simulink model "SimulinkAnalysisofCheetahTail"  (R2022a)
(part 6 of 21)

t4052 = ct{1961};
t4053 = ct{1962};
t4054 = ct{1963};
t4056 = ct{1964};
t4058 = ct{1965};
t4059 = ct{1966};
t4061 = ct{1967};
t4062 = ct{1968};
t4064 = ct{1969};
t4065 = ct{1970};
t4066 = ct{1971};
t4068 = ct{1972};
t4070 = ct{1973};
t4071 = ct{1974};
t4072 = ct{1975};
t4073 = ct{1976};
t4074 = ct{1977};
t4077 = ct{1978};
t4078 = ct{1979};
t4081 = ct{1980};
t4083 = ct{1981};
t4084 = ct{1982};
t4085 = ct{1983};
t4086 = ct{1984};
t4087 = ct{1985};
t4089 = ct{1986};
t4090 = ct{1987};
t4091 = ct{1988};
t4092 = ct{1989};
t4093 = ct{1990};
t4094 = ct{1991};
t4095 = ct{1992};
t4096 = ct{1993};
t4097 = ct{1994};
t4098 = ct{1995};
t4099 = ct{1996};
t410 = ct{1997};
t4100 = ct{1998};
t4104 = ct{1999};
t4105 = ct{2000};
t4107 = ct{2001};
t4108 = ct{2002};
t4109 = ct{2003};
t411 = ct{2004};
t4111 = ct{2005};
t4112 = ct{2006};
t4115 = ct{2007};
t4116 = ct{2008};
t4117 = ct{2009};
t4119 = ct{2010};
t412 = ct{2011};
t4120 = ct{2012};
t4121 = ct{2013};
t4122 = ct{2014};
t4126 = ct{2015};
t4128 = ct{2016};
t4129 = ct{2017};
t413 = ct{2018};
t4130 = ct{2019};
t4131 = ct{2020};
t4132 = ct{2021};
t4133 = ct{2022};
t4135 = ct{2023};
t4137 = ct{2024};
t4138 = ct{2025};
t4139 = ct{2026};
t414 = ct{2027};
t4140 = ct{2028};
t4141 = ct{2029};
t4143 = ct{2030};
t4144 = ct{2031};
t4145 = ct{2032};
t4147 = ct{2033};
t4148 = ct{2034};
t415 = ct{2035};
t4151 = ct{2036};
t4152 = ct{2037};
t4153 = ct{2038};
t4154 = ct{2039};
t4155 = ct{2040};
t4156 = ct{2041};
t4157 = ct{2042};
t4158 = ct{2043};
t4160 = ct{2044};
t4162 = ct{2045};
t4164 = ct{2046};
t4165 = ct{2047};
t4166 = ct{2048};
t4168 = ct{2049};
t4169 = ct{2050};
t4170 = ct{2051};
t4171 = ct{2052};
t4173 = ct{2053};
t4174 = ct{2054};
t4176 = ct{2055};
t4177 = ct{2056};
t4178 = ct{2057};
t4179 = ct{2058};
t4182 = ct{2059};
t4184 = ct{2060};
t4186 = ct{2061};
t4187 = ct{2062};
t4188 = ct{2063};
t4189 = ct{2064};
t4190 = ct{2065};
t4191 = ct{2066};
t4192 = ct{2067};
t4193 = ct{2068};
t4194 = ct{2069};
t4195 = ct{2070};
t4196 = ct{2071};
t4197 = ct{2072};
t420 = ct{2073};
t4200 = ct{2074};
t4201 = ct{2075};
t4202 = ct{2076};
t4203 = ct{2077};
t4204 = ct{2078};
t4205 = ct{2079};
t4206 = ct{2080};
t4208 = ct{2081};
t4209 = ct{2082};
t421 = ct{2083};
t4210 = ct{2084};
t4211 = ct{2085};
t4212 = ct{2086};
t4213 = ct{2087};
t4214 = ct{2088};
t4215 = ct{2089};
t4216 = ct{2090};
t4217 = ct{2091};
t4218 = ct{2092};
t4220 = ct{2093};
t4221 = ct{2094};
t4222 = ct{2095};
t4223 = ct{2096};
t4224 = ct{2097};
t4225 = ct{2098};
t4226 = ct{2099};
t4227 = ct{2100};
t4228 = ct{2101};
t4229 = ct{2102};
t4230 = ct{2103};
t4231 = ct{2104};
t4232 = ct{2105};
t4233 = ct{2106};
t4234 = ct{2107};
t4236 = ct{2108};
t4237 = ct{2109};
t4238 = ct{2110};
t4239 = ct{2111};
t4240 = ct{2112};
t4241 = ct{2113};
t4243 = ct{2114};
t4244 = ct{2115};
t4245 = ct{2116};
t4246 = ct{2117};
t4247 = ct{2118};
t4248 = ct{2119};
t4249 = ct{2120};
t425 = ct{2121};
t4250 = ct{2122};
t4252 = ct{2123};
t4253 = ct{2124};
t4255 = ct{2125};
t4256 = ct{2126};
t4258 = ct{2127};
t4259 = ct{2128};
t4260 = ct{2129};
t4261 = ct{2130};
t4262 = ct{2131};
t4263 = ct{2132};
t4265 = ct{2133};
t4266 = ct{2134};
t4268 = ct{2135};
t4269 = ct{2136};
t4271 = ct{2137};
t4272 = ct{2138};
t4273 = ct{2139};
t4274 = ct{2140};
t4276 = ct{2141};
t4277 = ct{2142};
t4278 = ct{2143};
t4280 = ct{2144};
t4281 = ct{2145};
t4282 = ct{2146};
t4285 = ct{2147};
t4286 = ct{2148};
t4290 = ct{2149};
t4295 = ct{2150};
t4296 = ct{2151};
t4298 = ct{2152};
t430 = ct{2153};
t4300 = ct{2154};
t4301 = ct{2155};
t4302 = ct{2156};
t4303 = ct{2157};
t4304 = ct{2158};
t4305 = ct{2159};
t4306 = ct{2160};
t4307 = ct{2161};
t4308 = ct{2162};
t4309 = ct{2163};
t431 = ct{2164};
t4310 = ct{2165};
t4311 = ct{2166};
t4312 = ct{2167};
t4313 = ct{2168};
t4315 = ct{2169};
t4316 = ct{2170};
t4317 = ct{2171};
t4318 = ct{2172};
t4319 = ct{2173};
t4320 = ct{2174};
t4321 = ct{2175};
t4322 = ct{2176};
t4323 = ct{2177};
t4324 = ct{2178};
t4326 = ct{2179};
t4327 = ct{2180};
t4329 = ct{2181};
t433 = ct{2182};
t4330 = ct{2183};
t4332 = ct{2184};
t4333 = ct{2185};
t4334 = ct{2186};
t4337 = ct{2187};
t4339 = ct{2188};
t4340 = ct{2189};
t4341 = ct{2190};
t4342 = ct{2191};
t4343 = ct{2192};
t4344 = ct{2193};
t4345 = ct{2194};
t4346 = ct{2195};
t4347 = ct{2196};
t4348 = ct{2197};
t4349 = ct{2198};
t4350 = ct{2199};
t4351 = ct{2200};
t4352 = ct{2201};
t4354 = ct{2202};
t4355 = ct{2203};
t4356 = ct{2204};
t4357 = ct{2205};
t4358 = ct{2206};
t4359 = ct{2207};
t436 = ct{2208};
t4360 = ct{2209};
t4361 = ct{2210};
t4362 = ct{2211};
t4364 = ct{2212};
t4365 = ct{2213};
t4367 = ct{2214};
t4368 = ct{2215};
t4370 = ct{2216};
t4371 = ct{2217};
t4372 = ct{2218};
t4373 = ct{2219};
t4374 = ct{2220};
t4375 = ct{2221};
t4376 = ct{2222};
t4377 = ct{2223};
t4378 = ct{2224};
t4379 = ct{2225};
t4380 = ct{2226};
t4382 = ct{2227};
t4383 = ct{2228};
t4384 = ct{2229};
t4385 = ct{2230};
t4386 = ct{2231};
t4387 = ct{2232};
t4388 = ct{2233};
t4389 = ct{2234};
t4392 = ct{2235};
t4393 = ct{2236};
t4394 = ct{2237};
t4395 = ct{2238};
t4396 = ct{2239};
t4399 = ct{2240};
t44 = ct{2241};
t4400 = ct{2242};
t4401 = ct{2243};
t4402 = ct{2244};
t4403 = ct{2245};
t4404 = ct{2246};
t4405 = ct{2247};
t4406 = ct{2248};
t4407 = ct{2249};
t4408 = ct{2250};
t4409 = ct{2251};
t4411 = ct{2252};
t4412 = ct{2253};
t4413 = ct{2254};
t4414 = ct{2255};
t4415 = ct{2256};
t4416 = ct{2257};
t4418 = ct{2258};
t4419 = ct{2259};
t4420 = ct{2260};
t4421 = ct{2261};
t4422 = ct{2262};
t4424 = ct{2263};
t4425 = ct{2264};
t4426 = ct{2265};
t4427 = ct{2266};
t4428 = ct{2267};
t4429 = ct{2268};
t4431 = ct{2269};
t4432 = ct{2270};
t4433 = ct{2271};
t4434 = ct{2272};
t4435 = ct{2273};
t4437 = ct{2274};
t4438 = ct{2275};
t4439 = ct{2276};
t4440 = ct{2277};
t4442 = ct{2278};
t4444 = ct{2279};
t4447 = ct{2280};
t4449 = ct{2281};
t445 = ct{2282};
t4450 = ct{2283};
t4451 = ct{2284};
t4452 = ct{2285};
t4453 = ct{2286};
t4454 = ct{2287};
t4455 = ct{2288};
t4457 = ct{2289};
t4458 = ct{2290};
t4459 = ct{2291};
t4460 = ct{2292};
t4461 = ct{2293};
t4462 = ct{2294};
t4465 = ct{2295};
t4467 = ct{2296};
t4469 = ct{2297};
t4470 = ct{2298};
t4471 = ct{2299};
t4472 = ct{2300};
t4473 = ct{2301};
t4475 = ct{2302};
t4476 = ct{2303};
t4477 = ct{2304};
t4478 = ct{2305};
t4479 = ct{2306};
t4480 = ct{2307};
t4481 = ct{2308};
t4482 = ct{2309};
t4483 = ct{2310};
t4484 = ct{2311};
t4485 = ct{2312};
t4486 = ct{2313};
t4487 = ct{2314};
t4488 = ct{2315};
t4489 = ct{2316};
t4490 = ct{2317};
t4492 = ct{2318};
t4493 = ct{2319};
t4494 = ct{2320};
t4495 = ct{2321};
t4496 = ct{2322};
t4497 = ct{2323};
t4498 = ct{2324};
t4499 = ct{2325};
t4500 = ct{2326};
t4501 = ct{2327};
t4502 = ct{2328};
t4503 = ct{2329};
t4504 = ct{2330};
t4505 = ct{2331};
t4506 = ct{2332};
t4507 = ct{2333};
t451 = ct{2334};
t4511 = ct{2335};
t4512 = ct{2336};
t4514 = ct{2337};
t4515 = ct{2338};
t4517 = ct{2339};
t4518 = ct{2340};
t4519 = ct{2341};
t4520 = ct{2342};
t4521 = ct{2343};
t4522 = ct{2344};
t4523 = ct{2345};
t4524 = ct{2346};
t4525 = ct{2347};
t4526 = ct{2348};
t4528 = ct{2349};
t4529 = ct{2350};
t4530 = ct{2351};
t4531 = ct{2352};
t4532 = ct{2353};
t4533 = ct{2354};
t4534 = ct{2355};
t4536 = ct{2356};
t4537 = ct{2357};
t4538 = ct{2358};
t4541 = ct{2359};
t4542 = ct{2360};
t4545 = ct{2361};
t4546 = ct{2362};
t4547 = ct{2363};
t4548 = ct{2364};
t4549 = ct{2365};
t4550 = ct{2366};
t4551 = ct{2367};
t4552 = ct{2368};
t4553 = ct{2369};
t4555 = ct{2370};
t4556 = ct{2371};
t4557 = ct{2372};
t4558 = ct{2373};
t4559 = ct{2374};
t4560 = ct{2375};
t4561 = ct{2376};
t4562 = ct{2377};
t4563 = ct{2378};
t4566 = ct{2379};
t4567 = ct{2380};
t4569 = ct{2381};
t4570 = ct{2382};
t4571 = ct{2383};
t4572 = ct{2384};
t4573 = ct{2385};
t4574 = ct{2386};
t4575 = ct{2387};
t4576 = ct{2388};
t4577 = ct{2389};
t4578 = ct{2390};
t4580 = ct{2391};
t4581 = ct{2392};
t4583 = ct{2393};
t4584 = ct{2394};
t4585 = ct{2395};
t4587 = ct{2396};
t4588 = ct{2397};
t4589 = ct{2398};
t459 = ct{2399};
t4591 = ct{2400};
t4592 = ct{2401};
t4597 = ct{2402};
t4598 = ct{2403};
t4600 = ct{2404};
t4601 = ct{2405};
t4602 = ct{2406};
t4603 = ct{2407};
t4604 = ct{2408};
t4605 = ct{2409};
t4606 = ct{2410};
t4608 = ct{2411};
t4610 = ct{2412};
t4613 = ct{2413};
t4614 = ct{2414};
t4615 = ct{2415};
t4616 = ct{2416};
t4617 = ct{2417};
t4618 = ct{2418};
t4619 = ct{2419};
t4621 = ct{2420};
t4622 = ct{2421};
t4625 = ct{2422};
t4630 = ct{2423};
t4636 = ct{2424};
t4637 = ct{2425};
t4638 = ct{2426};
t4641 = ct{2427};
t4645 = ct{2428};
t4646 = ct{2429};
t4649 = ct{2430};
t465 = ct{2431};
t4651 = ct{2432};
t4655 = ct{2433};
t4659 = ct{2434};
t4660 = ct{2435};
t4661 = ct{2436};
t4662 = ct{2437};
t4663 = ct{2438};
t4664 = ct{2439};
t4665 = ct{2440};
t4668 = ct{2441};
t4669 = ct{2442};
t4671 = ct{2443};
t4672 = ct{2444};
t4676 = ct{2445};
t4677 = ct{2446};
t4686 = ct{2447};
t4695 = ct{2448};
t4701 = ct{2449};
t4707 = ct{2450};
t4708 = ct{2451};
t4709 = ct{2452};
t4711 = ct{2453};
t4713 = ct{2454};
t4722 = ct{2455};
t4723 = ct{2456};
t4724 = ct{2457};
t4725 = ct{2458};
t4732 = ct{2459};
t4733 = ct{2460};
t4735 = ct{2461};
t4736 = ct{2462};
t4737 = ct{2463};
t4738 = ct{2464};
t4740 = ct{2465};
t4746 = ct{2466};
t4747 = ct{2467};
t4748 = ct{2468};
t4751 = ct{2469};
t4752 = ct{2470};
t4756 = ct{2471};
t4758 = ct{2472};
t4766 = ct{2473};
t4770 = ct{2474};
t4771 = ct{2475};
t4772 = ct{2476};
t4775 = ct{2477};
t4776 = ct{2478};
t4778 = ct{2479};
t4782 = ct{2480};
t4784 = ct{2481};
t4787 = ct{2482};
t4789 = ct{2483};
t4796 = ct{2484};
t48 = ct{2485};
t4800 = ct{2486};
t4801 = ct{2487};
t4802 = ct{2488};
t4805 = ct{2489};
t4807 = ct{2490};
t4809 = ct{2491};
t4821 = ct{2492};
t4823 = ct{2493};
t4830 = ct{2494};
t4834 = ct{2495};
t4837 = ct{2496};
t4842 = ct{2497};
t4846 = ct{2498};
t4847 = ct{2499};
t4848 = ct{2500};
t4849 = ct{2501};
t485 = ct{2502};
t4859 = ct{2503};
t4862 = ct{2504};
t4864 = ct{2505};
t4870 = ct{2506};
t4871 = ct{2507};
t4873 = ct{2508};
t4874 = ct{2509};
t4877 = ct{2510};
t4878 = ct{2511};
t488 = ct{2512};
t4880 = ct{2513};
t4882 = ct{2514};
t4883 = ct{2515};
t4889 = ct{2516};
t4890 = ct{2517};
t4892 = ct{2518};
t4895 = ct{2519};
t4897 = ct{2520};
t49 = ct{2521};
t4904 = ct{2522};
t4908 = ct{2523};
t4909 = ct{2524};
t491 = ct{2525};
t4912 = ct{2526};
t4913 = ct{2527};
t4922 = ct{2528};
t4923 = ct{2529};
t4925 = ct{2530};
t4927 = ct{2531};
t4931 = ct{2532};
t4932 = ct{2533};
t4933 = ct{2534};
t4934 = ct{2535};
t4936 = ct{2536};
t4938 = ct{2537};
t4939 = ct{2538};
t4941 = ct{2539};
t4942 = ct{2540};
t4944 = ct{2541};
t4945 = ct{2542};
t4946 = ct{2543};
t4949 = ct{2544};
t4950 = ct{2545};
t4953 = ct{2546};
t4954 = ct{2547};
t496 = ct{2548};
t4960 = ct{2549};
t4961 = ct{2550};
t4964 = ct{2551};
t4966 = ct{2552};
t4967 = ct{2553};
t4968 = ct{2554};
t4969 = ct{2555};
t4975 = ct{2556};
t4976 = ct{2557};
t4978 = ct{2558};
t4979 = ct{2559};
t4986 = ct{2560};
t4987 = ct{2561};
t4988 = ct{2562};
t4990 = ct{2563};
t4991 = ct{2564};
t4992 = ct{2565};
t4993 = ct{2566};
t4995 = ct{2567};
t4997 = ct{2568};
t4998 = ct{2569};
t5 = ct{2570};
t50 = ct{2571};
t5004 = ct{2572};
t501 = ct{2573};
t5017 = ct{2574};
t502 = ct{2575};
t5020 = ct{2576};
t5021 = ct{2577};
t5024 = ct{2578};
t5029 = ct{2579};
t5030 = ct{2580};
t5031 = ct{2581};
t5032 = ct{2582};
t5033 = ct{2583};
t5036 = ct{2584};
t5038 = ct{2585};
t504 = ct{2586};
t5041 = ct{2587};
t5042 = ct{2588};
t5046 = ct{2589};
t5048 = ct{2590};
t5051 = ct{2591};
t5053 = ct{2592};
t5054 = ct{2593};
t5055 = ct{2594};
t5058 = ct{2595};
t5059 = ct{2596};
t5061 = ct{2597};
t5063 = ct{2598};
t5066 = ct{2599};
t5067 = ct{2600};
t5072 = ct{2601};
t5074 = ct{2602};
t5076 = ct{2603};
t5078 = ct{2604};
t5080 = ct{2605};
t5082 = ct{2606};
t5083 = ct{2607};
t5088 = ct{2608};
t5092 = ct{2609};
t5098 = ct{2610};
t5099 = ct{2611};
t51 = ct{2612};
t5103 = ct{2613};
t5109 = ct{2614};
t5114 = ct{2615};
t5126 = ct{2616};
t5128 = ct{2617};
t5131 = ct{2618};
t5143 = ct{2619};
t5150 = ct{2620};
t5152 = ct{2621};
t5153 = ct{2622};
t5156 = ct{2623};
t5161 = ct{2624};
t5165 = ct{2625};
t5177 = ct{2626};
t5179 = ct{2627};
t5184 = ct{2628};
t519 = ct{2629};
t5191 = ct{2630};
t5194 = ct{2631};
t5197 = ct{2632};
t5198 = ct{2633};
t5202 = ct{2634};
t5203 = ct{2635};
t5205 = ct{2636};
t5206 = ct{2637};
t5207 = ct{2638};
t5208 = ct{2639};
t5214 = ct{2640};
t5223 = ct{2641};
t5227 = ct{2642};
t523 = ct{2643};
t5232 = ct{2644};
t524 = ct{2645};
t5240 = ct{2646};
t5241 = ct{2647};
t5265 = ct{2648};
t527 = ct{2649};
t5275 = ct{2650};
t5287 = ct{2651};
t5291 = ct{2652};
t5293 = ct{2653};
t530 = ct{2654};
t5300 = ct{2655};
t5308 = ct{2656};
t5310 = ct{2657};
t5317 = ct{2658};
t5319 = ct{2659};
t5324 = ct{2660};
t5328 = ct{2661};
t534 = ct{2662};
t5344 = ct{2663};
t5351 = ct{2664};
t5354 = ct{2665};
t5358 = ct{2666};
t5363 = ct{2667};
t537 = ct{2668};
t5372 = ct{2669};
t5374 = ct{2670};
t5379 = ct{2671};
t5380 = ct{2672};
t539 = ct{2673};
t5399 = ct{2674};
t54 = ct{2675};
t541 = ct{2676};
t5412 = ct{2677};
t5417 = ct{2678};
t542 = ct{2679};
t5420 = ct{2680};
t5424 = ct{2681};
t5427 = ct{2682};
t5431 = ct{2683};
t5438 = ct{2684};
t544 = ct{2685};
t5445 = ct{2686};
t5448 = ct{2687};
t5452 = ct{2688};
t5453 = ct{2689};
t5456 = ct{2690};
t546 = ct{2691};
t5460 = ct{2692};
t5476 = ct{2693};
t5488 = ct{2694};
t5490 = ct{2695};
t5492 = ct{2696};
t5493 = ct{2697};
t5494 = ct{2698};
t5498 = ct{2699};
t55 = ct{2700};
t550 = ct{2701};
t5523 = ct{2702};
t5524 = ct{2703};
t553 = ct{2704};
t5530 = ct{2705};
t5538 = ct{2706};
t5539 = ct{2707};
t5547 = ct{2708};
t5548 = ct{2709};
t5552 = ct{2710};
t5556 = ct{2711};
t5565 = ct{2712};
t5566 = ct{2713};
t5569 = ct{2714};
t557 = ct{2715};
t5576 = ct{2716};
t558 = ct{2717};
t5582 = ct{2718};
t5588 = ct{2719};
t5598 = ct{2720};
t56 = ct{2721};
t5607 = ct{2722};
t5620 = ct{2723};
t5657 = ct{2724};
t5660 = ct{2725};
t5662 = ct{2726};
t5664 = ct{2727};
t5668 = ct{2728};
t5672 = ct{2729};
t5674 = ct{2730};
t5685 = ct{2731};
t5690 = ct{2732};
t5696 = ct{2733};
t5697 = ct{2734};
t5705 = ct{2735};
t5706 = ct{2736};
t5713 = ct{2737};
t5724 = ct{2738};
t573 = ct{2739};
t5730 = ct{2740};
t5738 = ct{2741};
t574 = ct{2742};
t5749 = ct{2743};
t575 = ct{2744};
t5757 = ct{2745};
t5779 = ct{2746};
t5785 = ct{2747};
t5788 = ct{2748};
t5791 = ct{2749};
t5795 = ct{2750};
t5798 = ct{2751};
t5800 = ct{2752};
t5806 = ct{2753};
t5808 = ct{2754};
t5809 = ct{2755};
t5815 = ct{2756};
t5832 = ct{2757};
t5837 = ct{2758};
t5840 = ct{2759};
t5843 = ct{2760};
t5846 = ct{2761};
t5857 = ct{2762};
t5867 = ct{2763};
t5869 = ct{2764};
t587 = ct{2765};
t5870 = ct{2766};
t5874 = ct{2767};
t5880 = ct{2768};
t5887 = ct{2769};
t59 = ct{2770};
t5905 = ct{2771};
t5926 = ct{2772};
t5932 = ct{2773};
t5933 = ct{2774};
t5936 = ct{2775};
t5939 = ct{2776};
t5949 = ct{2777};
t595 = ct{2778};
t5963 = ct{2779};
t5971 = ct{2780};
t5984 = ct{2781};
t5985 = ct{2782};
t603 = ct{2783};
t6049 = ct{2784};
t6051 = ct{2785};
t6052 = ct{2786};
t6066 = ct{2787};
t6067 = ct{2788};
t6074 = ct{2789};
t6083 = ct{2790};
t6099 = ct{2791};
t61 = ct{2792};
t6117 = ct{2793};
t6129 = ct{2794};
t614 = ct{2795};
t628 = ct{2796};
t629 = ct{2797};
t634 = ct{2798};
t641 = ct{2799};
t65 = ct{2800};
t650 = ct{2801};
t651 = ct{2802};
t655 = ct{2803};
t6555 = ct{2804};
t6557 = ct{2805};
t657 = ct{2806};
t6599 = ct{2807};
t6628 = ct{2808};
t6629 = ct{2809};
t664 = ct{2810};
t665 = ct{2811};
t666 = ct{2812};
t667 = ct{2813};
t668 = ct{2814};
t669 = ct{2815};
t675 = ct{2816};
t68 = ct{2817};
t693 = ct{2818};
t7 = ct{2819};
t71 = ct{2820};
t721 = ct{2821};
t724 = ct{2822};
t73 = ct{2823};
t731 = ct{2824};
t732 = ct{2825};
t736 = ct{2826};
t741 = ct{2827};
t753 = ct{2828};
t754 = ct{2829};
t755 = ct{2830};
t756 = ct{2831};
t757 = ct{2832};
t759 = ct{2833};
t760 = ct{2834};
t761 = ct{2835};
t762 = ct{2836};
t764 = ct{2837};
t765 = ct{2838};
t769 = ct{2839};
t772 = ct{2840};
t774 = ct{2841};
t776 = ct{2842};
t778 = ct{2843};
t795 = ct{2844};
t797 = ct{2845};
t799 = ct{2846};
t8 = ct{2847};
t802 = ct{2848};
t803 = ct{2849};
t806 = ct{2850};
t817 = ct{2851};
t818 = ct{2852};
t820 = ct{2853};
t824 = ct{2854};
t828 = ct{2855};
t831 = ct{2856};
t838 = ct{2857};
t843 = ct{2858};
t844 = ct{2859};
t846 = ct{2860};
t847 = ct{2861};
t848 = ct{2862};
t850 = ct{2863};
t851 = ct{2864};
t852 = ct{2865};
t853 = ct{2866};
t855 = ct{2867};
t865 = ct{2868};
t867 = ct{2869};
t868 = ct{2870};
t870 = ct{2871};
t871 = ct{2872};
t872 = ct{2873};
t876 = ct{2874};
t877 = ct{2875};
t886 = ct{2876};
t888 = ct{2877};
t890 = ct{2878};
t896 = ct{2879};
t9 = ct{2880};
t901 = ct{2881};
t902 = ct{2882};
t903 = ct{2883};
t904 = ct{2884};
t906 = ct{2885};
t907 = ct{2886};
t909 = ct{2887};
t914 = ct{2888};
t916 = ct{2889};
t924 = ct{2890};
t925 = ct{2891};
t926 = ct{2892};
t947 = ct{2893};
t949 = ct{2894};
t952 = ct{2895};
t954 = ct{2896};
t955 = ct{2897};
t957 = ct{2898};
t964 = ct{2899};
t972 = ct{2900};
t977 = ct{2901};
t983 = ct{2902};
t987 = ct{2903};
t991 = ct{2904};
t992 = ct{2905};
t993 = ct{2906};
t994 = ct{2907};
t995 = ct{2908};
t4620 = Mt.*t3774.*t4115;
t4623 = t4528.*3.36554e-3;
t4624 = Mt.*t3774.*t4132;
t4626 = t4415.*(t197-t537).*(-3.36554e-3);
t4629 = t1884+t1893+t2128+t2200;
t4634 = t3997+t4031;
t4639 = t4435.*(t103-t544).*(-3.36554e-3);
t4647 = t4542.*3.36554e-3;
t4652 = t4550.*3.36554e-3;
t4653 = Mt.*t2730.*t4357;
t4657 = t2048+t2074+t2079+t2138;
t4666 = Mt.*t2914.*t4357;
t4667 = t1967+t2127+t2173+t2198;
t4670 = t1845+t1864+t2451+t2502;
t4673 = -t4664;
t4674 = Mt.*t4357.*(-t130+t436+t523-t657+t769);
t4675 = t1849+t1870+t2416+t2610;
t4678 = -t4671;
t4681 = t2214+t3352+t3479;
t4682 = dth2.*t4676;
t4683 = dth2.*t4677;
t4684 = dy.*t4677;
t4685 = dz.*t4676;
t4687 = t4576.*3.36554e-3;
t4697 = t4589.*3.36554e-3;
t4698 = t4591.*3.36554e-3;
t4700 = ITail.*t3967.*t4214;
t4702 = ITail.*t3961.*t4215;
t4704 = t2620+t3425+t3455;
t4705 = t4589.*9.52624335e-4;
t4706 = t4589.*3.372816795e-3;
t4710 = ITail.*t4071.*t4162;
t4712 = t1020+t1117+t1606+t1632+t1844+t1869;
t4717 = t1124+t1163+t1609+t1686+t1853+t1858;
t4720 = Mt.*t3679.*t4357;
t4728 = t916+t1143+t1544+t1614+t2038+t2175;
t4729 = -t4725;
t4742 = ITail.*t4164.*t4214;
t4749 = t754+t1174+t1220+t1635+t2544+t2676;
t4750 = -ITail.*t4215.*(-t1262+t1701+t9.*t868.*(t105-t465));
t4753 = t2880+t3626+t3763;
t4754 = dphi2.*t4748;
t4755 = dth2.*t4748;
t4757 = t1163+t1243+t1785+t1823+t1853+t1858;
t4759 = -ITail.*t4162.*(-t1355+t1789+(t9.*t868.*(t105-t465))./2.0);
t4761 = Mt.*t3969.*t4357;
t4764 = ITail.*t4214.*t4237;
t4767 = t954+t1156+t1730+t1792+t2093+t2139;
t4768 = -ITail.*t4215.*(-t947+t1240.*(t105-t465)+t903.*(t534-t546));
t4769 = ITail.*t4215.*t4255;
t4773 = ITail.*t4215.*(-t947+t1240.*(t105-t465)+t903.*(t534-t546));
t4777 = -ITail.*t4162.*(-t1017+(t1240.*(t105-t465))./2.0+(t903.*(t534-t546))./2.0);
t4780 = ITail.*t4162.*t4296;
t4781 = ITail.*t4214.*t4277;
t4783 = t1140+t1354+t1610+t1631+t2212+t2243;
t4785 = t2529+t2635+t2641+t2741;
t4786 = dz.*t4778;
t4788 = ITail.*t4162.*(-t1017+(t1240.*(t105-t465))./2.0+(t903.*(t534-t546))./2.0);
t4790 = dy.*t4782;
t4798 = t1079+t1122+t1924+t1956+t2003+t2005;
t4799 = Mt.*t4100.*t4357;
t4803 = -ITail.*t3967.*(t1386+t2501+(t1512.*(t105-t465))./2.0);
t4806 = -t4801;
t4808 = t1121+t1183+t1883+t1997+t2000+t2026;
t4810 = ITail.*t4214.*t4313;
t4811 = ITail.*t4215.*t4311;
t4812 = t1251+t1829+t1863+t4313;
t4815 = ITail.*t4162.*t4343;
t4816 = t1357+t1386+t1644+t1649+t2213+t2244;
t4820 = t987+t1753+t1762+t4396;
t4826 = ITail.*t4296.*t4313;
t4829 = -ITail.*t4214.*(t1260-t2364+t1430.*(t105-t465));
t4831 = ITail.*t4215.*t4382;
t4832 = ITail.*t4214.*(t1260-t2364+t1430.*(t105-t465));
t4836 = ITail.*t4277.*t4343;
t4838 = t3967.*t4500;
t4841 = -ITail.*t4215.*(t1332+t2368+t1512.*(t105-t465));
t4843 = t3961.*t4505;
t4844 = ITail.*t4162.*t4416;
t4845 = -ITail.*t4214.*(-t1331+t2317+t1510.*(t103-t544));
t4850 = dy.*t4842;
t4851 = dphi2.*t4837;
t4852 = dth2.*t4837;
t4853 = -ITail.*t4162.*(t1386+t2501+(t1512.*(t105-t465))./2.0);
t4855 = -ITail.*t4164.*(t1386+t2501+(t1512.*(t105-t465))./2.0);
t4856 = t1354+t1358+t1872+t1922+t2212+t2243;
t4858 = t2957+t4011+t4030;
t4865 = ITail.*t4164.*(t1386+t2501+(t1512.*(t105-t465))./2.0);
t4867 = t1082+t1847+t1852+t4426;
t4879 = t844+t1361+t1423+t1711+t3099+t3168;
t4881 = t2867+t2971+t3000+t3003;
t4884 = -t4877;
t4888 = -ITail.*t4237.*(t1386+t2501+(t1512.*(t105-t465))./2.0);
t4891 = t1189+t1248+t2205+t2210+t2279+t2284;
t4896 = t2274+t4128+t4131;
t4900 = t1478+t1555+t1940+t1986+t2195+t2234;
t4901 = ITail.*t4214.*t4454;
t4902 = -ITail.*t4296.*(-t1331+t2317+t1510.*(t103-t544));
t4903 = ITail.*t4277.*t4416;
t4906 = ITail.*t4296.*(-t1331+t2317+t1510.*(t103-t544));
t4911 = t4164.*t4500;
t4914 = -t4505.*(-t1262+t1701+t9.*t868.*(t105-t465));
t4915 = ITail.*t4313.*t4416;
t4919 = -ITail.*t4214.*(-t1018+t1426+t1431-t1446+t3.*t496.*(t105-t465));
t4920 = -ITail.*t4343.*(-t1331+t2317+t1510.*(t103-t544));
t4924 = ITail.*t4214.*(-t1018+t1426+t1431-t1446+t3.*t496.*(t105-t465));
t4926 = ITail.*t4343.*(-t1331+t2317+t1510.*(t103-t544));
t4928 = t1399+t1553+t2235+t2246+t2250+t2332;
t4929 = t4237.*t4500;
t4935 = -t4505.*(-t947+t1240.*(t105-t465)+t903.*(t534-t546));
t4937 = t4505.*(-t947+t1240.*(t105-t465)+t903.*(t534-t546));
t4940 = t4162.*t4551;
t4943 = t4255.*t4518;
t4947 = ITail.*t3961.*t4617;
t4948 = t4277.*t4517;
t4963 = -ITail.*t4392.*(t1368-t2524+t1430.*(t197-t537));
t4972 = t1368+t1380+t2453+t2460+t2549+t2558;
t4973 = dphi2.*t4968;
t4974 = t4313.*t4517;
t4977 = t4311.*t4518;
t4980 = t3181+t3189+t3464+t3496;
t4982 = ITail.*t4071.*t4638;
t4983 = dphi2.*t4979;
t4989 = t3240+t3370+t3408+t3410;
t4994 = t3069+t3102+t3601+t3635;
t4996 = ITail.*t4214.*t4581;
t4999 = -t4992;
t5000 = -ITail.*t4447.*(t1368-t2524+t1430.*(t197-t537));
t5002 = ITail.*t4392.*t4461;
t5005 = -t4162.*(-t2388+t3008+t9.*t868.*(t105-t465).*9.53094055e-4);
t5006 = t3361+t3393+t3420+t3430;
t5007 = -ITail.*t4214.*(t1019-t1651+t1702+t3.*t818.*(t105-t465)+t3.*t872.*(t103-t544));
t5008 = -ITail.*t4454.*(t1386+t2501+(t1512.*(t105-t465))./2.0);
t5009 = -ITail.*t4452.*(t1396-t2573+t1430.*(t197-t537).*2.0);
t5010 = ITail.*t4214.*(t1019-t1651+t1702+t3.*t818.*(t105-t465)+t3.*t872.*(t103-t544));
t5011 = -t4500.*(t1260-t2364+t1430.*(t105-t465));
t5012 = -ITail.*t4617.*(-t1262+t1701+t9.*t868.*(t105-t465));
t5014 = -ITail.*t4392.*(t1365-t2831+t1505.*(t534-t546));
t5016 = t4500.*(t1260-t2364+t1430.*(t105-t465));
t5018 = -t4505.*(t1332+t2368+t1512.*(t105-t465));
t5019 = ITail.*t4071.*t4672;
t5022 = t1617+t1653+t2439+t2445+t2554+t2561;
t5023 = t3115+t3157+t3658+t3790;
t5026 = t4382.*t4518;
t5027 = -t5020;
t5039 = -t5029;
t5040 = -t4517.*(-t1331+t2317+t1510.*(t103-t544));
t5043 = -t4162.*(-t1974+t1240.*(t105-t465).*9.53094055e-4+t903.*(t534-t546).*9.53094055e-4);
t5047 = ITail.*(t1386+t2501+(t1512.*(t105-t465))./2.0).*(-t1018+t1426+t1431-t1446+t3.*t496.*(t105-t465));
t5050 = ITail.*t4447.*t4461;
t5052 = t4162.*(-t1974+t1240.*(t105-t465).*9.53094055e-4+t903.*(t534-t546).*9.53094055e-4);
t5057 = -ITail.*t4617.*(-t947+t1240.*(t105-t465)+t903.*(t534-t546));
t5060 = ITail.*t4452.*t4471;
t5062 = t4162.*t4668;
t5064 = -ITail.*t4638.*(-t1355+t1789+(t9.*t868.*(t105-t465))./2.0);
t5073 = -ITail.*t4447.*(t1365-t2831+t1505.*(t534-t546));
t5077 = -t3967.*(-t2389+t3634+t1512.*(t105-t465).*9.53094055e-4);
t5081 = t1306+t1465+t2639+t2640+t2940+t2997;
t5084 = ITail.*t4447.*(t1365-t2831+t1505.*(t534-t546));
t5085 = -ITail.*t4452.*(t1395-t2868+t1505.*(t534-t546).*2.0);
t5090 = t4454.*t4500;
t5093 = -ITail.*t4522.*(t1396-t2573+t1430.*(t197-t537).*2.0);
t5095 = ITail.*t4214.*t4672;
t5101 = ITail.*t4214.*t4686;
t5102 = -ITail.*t4638.*(-t1017+(t1240.*(t105-t465))./2.0+(t903.*(t534-t546))./2.0);
t5104 = -t5099;
t5111 = t4162.*t4701;
t5112 = -ITail.*t4672.*(-t1355+t1789+(t9.*t868.*(t105-t465))./2.0);
t5113 = t1443+t2833+t2905+t4494;
t5120 = -ITail.*t4215.*(t995+t1064-t1506+t1598-t1763-t1774);
t5121 = ITail.*t4214.*t4695;
t5123 = ITail.*t4392.*t4573;
t5129 = -t4500.*(-t1018+t1426+t1431-t1446+t3.*t496.*(t105-t465));
t5133 = -ITail.*t4215.*(t820+t1121-t1435+t1997+t2000+t11.*t420.*(t214-t541));
t5135 = t4500.*(-t1018+t1426+t1431-t1446+t3.*t496.*(t105-t465));
t5136 = ITail.*t4471.*t4522;
t5137 = -ITail.*t4214.*(t1260-t1328-t1427-t1441+t1706+t9.*t870.*(t105-t465));
t5139 = ITail.*t4215.*(t820+t1121-t1435+t1997+t2000+t11.*t420.*(t214-t541));
t5144 = ITail.*t4214.*(t1260-t1328-t1427-t1441+t1706+t9.*t870.*(t105-t465));
t5146 = ITail.*t4408.*t4573;
t5149 = -ITail.*t4162.*(t1088+t1147-t1609+t1652-t1853-t1858);
t5151 = -ITail.*t4522.*(t1395-t2868+t1505.*(t534-t546).*2.0);
t5154 = -ITail.*t4575.*(t1386+t2501+(t1512.*(t105-t465))./2.0);
t5155 = -t4162.*(-t2389+t3634+t1512.*(t105-t465).*9.53094055e-4);
t5158 = t4313.*t4668;
t5160 = -t4164.*(-t2389+t3634+t1512.*(t105-t465).*9.53094055e-4);
t5163 = ITail.*t4522.*(t1395-t2868+t1505.*(t534-t546).*2.0);
t5164 = -ITail.*t4581.*(t1386+t2501+(t1512.*(t105-t465))./2.0);
t5166 = t4164.*(-t2389+t3634+t1512.*(t105-t465).*9.53094055e-4);
t5167 = t4277.*t4701;
t5171 = -ITail.*t4617.*(t1332+t2368+t1512.*(t105-t465));
t5172 = ITail.*t4581.*(t1386+t2501+(t1512.*(t105-t465))./2.0);
t5173 = -ITail.*t4214.*(t753+t991-t1771-t1957+t1181.*(t105-t465)+t11.*t381.*(t534-t546));
t5174 = ITail.*t4447.*t4573;
t5176 = t4162.*t4736;
t5178 = ITail.*(t1386+t2501+(t1512.*(t105-t465))./2.0).*(t1019-t1651+t1702+t3.*t818.*(t105-t465)+t3.*t872.*(t103-t544));
t5181 = -ITail.*t4215.*(t1064+t1137-t1694+t1698-t1763-t1774);
t5182 = -ITail.*t4592.*(-t1412+t2419+(t1510.*(t103-t544))./2.0);
t5185 = -ITail.*t4077.*(t2436-t2536+t1510.*(t197-t537)+t1505.*(t214-t541));
t5190 = ITail.*t4215.*(t1064+t1137-t1694+t1698-t1763-t1774);
t5193 = -t5184;
t5199 = -t4237.*(-t2389+t3634+t1512.*(t105-t465).*9.53094055e-4);
t5204 = -ITail.*t4215.*(t867+t1059-t1646-t1705+t1938-t2002);
t5210 = -ITail.*t4618.*(-t1412+t2419+(t1510.*(t103-t544))./2.0);
t5213 = -ITail.*t4162.*(t1147+t1193-t1785+t1787-t1853-t1858);
t5215 = ITail.*t4215.*t4738;
t5217 = -ITail.*t4638.*(t1386+t2501+(t1512.*(t105-t465))./2.0);
t5218 = ITail.*t4618.*(-t1412+t2419+(t1510.*(t103-t544))./2.0);
t5220 = ITail.*t4162.*(t1147+t1193-t1785+t1787-t1853-t1858);
t5224 = ITail.*t4071.*(t1079+t1956-t4277-t1178.*(t105-t465));
t5225 = ITail.*t4476.*t4573;
t5229 = ITail.*(t1386+t2501+(t1512.*(t105-t465))./2.0).*(t1751+t2308+t964.*(t105-t465)+t1430.*(t103-t544));
t5236 = -t4668.*(-t1331+t2317+t1510.*(t103-t544));
t5237 = t4277.*t4736;
t5238 = -ITail.*t4645.*(-t1412+t2419+(t1510.*(t103-t544))./2.0);
t5239 = -ITail.*t4162.*(t949+t1142-t1730-t1792+t2049-t2139);
t5244 = t4668.*(-t1331+t2317+t1510.*(t103-t544));
t5246 = t4500.*t4581;
t5250 = -ITail.*t4313.*(t1088+t1147-t1609+t1652-t1853-t1858);
t5251 = -ITail.*t4071.*(t1185+t1813-t4313+t1047.*(t105-t465));
t5256 = -t4500.*(t1019-t1651+t1702+t3.*t818.*(t105-t465)+t3.*t872.*(t103-t544));
t5263 = t4500.*(t1019-t1651+t1702+t3.*t818.*(t105-t465)+t3.*t872.*(t103-t544));
t5266 = ITail.*t4215.*t4770;
t5268 = -ITail.*t4672.*(t1386+t2501+(t1512.*(t105-t465))./2.0);
t5271 = t4313.*t4736;
t5272 = -ITail.*t4277.*(t1147+t1193-t1785+t1787-t1853-t1858);
t5274 = ITail.*t4077.*t4821;
t5280 = -ITail.*t4686.*(t1386+t2501+(t1512.*(t105-t465))./2.0);
t5282 = -t4701.*(-t1331+t2317+t1510.*(t103-t544));
t5285 = ITail.*t4686.*(t1386+t2501+(t1512.*(t105-t465))./2.0);
t5286 = t4701.*(-t1331+t2317+t1510.*(t103-t544));
t5288 = ITail.*t4077.*t4823;
t5289 = -ITail.*t4695.*(t1386+t2501+(t1512.*(t105-t465))./2.0);
t5290 = ITail.*t4214.*(t1079+t1956-t4277-t1178.*(t105-t465));
t5294 = ITail.*t3938.*t4874;
t5299 = ITail.*t4695.*(t1386+t2501+(t1512.*(t105-t465))./2.0);
t5301 = ITail.*t4077.*t4830;
t5302 = -ITail.*t4077.*(-t1129+t1139-t2082+t2110+t2123+t8.*t872.*(t534-t546));
t5304 = t1975+t2095+t2769+t2807+t3065+t3104;
t5306 = ITail.*t3938.*t4882;
t5309 = ITail.*(-t1412+t2419+(t1510.*(t103-t544))./2.0).*(t820+t1121-t1435+t1997+t2000+t11.*t420.*(t214-t541));
t5311 = -ITail.*t4215.*(t1060+t1138-t1883+t1932+t2088+t1179.*(t103-t544));
t5312 = -ITail.*(-t1355+t1789+(t9.*t868.*(t105-t465))./2.0).*(t1079+t1956-t4277-t1178.*(t105-t465));
t5313 = t3844+t3884+t3901+t3910;
t5316 = ITail.*(t1386+t2501+(t1512.*(t105-t465))./2.0).*(t1260-t1328-t1427-t1441+t1706+t9.*t870.*(t105-t465));
t5318 = ITail.*t4077.*t4834;
t5320 = -ITail.*t4214.*(t1185+t1813-t4313+t1047.*(t105-t465));
t5321 = -t5308;
t5325 = ITail.*(-t1331+t2317+t1510.*(t103-t544)).*(t1088+t1147-t1609+t1652-t1853-t1858);
t5326 = ITail.*t4214.*(t1185+t1813-t4313+t1047.*(t105-t465));
t5327 = ITail.*t4077.*t4849;
t5329 = -ITail.*t4313.*(t949+t1142-t1730-t1792+t2049-t2139);
t5334 = t1073+t1946+t1949+t2425+t3970+t3987;
t5335 = ITail.*(-t1355+t1789+(t9.*t868.*(t105-t465))./2.0).*(t1185+t1813-t4313+t1047.*(t105-t465));
t5336 = -ITail.*t4215.*(t1250-t1261+t1761-t2083-t2111+t1037.*(t103-t544));
t5338 = ITail.*t3938.*t4908;
t5340 = t4500.*t4672;
t5345 = -ITail.*t4215.*(t1053+t1332+t2368+t817.*(t214-t541)+t977.*(t103-t544)+t1512.*(t105-t465));
t5346 = -ITail.*t4162.*(t1143+t1194-t1959+t2038+t2175+(t1179.*(t103-t544))./2.0);
t5347 = ITail.*(t1386+t2501+(t1512.*(t105-t465))./2.0).*(t753+t991-t1771-t1957+t1181.*(t105-t465)+t11.*t381.*(t534-t546));
t5348 = t1132+t1902+t2010+t2521+t3941+t4015;
t5349 = -ITail.*(-t1017+(t1240.*(t105-t465))./2.0+(t903.*(t534-t546))./2.0).*(t1079+t1956-t4277-t1178.*(t105-t465));
t5352 = t4500.*t4686;
t5353 = t4551.*t4638;
t5356 = -t4392.*(t2591-t3773+t1430.*(t197-t537).*1.90524867e-3);
t5364 = t4500.*t4695;
t5367 = t2176+t2259+t2825+t2944+t3121+t3131;
t5368 = ITail.*t4077.*t4897;
t5369 = -ITail.*t4162.*(t1334-t1354+t1851-t2212-t2243+(t1037.*(t103-t544))./2.0);
t5370 = ITail.*(-t1017+(t1240.*(t105-t465))./2.0+(t903.*(t534-t546))./2.0).*(t1185+t1813-t4313+t1047.*(t105-t465));
t5378 = -t4454.*(-t2389+t3634+t1512.*(t105-t465).*9.53094055e-4);
t5382 = ITail.*(-t1331+t2317+t1510.*(t103-t544)).*(t1147+t1193-t1785+t1787-t1853-t1858);
t5384 = -ITail.*t4162.*(t1141+t1386+t2501+(t817.*(t214-t541))./2.0+(t977.*(t103-t544))./2.0+(t1512.*(t105-t465))./2.0);
t5385 = -t5372;
t5386 = -t4518.*(t995+t1064-t1506+t1598-t1763-t1774);
t5391 = -t4737.*(t1396-t2573+t1430.*(t197-t537).*2.0);
t5392 = t1914+t2208+t2775+t2835+t3347+t3475;
t5393 = -t4500.*(t1260-t1328-t1427-t1441+t1706+t9.*t870.*(t105-t465));
t5396 = -ITail.*t4738.*(-t1412+t2419+(t1510.*(t103-t544))./2.0);
t5397 = -t4518.*(t820+t1121-t1435+t1997+t2000+t11.*t420.*(t214-t541));
t5398 = t4500.*(t1260-t1328-t1427-t1441+t1706+t9.*t870.*(t105-t465));
t5401 = t4551.*t4672;
t5404 = -ITail.*t4277.*(t1143+t1194-t1959+t2038+t2175+(t1179.*(t103-t544))./2.0);
t5405 = ITail.*(-t1331+t2317+t1510.*(t103-t544)).*(t949+t1142-t1730-t1792+t2049-t2139);
t5406 = t4518.*(t820+t1121-t1435+t1997+t2000+t11.*t420.*(t214-t541));
t5407 = -t4447.*(t2591-t3773+t1430.*(t197-t537).*1.90524867e-3);
t5409 = t4392.*t4775;
t5413 = ITail.*t4277.*(t1143+t1194-t1959+t2038+t2175+(t1179.*(t103-t544))./2.0);
t5419 = -t4500.*(t753+t991-t1771-t1957+t1181.*(t105-t465)+t11.*t381.*(t534-t546));
t5421 = ITail.*t4077.*t4922;
t5422 = -t4392.*(t2587-t3868+t1505.*(t534-t546).*1.90524867e-3);
t5423 = (-t2389+t3634+t1512.*(t105-t465).*9.53094055e-4).*(-t1018+t1426+t1431-t1446+t3.*t496.*(t105-t465));
t5425 = ITail.*t4077.*t4923;
t5428 = -ITail.*t4277.*(t1334-t1354+t1851-t2212-t2243+(t1037.*(t103-t544))./2.0);
t5429 = t4408.*t4775;
t5430 = t3961.*t4949;
t5432 = t2259+t2342+t3054+t3096+t3121+t3131;
t5435 = ITail.*t3938.*t4960;
t5437 = t4471.*t4737;
t5439 = ITail.*t3938.*t4961;
t5441 = -ITail.*t4313.*(t1143+t1194-t1959+t2038+t2175+(t1179.*(t103-t544))./2.0);
t5443 = -ITail.*t4452.*(t2436-t2536+t1510.*(t197-t537)+t1505.*(t214-t541));
t5444 = -ITail.*t4277.*(t1141+t1386+t2501+(t817.*(t214-t541))./2.0+(t977.*(t103-t544))./2.0+(t1512.*(t105-t465))./2.0);
t5446 = -ITail.*t4770.*(-t1412+t2419+(t1510.*(t103-t544))./2.0);
t5447 = -t4638.*(-t2388+t3008+t9.*t868.*(t105-t465).*9.53094055e-4);
t5451 = -t4518.*(t1064+t1137-t1694+t1698-t1763-t1774);
t5455 = ITail.*t4770.*(-t1412+t2419+(t1510.*(t103-t544))./2.0);
t5457 = t1960+t2254+t2994+t3064+t3407+t3431;
t5458 = t4518.*(t1064+t1137-t1694+t1698-t1763-t1774);
t5459 = -t4737.*(t1395-t2868+t1505.*(t534-t546).*2.0);
t5461 = t4447.*t4775;
t5463 = -t4518.*(t867+t1059-t1646-t1705+t1938-t2002);
t5464 = -t4787.*(t1396-t2573+t1430.*(t197-t537).*2.0);
t5466 = -ITail.*t4313.*(t1334-t1354+t1851-t2212-t2243+(t1037.*(t103-t544))./2.0);
t5470 = ITail.*t4313.*(t1334-t1354+t1851-t2212-t2243+(t1037.*(t103-t544))./2.0);
t5472 = -t4447.*(t2587-t3868+t1505.*(t534-t546).*1.90524867e-3);
t5473 = -ITail.*t4313.*(t1141+t1386+t2501+(t817.*(t214-t541))./2.0+(t977.*(t103-t544))./2.0+(t1512.*(t105-t465))./2.0);
t5474 = t2201+t2514+t2828+t2848+t3501+t3510;
t5475 = -t4638.*(-t1974+t1240.*(t105-t465).*9.53094055e-4+t903.*(t534-t546).*9.53094055e-4);
t5477 = t4518.*t4738;
t5480 = -ITail.*t4447.*(t2582-t2684+(t1510.*(t197-t537))./2.0+(t1505.*(t214-t541))./2.0);
t5481 = t4447.*(t2587-t3868+t1505.*(t534-t546).*1.90524867e-3);
t5484 = ITail.*t4313.*(t1141+t1386+t2501+(t817.*(t214-t541))./2.0+(t977.*(t103-t544))./2.0+(t1512.*(t105-t465))./2.0);
t5486 = -t4672.*(-t2388+t3008+t9.*t868.*(t105-t465).*9.53094055e-4);
t5502 = t4476.*t4775;
t5509 = t4471.*t4787;
t5511 = -ITail.*t4522.*(t2436-t2536+t1510.*(t197-t537)+t1505.*(t214-t541));
t5514 = t2564+t2565+t2892+t2902+t3502+t3511;
t5516 = -t4949.*(-t1262+t1701+t9.*t868.*(t105-t465));
t5519 = t2351+t2467+t3136+t3164+t3355+t3373;
t5521 = t4518.*t4770;
t5525 = -t4787.*(t1395-t2868+t1505.*(t534-t546).*2.0);
t5527 = -t4575.*(-t2389+t3634+t1512.*(t105-t465).*9.53094055e-4);
t5528 = ITail.*t4452.*t4821;
t5533 = t4787.*(t1395-t2868+t1505.*(t534-t546).*2.0);
t5536 = t4500.*(t1079+t1956-t4277-t1178.*(t105-t465));
t5537 = -t4581.*(-t2389+t3634+t1512.*(t105-t465).*9.53094055e-4);
t5540 = ITail.*t4452.*t4823;
t5542 = t4581.*(-t2389+t3634+t1512.*(t105-t465).*9.53094055e-4);
t5543 = ITail.*t4392.*t4874;
t5546 = (-t2389+t3634+t1512.*(t105-t465).*9.53094055e-4).*(t1019-t1651+t1702+t3.*t818.*(t105-t465)+t3.*t872.*(t103-t544));
t5550 = ITail.*t4392.*t4882;
t5551 = -t4949.*(-t947+t1240.*(t105-t465)+t903.*(t534-t546));
t5553 = -t4555.*(t2436-t2536+t1510.*(t197-t537)+t1505.*(t214-t541));
t5557 = -ITail.*t4077.*(t1176-t1366+t2434+t2435-t2899+t1430.*(t539+t641));
t5563 = ITail.*t4452.*t4830;
t5564 = -t4500.*(t1185+t1813-t4313+t1047.*(t105-t465));
t5567 = -ITail.*t4392.*(-t1189+t1195-t2210+t2241+t2248+(t8.*t872.*(t534-t546))./2.0);
t5571 = t4500.*(t1185+t1813-t4313+t1047.*(t105-t465));
t5573 = ITail.*t4408.*t4874;
t5575 = -t4518.*(t1060+t1138-t1883+t1932+t2088+t1179.*(t103-t544));
t5578 = ITail.*t4392.*(-t1189+t1195-t2210+t2241+t2248+(t8.*t872.*(t534-t546))./2.0);
t5580 = ITail.*t4408.*t4882;
t5583 = t2237+t2258+t3434+t3439+t3470+t3472;
t5585 = -t4592.*(-t2621+t3659+t1510.*(t103-t544).*8.56645e-6);
t5592 = ITail.*t4392.*t4908;
t5596 = t2514+t2566+t3160+t3266+t3501+t3510;
t5597 = t2615+t2714+t3200+t3224+t3401+t3456;
t5599 = -t4638.*(-t2389+t3634+t1512.*(t105-t465).*9.53094055e-4);
t5601 = -t4518.*(t1250-t1261+t1761-t2083-t2111+t1037.*(t103-t544));
t5602 = t4551.*(t1079+t1956-t4277-t1178.*(t105-t465));
t5603 = ITail.*t4447.*t4874;
t5606 = (-t2389+t3634+t1512.*(t105-t465).*9.53094055e-4).*(t1751+t2308+t964.*(t105-t465)+t1430.*(t103-t544));
t5612 = -t4618.*(-t2621+t3659+t1510.*(t103-t544).*8.56645e-6);
t5616 = -t4518.*(t1053+t1332+t2368+t817.*(t214-t541)+t977.*(t103-t544)+t1512.*(t105-t465));
t5618 = t4618.*(-t2621+t3659+t1510.*(t103-t544).*8.56645e-6);
t5619 = -ITail.*t4447.*(-t1189+t1195-t2210+t2241+t2248+(t8.*t872.*(t534-t546))./2.0);
t5622 = -t4551.*(t1185+t1813-t4313+t1047.*(t105-t465));
t5623 = ITail.*t4522.*t4823;
t5627 = ITail.*t4452.*t4897;
t5629 = -t4645.*(-t2621+t3659+t1510.*(t103-t544).*8.56645e-6);
t5631 = ITail.*t4522.*t4830;
t5632 = -ITail.*t4522.*(-t1129+t1139-t2082+t2110+t2123+t8.*t872.*(t534-t546));
t5633 = -t4672.*(-t2389+t3634+t1512.*(t105-t465).*9.53094055e-4);
t5638 = ITail.*t4447.*t4908;
t5642 = ITail.*t4522.*t4834;
t5644 = t4555.*t4821;
t5647 = t2503+t2712+t3426+t3460+t3477+t3533;
t5648 = -t4686.*(-t2389+t3634+t1512.*(t105-t465).*9.53094055e-4);
t5650 = t491+t824+t877+t1115+t1878+t2073+t4842;
t5655 = -ITail.*t4077.*(t1365-t1443+t2829-t2831-t2833+t1505.*(t534-t546));
t5658 = ITail.*t4476.*t4882;
t5659 = t4686.*(-t2389+t3634+t1512.*(t105-t465).*9.53094055e-4);
t5661 = ITail.*t4522.*t4849;
t5663 = ITail.*t4077.*(t1365-t1443+t2829-t2831-t2833+t1505.*(t534-t546));
t5667 = t4555.*t4823;
t5670 = -t4695.*(-t2389+t3634+t1512.*(t105-t465).*9.53094055e-4);
t5677 = -t4949.*(t1332+t2368+t1512.*(t105-t465));
t5678 = t4695.*(-t2389+t3634+t1512.*(t105-t465).*9.53094055e-4);
t5682 = t4555.*t4830;
t5684 = -t4555.*(-t1129+t1139-t2082+t2110+t2123+t8.*t872.*(t534-t546));
t5686 = ITail.*t4452.*t4923;
t5687 = t4555.*t4834;
t5688 = (-t2389+t3634+t1512.*(t105-t465).*9.53094055e-4).*(t1260-t1328-t1427-t1441+t1706+t9.*t870.*(t105-t465));
t5689 = ITail.*t4452.*t4922;
t5691 = -(-t2388+t3008+t9.*t868.*(t105-t465).*9.53094055e-4).*(t1079+t1956-t4277-t1178.*(t105-t465));
t5692 = ITail.*t4392.*t4961;
t5693 = ITail.*t4392.*t4960;
t5694 = ITail.*t4476.*t4908;
t5699 = t4555.*t4849;
t5704 = (-t2621+t3659+t1510.*(t103-t544).*8.56645e-6).*(t820+t1121-t1435+t1997+t2000+t11.*t420.*(t214-t541));
t5707 = ITail.*t4522.*t4897;
t5709 = (-t2388+t3008+t9.*t868.*(t105-t465).*9.53094055e-4).*(t1185+t1813-t4313+t1047.*(t105-t465));
t5710 = ITail.*t4408.*t4961;
t5712 = ITail.*t4408.*t4960;
t5715 = (-t2389+t3634+t1512.*(t105-t465).*9.53094055e-4).*(t753+t991-t1771-t1957+t1181.*(t105-t465)+t11.*t381.*(t534-t546));
t5717 = -(-t1974+t1240.*(t105-t465).*9.53094055e-4+t903.*(t534-t546).*9.53094055e-4).*(t1079+t1956-t4277-t1178.*(t105-t465));
t5721 = t4569+t4859;
t5722 = t1473+t1477+t3323+t3396+t4158+t4176;
t5726 = -t4277.*(t2449.*3.367829185e-3+t3556+t3557+t3576);
t5731 = ITail.*t4447.*t4960;
t5733 = (-t1974+t1240.*(t105-t465).*9.53094055e-4+t903.*(t534-t546).*9.53094055e-4).*(t1185+t1813-t4313+t1047.*(t105-t465));
t5734 = t4555.*t4897;
t5741 = ITail.*t4522.*t4923;
t5745 = -t4313.*(t2449.*3.367829185e-3+t3556+t3557+t3576);
t5754 = -t5749;
t5756 = -t4738.*(-t2621+t3659+t1510.*(t103-t544).*8.56645e-6);
t5761 = ITail.*t4476.*t4961;
t5763 = -t5757;
t5771 = t4555.*t4922;
t5772 = t4555.*t4923;
t5776 = -t4737.*(t2436-t2536+t1510.*(t197-t537)+t1505.*(t214-t541));
t5778 = t1661+t1976+t3791+t3811+t4043+t4070;
t5780 = t2318+t2782+t3495+t3532+t3935+t3946;
t5781 = -ITail.*t4452.*(t1176-t1366+t2434+t2435-t2899+t1430.*(t539+t641));
t5786 = -ITail.*t4392.*(t1255-t1465+t2578+t2579-t2997+(t1430.*(t539+t641))./2.0);
t5789 = ITail.*t4452.*(t1176-t1366+t2434+t2435-t2899+t1430.*(t539+t641));
t5792 = ITail.*t4392.*(t1255-t1465+t2578+t2579-t2997+(t1430.*(t539+t641))./2.0);
t5793 = t2335+t2588+t3751+t3752+t3866+t3897;
t5796 = -t4770.*(-t2621+t3659+t1510.*(t103-t544).*8.56645e-6);
t5805 = t4770.*(-t2621+t3659+t1510.*(t103-t544).*8.56645e-6);
t5814 = -t5806;
t5817 = t896+t1214+t1271+t1731+t2634+t2767+t4740;
t5818 = t924+t1201+t1213+t1828+t2294+t2299+t4778;
t5820 = -t4447.*(t2449.*3.36554e-3+t3490+t3556+t3557);
t5823 = t2422+t2782+t3562+t3660+t3935+t3946;
t5824 = dth1.*(t890+t1161-t1212+t1770+t2224-t2298-t4782);
t5826 = -ITail.*t4447.*(t1255-t1465+t2578+t2579-t2997+(t1430.*(t539+t641))./2.0);
t5829 = t2318+t2961+t3495+t3532+t4013+t4032;
t5835 = -t4787.*(t2436-t2536+t1510.*(t197-t537)+t1505.*(t214-t541));
t5841 = t4737.*t4821;
t5845 = -ITail.*t4452.*(t1365-t1443+t2829-t2831-t2833+t1505.*(t534-t546));
t5847 = t2104+t2277+t3879+t3936+t3978+t3994;
t5848 = t4737.*t4823;
t5855 = -t4555.*(t1176-t1366+t2434+t2435-t2899+t1430.*(t539+t641));
t5859 = t4737.*t4830;
t5862 = -t5857;
t5868 = t4162.*(-t2141+t2259+t2825+t2944+t3121+t3131);
t5881 = -t4447.*(t3716-t3777+t1510.*(t197-t537).*9.52624335e-4+t1505.*(t214-t541).*9.52624335e-4);
t5889 = t4787.*t4823;
t5891 = t4737.*t4897;
t5894 = t4787.*t4830;
t5895 = -t4787.*(-t1129+t1139-t2082+t2110+t2123+t8.*t872.*(t534-t546));
t5897 = t4162.*(-t2218+t2342+t3054+t3096+t3121+t3131);
t5901 = t4787.*t4834;
t5906 = -t4555.*(t1365-t1443+t2829-t2831-t2833+t1505.*(t534-t546));
t5908 = t4787.*t4849;
t5909 = t4162.*(-t1928+t2254+t2994+t3064+t3407+t3431);
t5910 = t4555.*(t1365-t1443+t2829-t2831-t2833+t1505.*(t534-t546));
t5915 = t4313.*(-t2141+t2259+t2825+t2944+t3121+t3131);
t5916 = t3961.*t5548;
t5917 = t3938.*t5556;
t5919 = t3938.*t5566;
t5923 = t4737.*t4923;
t5925 = t4737.*t4922;
t5935 = t4277.*(-t2218+t2342+t3054+t3096+t3121+t3131);
t5940 = t3509+t3537+t3675+t3676+t3934+t3966;
t5941 = t4787.*t4897;
t5943 = t3556+t3557+t3625+t3664+t3934+t3966;
t5944 = t3509+t3537+t3556+t3557+t4001+t4034;
t5947 = t3938.*t5607;
t5959 = -(-t1331+t2317+t1510.*(t103-t544)).*(-t2141+t2259+t2825+t2944+t3121+t3131);
t5960 = t4313.*(-t1928+t2254+t2994+t3064+t3407+t3431);
t5964 = t4173.*t5548;
t5967 = t4787.*t4923;
t5970 = -t5548.*(-t1262+t1701+t9.*t868.*(t105-t465));
t5973 = -t4162.*(t2208+t2312-t3315+t3347+t3475+t1179.*(t103-t544).*8.56645e-6);
t5980 = t4162.*(t2514-t2518+t3160+t3266+t3501+t3510);
t5981 = -t5548.*(-t947+t1240.*(t105-t465)+t903.*(t534-t546));
t5982 = -(-t1331+t2317+t1510.*(t103-t544)).*(-t2218+t2342+t3054+t3096+t3121+t3131);
t5983 = -t4162.*(t2202+t2564+t3719+t817.*(t214-t541).*8.56645e-6+t977.*(t103-t544).*8.56645e-6+t1512.*(t105-t465).*8.56645e-6);
t5986 = -t4737.*(t1176-t1366+t2434+t2435-t2899+t1430.*(t539+t641));
t5988 = -t4277.*(t2208+t2312-t3315+t3347+t3475+t1179.*(t103-t544).*8.56645e-6);
t5989 = -(-t1331+t2317+t1510.*(t103-t544)).*(-t1928+t2254+t2994+t3064+t3407+t3431);
t5990 = t4737.*(t1176-t1366+t2434+t2435-t2899+t1430.*(t539+t641));
t5991 = t4277.*(t2208+t2312-t3315+t3347+t3475+t1179.*(t103-t544).*8.56645e-6);
t5992 = (-t1331+t2317+t1510.*(t103-t544)).*(-t1928+t2254+t2994+t3064+t3407+t3431);
t5996 = t4277.*(t2514-t2518+t3160+t3266+t3501+t3510);
t5998 = -t4313.*(t2208+t2312-t3315+t3347+t3475+t1179.*(t103-t544).*8.56645e-6);
t6000 = -t4277.*(t2202+t2564+t3719+t817.*(t214-t541).*8.56645e-6+t977.*(t103-t544).*8.56645e-6+t1512.*(t105-t465).*8.56645e-6);
t6001 = t4313.*(t2514-t2518+t3160+t3266+t3501+t3510);
t6005 = -t4313.*(t2202+t2564+t3719+t817.*(t214-t541).*8.56645e-6+t977.*(t103-t544).*8.56645e-6+t1512.*(t105-t465).*8.56645e-6);
t6009 = t764+t1349+t1405+t1589+t2519+t3316+t3324+t4166+t4168;
t6010 = t4313.*(t2202+t2564+t3719+t817.*(t214-t541).*8.56645e-6+t977.*(t103-t544).*8.56645e-6+t1512.*(t105-t465).*8.56645e-6);
t6013 = -t4737.*(t1365-t1443+t2829-t2831-t2833+t1505.*(t534-t546));
t6014 = t4392.*t5556;
t6015 = t4392.*t5566;
t6019 = -t4392.*(t2215-t2237+t3424+t3427-t3439+t8.*t872.*(t534-t546).*9.52624335e-4);
t6021 = t4408.*t5556;
t6024 = t4392.*(t2215-t2237+t3424+t3427-t3439+t8.*t872.*(t534-t546).*9.52624335e-4);
C = ft_11({B_cg_H,ITail,Mb,Mm,Mt,T_cg_H,dphi1,dphi2,dpsi1,dth1,dth2,dx,dy,dz,t10,t1003,t1005,t1006,t1007,t1008,t1009,t1013,t1014,t1015,t1016,t1017,t1018,t1019,t1023,t1029,t103,t1037,t1047,t105,t1050,t1053,t1059,t1060,t1064,t1068,t1071,t1072,t1075,t1076,t1077,t1078,t1079,t1084,t1086,t1088,t1097,t1099,t11,t1102,t1108,t1113,t1116,t1121,t1129,t1133,t1134,t1135,t1136,t1137,t1138,t1139,t1141,t1142,t1143,t1147,t1149,t1153,t1155,t1157,t1159,t1160,t1162,t1164,t1167,t1169,t1170,t1173,t1176,t1178,t1179,t1181,t1185,t1186,t1187,t1188,t1189,t1191,t1192,t1193,t1194,t1195,t1196,t120,t1200,t1203,t1205,t1206,t1211,t1215,t1221,t1223,t1224,t1225,t1228,t1229,t1230,t1234,t1240,t1242,t1244,t1245,t1246,t1247,t1250,t1252,t1253,t1255,t1260,t1261,t1262,t1264,t1265,t1268,t1280,t1283,t1291,t130,t1301,t1302,t1303,t1304,t1305,t1307,t1309,t1313,t1322,t1328,t1331,t1332,t1334,t1337,t1338,t134,t1343,t1344,t1345,t1348,t1352,t1354,t1355,t1356,t1360,t1362,t1365,t1366,t1368,t1370,t1371,t1373,t1374,t1378,t1381,t1382,t1384,t1386,t1388,t1389,t1391,t1393,t1394,t1395,t1396,t1397,t1403,t1406,t1412,t1413,t1415,t1416,t1421,t1426,t1427,t1430,t1431,t1433,t1435,t144,t1441,t1443,t1444,t1446,t1453,t1455,t1456,t1457,t1458,t1460,t1463,t1465,t1466,t1467,t1468,t1469,t1470,t1476,t1479,t1480,t1481,t1486,t1487,t1495,t15,t1505,t1506,t1508,t1510,t1512,t1513,t1516,t1518,t1521,t1525,t1526,t1528,t1529,t1531,t1535,t1540,t1543,t1544,t1546,t1549,t1551,t1552,t1558,t1562,t1563,t1568,t1575,t1578,t1581,t1585,t1586,t1587,t1590,t1593,t1595,t1596,t1597,t1598,t1599,t1605,t1609,t161,t1612,t1618,t1619,t162,t1620,t1621,t1624,t1627,t1628,t1630,t1633,t1634,t1635,t1636,t1637,t1639,t1640,t1643,t1645,t1646,t1650,t1651,t1652,t1654,t1655,t1656,t1657,t1659,t1660,t1661,t1663,t1664,t1665,t1667,t1669,t1672,t1674,t1675,t1676,t1678,t1679,t1680,t1681,t1682,t1683,t1685,t1691,t1692,t1693,t1694,t1695,t1696,t1698,t1699,t1700,t1701,t1702,t1703,t1705,t1706,t1716,t1718,t1719,t1720,t1721,t1722,t1723,t1725,t1727,t1730,t1734,t1735,t1736,t1737,t1739,t1740,t1741,t1742,t1744,t1746,t1747,t1748,t1751,t1752,t1759,t1761,t1763,t1764,t1765,t1771,t1774,t1777,t1778,t1779,t1780,t1781,t1782,t1783,t1784,t1785,t1786,t1787,t1788,t1789,t1790,t1792,t1798,t1799,t1800,t1801,t1802,t1806,t1809,t1810,t1813,t1820,t1821,t1832,t1836,t1840,t1841,t1843,t1846,t1851,t1853,t1855,t1857,t1858,t1859,t1860,t1865,t1866,t1867,t1874,t1875,t1882,t1883,t1888,t1890,t1895,t1896,t1898,t1899,t1900,t1904,t1905,t1907,t1908,t1909,t1910,t1912,t1915,t1916,t1917,t1918,t1928,t1929,t1930,t1931,t1932,t1938,t1939,t1941,t1942,t1943,t1945,t1947,t1948,t195,t1950,t1951,t1952,t1956,t1957,t1959,t1961,t1962,t1963,t1964,t1965,t1966,t1969,t197,t1970,t1971,t1973,t1974,t1976,t1977,t1979,t1981,t1982,t1983,t1993,t1997,t1998,t1999,t2,t2000,t2002,t2004,t2007,t2008,t2009,t2011,t2012,t2013,t2015,t2016,t2017,t2018,t2020,t2023,t2024,t2025,t2032,t2033,t2037,t2038,t2042,t2045,t2046,t2047,t2049,t2050,t2057,t2058,t2059,t2061,t2062,t2064,t2065,t2066,t2067,t2068,t2069,t2072,t2075,t2076,t2081,t2082,t2083,t2086,t2087,t2088,t2089,t2090,t2091,t2094,t2096,t2102,t2104,t2106,t2107,t2108,t2109,t2110,t2111,t2113,t2117,t2118,t2119,t2123,t2130,t2131,t2134,t2135,t2137,t2139,t214,t2141,t2143,t2144,t2147,t2148,t2150,t2151,t2152,t2153,t2154,t2155,t2156,t2157,t2158,t2161,t2165,t2171,t2172,t2174,t2175,t2178,t2179,t2181,t2182,t2183,t2186,t2188,t2189,t2190,t2191,t2192,t2196,t2197,t2202,t2203,t2206,t2208,t2210,t2211,t2212,t2215,t2216,t2217,t2218,t2220,t2221,t2222,t2223,t2225,t2227,t2229,t2230,t2237,t2240,t2241,t2242,t2243,t2245,t2247,t2248,t2249,t2251,t2252,t2253,t2254,t2255,t2257,t2259,t2260,t2262,t2263,t2268,t2269,t2271,t2274,t2276,t2281,t2282,t2285,t2286,t2287,t2288,t2289,t2290,t2293,t2305,t2307,t2308,t2312,t2316,t2317,t2318,t2319,t2320,t2321,t2322,t2324,t2325,t2329,t2334,t2336,t2338,t2339,t2340,t2341,t2342,t2343,t2345,t2346,t2347,t2348,t2349,t2350,t2352,t2354,t2356,t2358,t2360,t2361,t2362,t2363,t2364,t2368,t2376,t2382,t2385,t2386,t2387,t2388,t2389,t2390,t2391,t2392,t2397,t2399,t24,t2400,t2401,t2404,t2406,t2407,t2408,t2409,t2410,t2411,t2412,t2413,t2419,t2420,t2422,t2426,t2427,t2428,t2429,t2430,t2431,t2433,t2434,t2435,t2436,t2437,t2438,t2447,t2449,t2458,t2461,t2462,t2463,t2465,t2468,t2470,t2471,t2472,t2474,t2476,t2479,t2480,t2483,t2485,t2486,t2487,t2488,t2489,t2492,t2495,t2496,t25,t2501,t2503,t2504,t2512,t2513,t2514,t2515,t2516,t2518,t2522,t2523,t2524,t2525,t2526,t2527,t2528,t2530,t2531,t2533,t2534,t2535,t2536,t2543,t2545,t2546,t2547,t2550,t2551,t2552,t2555,t2557,t2559,t2560,t2562,t2563,t2564,t2567,t2568,t2569,t2570,t2571,t2573,t2574,t2576,t2577,t2578,t2579,t2581,t2582,t2584,t2585,t2587,t2589,t259,t2590,t2591,t2597,t2598,t2599,t26,t260,t2600,t2605,t2607,t2613,t2616,t2617,t2619,t2621,t2623,t2624,t2627,t2629,t2630,t2632,t2636,t2637,t2638,t2646,t2648,t2650,t2652,t2655,t2657,t2659,t2660,t2661,t2662,t2663,t2665,t2666,t2667,t2668,t2669,t2671,t2673,t2677,t2678,t2679,t2682,t2684,t2688,t2689,t2692,t2696,t2698,t2699,t27,t2700,t2705,t2706,t2707,t2708,t2710,t2712,t2715,t2717,t2718,t2722,t2723,t2725,t2726,t2727,t2728,t2730,t2733,t2734,t2735,t2736,t2737,t2738,t2740,t2742,t2743,t2744,t2746,t2749,t2750,t2751,t2752,t2754,t2756,t2758,t2759,t276,t2760,t2761,t2763,t2764,t2765,t2766,t2768,t277,t2772,t2774,t2776,t2778,t2779,t2781,t2783,t2785,t2786,t2787,t2788,t2790,t2791,t2792,t2794,t2796,t2797,t2798,t2799,t2800,t2802,t2803,t2804,t2805,t2806,t2808,t2811,t2813,t2814,t2816,t2817,t2818,t2819,t2821,t2823,t2824,t2825,t2829,t283,t2831,t2832,t2833,t2834,t2836,t2837,t2838,t2839,t284,t2841,t2842,t2843,t2844,t2845,t2846,t2847,t2849,t285,t2853,t2857,t2858,t2859,t286,t2860,t2861,t2864,t2865,t2868,t287,t2870,t2871,t2872,t2874,t2875,t2876,t2877,t2878,t2879,t288,t2882,t2883,t2884,t2886,t2887,t2889,t289,t2890,t2893,t2896,t2897,t2898,t2899,t290,t2903,t2909,t291,t2912,t2913,t2914,t2915,t2916,t2917,t2918,t2919,t292,t2920,t2921,t2926,t2927,t2928,t293,t2930,t2932,t2936,t2937,t2938,t294,t2941,t2942,t2943,t2944,t2945,t2946,t2949,t2950,t2952,t2954,t2956,t2959,t2960,t2962,t2963,t2964,t2965,t2966,t2970,t2972,t2973,t2976,t2977,t2978,t2979,t2981,t2982,t2985,t2988,t2989,t2992,t2994,t2995,t2996,t2997,t2998,t3,t3004,t3006,t3007,t3008,t3009,t3011,t3012,t3016,t3017,t3019,t3022,t3027,t3030,t3031,t3032,t3033,t3034,t3035,t3037,t3038,t304,t3040,t3041,t3042,t3043,t3047,t3049,t3050,t3051,t3054,t3059,t3060,t3061,t3062,t3063,t3064,t3070,t3075,t3076,t3078,t3080,t3082,t3083,t3084,t3085,t3086,t3087,t3089,t3090,t3091,t3092,t3093,t3094,t3096,t3097,t3098,t3100,t3103,t3105,t3106,t3107,t3108,t3109,t3110,t3112,t3113,t3117,t3121,t3122,t3127,t3128,t3131,t3132,t3134,t3135,t3138,t3139,t3145,t3146,t3147,t3149,t3151,t3153,t3155,t3156,t3158,t3160,t3161,t3162,t3163,t3166,t3167,t3169,t3170,t3171,t3173,t3174,t3176,t3177,t3178,t3179,t3180,t3183,t3184,t3185,t3186,t3187,t3190,t3192,t3193,t3196,t3199,t3203,t3204,t3206,t3207,t3210,t3212,t3213,t3214,t3215,t3216,t3217,t3218,t3221,t3222,t3223,t3226,t3230,t3231,t3232,t3233,t3235,t3236,t3239,t3241,t3243,t3244,t3245,t3247,t3248,t3250,t3251,t3252,t3254,t3256,t3257,t3258,t3260,t3261,t3262,t3263,t3265,t3266,t3267,t3270,t3271,t3272,t3273,t3276,t3277,t3278,t3279,t3280,t3284,t3285,t3286,t3287,t3289,t3290,t3296,t3299,t3300,t3301,t3302,t3303,t3304,t3305,t3306,t3307,t3308,t3311,t3312,t3313,t3314,t3315,t3317,t3319,t3320,t3321,t3322,t3325,t3326,t3327,t3328,t3329,t3330,t3331,t3332,t3333,t3334,t3335,t3336,t3337,t3338,t3339,t3340,t3341,t3342,t3343,t3344,t3347,t3349,t3351,t3354,t3357,t3359,t3360,t3367,t3368,t3372,t3375,t3376,t3377,t3378,t3379,t3380,t3381,t3384,t3385,t3386,t3387,t3388,t3390,t3391,t3392,t3397,t3399,t3402,t3403,t3404,t3405,t3406,t3407,t3409,t3411,t3412,t3413,t3414,t3415,t3416,t3419,t3423,t3424,t3427,t3429,t3431,t3432,t3433,t3437,t3438,t3439,t3440,t3441,t3442,t3443,t3444,t3445,t3446,t3447,t3448,t3449,t3454,t3457,t3458,t3459,t3460,t3463,t3465,t3466,t3467,t3469,t3471,t3473,t3474,t3475,t3476,t3478,t3480,t3481,t3482,t3483,t3484,t3485,t3486,t3487,t3488,t3489,t3490,t3491,t3492,t3494,t3497,t3499,t3500,t3501,t3504,t3506,t3508,t3510,t3512,t3513,t3515,t3516,t3517,t3521,t3522,t3523,t3524,t3526,t3528,t3529,t3530,t3531,t3534,t3535,t3536,t3538,t3539,t3540,t3541,t3542,t3543,t3544,t3545,t3547,t3548,t3550,t3552,t3553,t3554,t3555,t3556,t3557,t3558,t3559,t3563,t3565,t3570,t3571,t3575,t3576,t3578,t3579,t3581,t3582,t3583,t3584,t3587,t3588,t3591,t3594,t3595,t3596,t3597,t3598,t3600,t3602,t3603,t3605,t3609,t3610,t3611,t3613,t3614,t3615,t3616,t3617,t3618,t3619,t3620,t3621,t3622,t3623,t3624,t3627,t3629,t3630,t3632,t3634,t3637,t3638,t3639,t3643,t3644,t3646,t3647,t3648,t3649,t3651,t3652,t3653,t3654,t3655,t3657,t3659,t3661,t3666,t3667,t3668,t3670,t3671,t3672,t3673,t3674,t3677,t3678,t3679,t3680,t3681,t3682,t3683,t3684,t3685,t3686,t3687,t3689,t3690,t3693,t3697,t3698,t3699,t3700,t3701,t3702,t3704,t3708,t3709,t3710,t3711,t3716,t3719,t3720,t3721,t3722,t3723,t3724,t3730,t3735,t3736,t3738,t3739,t3741,t3742,t3744,t3745,t3746,t3747,t3748,t3749,t3750,t3755,t3756,t3757,t3758,t3759,t376,t3760,t3761,t3762,t3764,t3765,t3766,t3767,t3769,t377,t3770,t3771,t3772,t3773,t3774,t3775,t3777,t3779,t3780,t3784,t3785,t3787,t3789,t3791,t3792,t3793,t3794,t3795,t3797,t3798,t3799,t3800,t3802,t3804,t3805,t3806,t3807,t3808,t3809,t381,t3811,t3812,t3814,t3815,t3817,t3818,t3819,t382,t3820,t3823,t3824,t3825,t3826,t3828,t3829,t383,t3831,t3832,t3833,t3834,t3836,t3837,t3838,t3840,t3841,t3842,t3845,t3846,t3847,t3848,t3849,t3850,t3851,t3854,t3855,t3856,t3858,t3859,t3860,t3861,t3862,t3867,t3868,t3870,t3871,t3872,t3873,t3876,t3879,t3880,t3882,t3883,t3885,t3886,t3887,t3888,t3889,t3890,t3891,t3892,t3893,t3894,t3896,t3898,t390,t3900,t3902,t3903,t3906,t3907,t3908,t3909,t3911,t3913,t3914,t3915,t3916,t3918,t3919,t3921,t3923,t3925,t3926,t3928,t3929,t3930,t3931,t3932,t3933,t3934,t3936,t3937,t3938,t3939,t394,t3940,t3943,t3944,t3945,t3947,t3948,t3949,t3950,t3951,t3952,t3953,t3954,t3955,t3956,t3957,t3958,t3959,t3960,t3961,t3962,t3964,t3965,t3966,t3967,t3969,t3971,t3974,t3975,t3976,t3977,t3979,t3980,t3981,t3982,t3983,t3984,t3985,t3986,t3988,t3989,t3991,t3992,t3993,t3995,t3996,t3998,t4,t4000,t4001,t4003,t4005,t4006,t4007,t4008,t4009,t4010,t4012,t4014,t4016,t4017,t4019,t4020,t4021,t4022,t4023,t4024,t4025,t4026,t4027,t4028,t4029,t4033,t4034,t4035,t4036,t4037,t4038,t4040,t4041,t4042,t4044,t4046,t4047,t4048,t4050,t4051,t4052,t4053,t4054,t4056,t4058,t4059,t4061,t4062,t4064,t4065,t4066,t4068,t4070,t4071,t4072,t4073,t4074,t4077,t4078,t4081,t4083,t4084,t4085,t4086,t4087,t4089,t4090,t4091,t4092,t4093,t4094,t4095,t4096,t4097,t4098,t4099,t410,t4100,t4104,t4105,t4107,t4108,t4109,t411,t4111,t4112,t4115,t4116,t4117,t4119,t412,t4120,t4121,t4122,t4126,t4129,t413,t4130,t4132,t4133,t4135,t4137,t4138,t4139,t414,t4140,t4141,t4143,t4144,t4145,t4147,t4148,t415,t4151,t4152,t4153,t4154,t4155,t4156,t4157,t4160,t4162,t4164,t4165,t4169,t4170,t4171,t4173,t4174,t4177,t4178,t4179,t4182,t4184,t4186,t4187,t4188,t4189,t4190,t4191,t4192,t4193,t4194,t4195,t4196,t4197,t420,t4200,t4201,t4202,t4203,t4204,t4205,t4206,t4208,t4209,t421,t4210,t4211,t4212,t4213,t4214,t4215,t4216,t4217,t4218,t4220,t4221,t4222,t4223,t4224,t4225,t4226,t4227,t4228,t4229,t4230,t4231,t4232,t4233,t4234,t4236,t4237,t4238,t4239,t4240,t4241,t4243,t4244,t4245,t4246,t4247,t4248,t4249,t425,t4250,t4252,t4253,t4255,t4256,t4258,t4259,t4260,t4261,t4262,t4263,t4265,t4266,t4268,t4269,t4271,t4272,t4273,t4274,t4276,t4277,t4278,t4280,t4281,t4282,t4285,t4286,t4290,t4295,t4296,t4298,t430,t4300,t4301,t4302,t4303,t4304,t4305,t4306,t4307,t4308,t4309,t431,t4310,t4311,t4312,t4313,t4315,t4316,t4317,t4318,t4319,t4320,t4321,t4322,t4323,t4324,t4326,t4327,t4329,t433,t4330,t4332,t4333,t4334,t4337,t4339,t4340,t4341,t4342,t4343,t4344,t4345,t4346,t4347,t4348,t4349,t4350,t4351,t4352,t4354,t4355,t4356,t4357,t4358,t4359,t436,t4360,t4361,t4362,t4364,t4365,t4367,t4368,t4370,t4371,t4372,t4373,t4374,t4375,t4376,t4377,t4378,t4379,t4380,t4382,t4383,t4384,t4385,t4386,t4387,t4388,t4389,t4392,t4393,t4394,t4395,t4399,t44,t4400,t4401,t4402,t4403,t4404,t4405,t4406,t4407,t4408,t4409,t4411,t4412,t4413,t4414,t4415,t4416,t4418,t4419,t4420,t4421,t4422,t4424,t4425,t4427,t4428,t4429,t4431,t4432,t4433,t4434,t4435,t4437,t4438,t4439,t4440,t4442,t4444,t4447,t4449,t445,t4450,t4451,t4452,t4453,t4454,t4455,t4457,t4458,t4459,t4460,t4461,t4462,t4465,t4467,t4469,t4470,t4471,t4472,t4473,t4475,t4476,t4477,t4478,t4479,t4480,t4481,t4482,t4483,t4484,t4485,t4486,t4487,t4488,t4489,t4490,t4492,t4493,t4495,t4496,t4497,t4498,t4499,t4500,t4501,t4502,t4503,t4504,t4505,t4506,t4507,t451,t4511,t4512,t4514,t4515,t4517,t4518,t4519,t4520,t4521,t4522,t4523,t4524,t4525,t4526,t4528,t4529,t4530,t4531,t4532,t4533,t4534,t4536,t4537,t4538,t4541,t4542,t4545,t4546,t4547,t4548,t4549,t4550,t4551,t4552,t4553,t4555,t4556,t4557,t4558,t4559,t4560,t4561,t4562,t4563,t4566,t4567,t4570,t4571,t4572,t4573,t4574,t4575,t4576,t4577,t4578,t4580,t4581,t4583,t4584,t4585,t4587,t4588,t4589,t459,t4591,t4592,t4597,t4598,t4600,t4601,t4602,t4603,t4604,t4605,t4606,t4608,t4610,t4613,t4614,t4615,t4616,t4617,t4618,t4619,t4620,t4621,t4622,t4623,t4624,t4625,t4626,t4629,t4630,t4634,t4636,t4637,t4638,t4639,t4641,t4645,t4646,t4647,t4649,t465,t4651,t4652,t4653,t4655,t4657,t4659,t4660,t4661,t4662,t4663,t4664,t4665,t4666,t4667,t4668,t4669,t4672,t4673,t4674,t4675,t4678,t4681,t4682,t4683,t4684,t4685,t4686,t4687,t4695,t4697,t4698,t4700,t4701,t4702,t4704,t4705,t4706,t4707,t4708,t4709,t4710,t4711,t4712,t4713,t4720,t4722,t4723,t4724,t4729,t4732,t4733,t4735,t4736,t4737,t4738,t4742,t4746,t4747,t4749,t4750,t4751,t4752,t4753,t4754,t4755,t4756,t4758,t4759,t4761,t4764,t4766,t4769,t4770,t4771,t4772,t4773,t4775,t4776,t4780,t4781,t4783,t4784,t4785,t4786,t4787,t4788,t4789,t4790,t4796,t4799,t48,t4800,t4801,t4802,t4803,t4805,t4806,t4807,t4809,t4810,t4811,t4815,t4816,t4820,t4821,t4823,t4826,t4830,t4831,t4832,t4834,t4836,t4838,t4841,t4843,t4844,t4845,t4846,t4847,t4848,t4849,t485,t4850,t4851,t4852,t4853,t4858,t4862,t4864,t4865,t4867,t4870,t4871,t4873,t4874,t4877,t4878,t4879,t488,t4880,t4881,t4882,t4883,t4884,t4888,t4889,t4890,t4892,t4895,t4897,t49,t4900,t4901,t4903,t4904,t4906,t4908,t4909,t4911,t4912,t4913,t4914,t4915,t4922,t4923,t4924,t4925,t4926,t4927,t4928,t4929,t4931,t4932,t4933,t4934,t4936,t4937,t4938,t4939,t4940,t4941,t4942,t4943,t4944,t4945,t4946,t4947,t4948,t4949,t4950,t4953,t4954,t496,t4960,t4961,t4963,t4964,t4966,t4967,t4968,t4969,t4972,t4973,t4974,t4975,t4976,t4977,t4978,t4979,t4980,t4982,t4983,t4986,t4987,t4988,t4989,t4990,t4991,t4993,t4995,t4996,t4997,t4998,t4999,t5,t50,t5000,t5002,t5004,t5005,t5006,t5007,t5008,t5009,t501,t5010,t5012,t5014,t5016,t5017,t5018,t5019,t502,t5021,t5022,t5023,t5024,t5026,t5027,t5030,t5031,t5032,t5033,t5036,t5038,t5039,t504,t5040,t5041,t5042,t5046,t5047,t5048,t5050,t5051,t5052,t5053,t5054,t5055,t5057,t5058,t5059,t5060,t5061,t5062,t5063,t5064,t5066,t5067,t5072,t5074,t5076,t5077,t5078,t5080,t5082,t5083,t5084,t5085,t5088,t5090,t5092,t5093,t5095,t5098,t5099,t51,t5101,t5102,t5103,t5104,t5109,t5111,t5112,t5114,t5120,t5121,t5123,t5126,t5128,t5131,t5135,t5136,t5137,t5139,t5143,t5144,t5146,t5149,t5150,t5152,t5153,t5154,t5155,t5156,t5158,t5161,t5163,t5165,t5166,t5167,t5171,t5172,t5173,t5174,t5176,t5177,t5178,t5179,t5182,t5184,t5185,t519,t5190,t5191,t5193,t5194,t5197,t5198,t5199,t5202,t5203,t5204,t5205,t5206,t5207,t5208,t5214,t5215,t5217,t5218,t5220,t5223,t5224,t5225,t5227,t5229,t523,t5232,t5237,t5238,t5239,t524,t5240,t5241,t5244,t5246,t5250,t5251,t5256,t5263,t5265,t5266,t5268,t527,t5271,t5272,t5274,t5275,t5280,t5285,t5286,t5287,t5288,t5289,t5290,t5291,t5293,t5294,t5299,t530,t5300,t5301,t5302,t5304,t5306,t5308,t5309,t5310,t5311,t5312,t5313,t5316,t5317,t5318,t5319,t5321,t5324,t5325,t5326,t5327,t5328,t5329,t5334,t5335,t5336,t5338,t534,t5340,t5344,t5345,t5346,t5347,t5348,t5349,t5351,t5352,t5353,t5354,t5356,t5358,t5363,t5364,t5368,t5369,t537,t5370,t5372,t5374,t5378,t5379,t5380,t5382,t5384,t5385,t5386,t539,t5391,t5392,t5393,t5396,t5398,t5399,t54,t5401,t5404,t5405,t5406,t5407,t5409,t541,t5412,t5413,t5417,t5419,t542,t5420,t5421,t5422,t5423,t5424,t5425,t5427,t5428,t5429,t5430,t5431,t5435,t5437,t5438,t5439,t544,t5441,t5443,t5444,t5445,t5447,t5448,t5452,t5453,t5455,t5456,t5458,t5459,t546,t5460,t5461,t5463,t5464,t5470,t5474,t5475,t5476,t5477,t5480,t5481,t5484,t5486,t5488,t5490,t5492,t5493,t5494,t5498,t55,t550,t5502,t5509,t5511,t5514,t5516,t5519,t5521,t5523,t5524,t5527,t5528,t553,t5530,t5533,t5536,t5538,t5539,t5540,t5542,t5543,t5546,t5547,t5548,t5550,t5551,t5552,t5553,t5556,t5557,t5563,t5565,t5566,t5569,t557,t5571,t5573,t5575,t5576,t5578,t558,t5580,t5582,t5585,t5588,t5592,t5597,t5598,t5599,t56,t5601,t5602,t5603,t5606,t5607,t5616,t5618,t5619,t5620,t5622,t5623,t5627,t5629,t5631,t5632,t5633,t5638,t5642,t5644,t5648,t5657,t5658,t5659,t5660,t5661,t5662,t5663,t5664,t5667,t5668,t5670,t5672,t5674,t5677,t5678,t5682,t5684,t5685,t5686,t5687,t5688,t5689,t5690,t5691,t5692,t5693,t5694,t5696,t5697,t5699,t5704,t5705,t5706,t5707,t5709,t5710,t5712,t5713,t5715,t5717,t5721,t5722,t5724,t5726,t573,t5730,t5731,t5733,t5734,t5738,t574,t5741,t5745,t5749,t575,t5754,t5756,t5761,t5763,t5771,t5772,t5776,t5778,t5779,t5780,t5781,t5785,t5786,t5788,t5789,t5791,t5792,t5793,t5795,t5798,t5800,t5805,t5808,t5809,t5814,t5815,t5818,t5820,t5823,t5824,t5826,t5829,t5832,t5835,t5837,t5840,t5841,t5843,t5845,t5846,t5847,t5848,t5855,t5857,t5859,t5862,t5867,t5868,t5869,t587,t5870,t5874,t5880,t5881,t5887,t5889,t5891,t5894,t5895,t5897,t59,t5901,t5905,t5908,t5909,t5910,t5915,t5916,t5917,t5919,t5923,t5925,t5926,t5932,t5933,t5935,t5936,t5939,t5941,t5947,t5949,t595,t5959,t5960,t5963,t5964,t5967,t5970,t5971,t5973,t5980,t5981,t5982,t5983,t5984,t5985,t5986,t5988,t5989,t5990,t5991,t5992,t5996,t5998,t6000,t6001,t6009,t6010,t6013,t6014,t6015,t6021,t6024,t603,t6049,t6051,t6052,t6066,t6067,t6074,t6083,t6099,t61,t6117,t6129,t614,t628,t629,t634,t641,t65,t650,t651,t655,t6555,t6557,t657,t6599,t6628,t6629,t664,t665,t666,t667,t668,t669,t675,t68,t693,t7,t71,t721,t724,t73,t731,t732,t736,t741,t753,t754,t755,t756,t757,t759,t760,t761,t762,t765,t769,t772,t774,t776,t778,t795,t797,t799,t8,t802,t803,t806,t817,t818,t820,t828,t831,t838,t843,t846,t847,t848,t850,t851,t852,t853,t855,t865,t867,t868,t870,t871,t872,t876,t886,t888,t9,t901,t902,t903,t904,t906,t907,t909,t914,t925,t926,t947,t949,t952,t955,t957,t964,t972,t977,t983,t991,t992,t993,t994,t995});
end
function C = ft_11(ct)
B_cg_H = ct{1};
ITail = ct{2};
Mb = ct{3};
Mm = ct{4};
Mt = ct{5};
T_cg_H = ct{6};
dphi1 = ct{7};
dphi2 = ct{8};
dpsi1 = ct{9};
dth1 = ct{10};
dth2 = ct{11};
dx = ct{12};
dy = ct{13};
dz = ct{14};
t10 = ct{15};
t1003 = ct{16};
t1005 = ct{17};
t1006 = ct{18};
t1007 = ct{19};
t1008 = ct{20};
t1009 = ct{21};
t1013 = ct{22};
t1014 = ct{23};
t1015 = ct{24};
t1016 = ct{25};
t1017 = ct{26};
t1018 = ct{27};
t1019 = ct{28};
t1023 = ct{29};
t1029 = ct{30};
t103 = ct{31};
t1037 = ct{32};
t1047 = ct{33};
t105 = ct{34};
t1050 = ct{35};
t1053 = ct{36};
t1059 = ct{37};
t1060 = ct{38};
t1064 = ct{39};
t1068 = ct{40};
t1071 = ct{41};
t1072 = ct{42};
t1075 = ct{43};
t1076 = ct{44};
t1077 = ct{45};
t1078 = ct{46};
t1079 = ct{47};
t1084 = ct{48};
t1086 = ct{49};
t1088 = ct{50};
t1097 = ct{51};
t1099 = ct{52};
t11 = ct{53};
t1102 = ct{54};
t1108 = ct{55};
t1113 = ct{56};
t1116 = ct{57};
t1121 = ct{58};
t1129 = ct{59};
t1133 = ct{60};
t1134 = ct{61};
t1135 = ct{62};
t1136 = ct{63};
t1137 = ct{64};
t1138 = ct{65};
t1139 = ct{66};
t1141 = ct{67};
t1142 = ct{68};
t1143 = ct{69};
t1147 = ct{70};
t1149 = ct{71};
t1153 = ct{72};
t1155 = ct{73};
t1157 = ct{74};
t1159 = ct{75};
t1160 = ct{76};
t1162 = ct{77};
t1164 = ct{78};
t1167 = ct{79};
t1169 = ct{80};
t1170 = ct{81};
t1173 = ct{82};
t1176 = ct{83};
t1178 = ct{84};
t1179 = ct{85};
t1181 = ct{86};
t1185 = ct{87};
t1186 = ct{88};
t1187 = ct{89};
t1188 = ct{90};
t1189 = ct{91};
t1191 = ct{92};
t1192 = ct{93};
t1193 = ct{94};
t1194 = ct{95};
t1195 = ct{96};
t1196 = ct{97};
t120 = ct{98};
t1200 = ct{99};
t1203 = ct{100};
t1205 = ct{101};
t1206 = ct{102};
t1211 = ct{103};
t1215 = ct{104};
t1221 = ct{105};
t1223 = ct{106};
t1224 = ct{107};
t1225 = ct{108};
t1228 = ct{109};
t1229 = ct{110};
t1230 = ct{111};
t1234 = ct{112};
t1240 = ct{113};
t1242 = ct{114};
t1244 = ct{115};
t1245 = ct{116};
t1246 = ct{117};
t1247 = ct{118};
t1250 = ct{119};
t1252 = ct{120};
t1253 = ct{121};
t1255 = ct{122};
t1260 = ct{123};
t1261 = ct{124};
t1262 = ct{125};
t1264 = ct{126};
t1265 = ct{127};
t1268 = ct{128};
t1280 = ct{129};
t1283 = ct{130};
t1291 = ct{131};
t130 = ct{132};
t1301 = ct{133};
t1302 = ct{134};
t1303 = ct{135};
t1304 = ct{136};
t1305 = ct{137};
t1307 = ct{138};
t1309 = ct{139};
t1313 = ct{140};
t1322 = ct{141};
t1328 = ct{142};
t1331 = ct{143};
t1332 = ct{144};
t1334 = ct{145};
t1337 = ct{146};
t1338 = ct{147};
t134 = ct{148};
t1343 = ct{149};
t1344 = ct{150};
t1345 = ct{151};
t1348 = ct{152};
t1352 = ct{153};
t1354 = ct{154};
t1355 = ct{155};
t1356 = ct{156};
t1360 = ct{157};
t1362 = ct{158};
t1365 = ct{159};
t1366 = ct{160};
t1368 = ct{161};
t1370 = ct{162};
t1371 = ct{163};
t1373 = ct{164};
t1374 = ct{165};
t1378 = ct{166};
t1381 = ct{167};
t1382 = ct{168};
t1384 = ct{169};
t1386 = ct{170};
t1388 = ct{171};
t1389 = ct{172};
t1391 = ct{173};
t1393 = ct{174};
t1394 = ct{175};
t1395 = ct{176};
t1396 = ct{177};
t1397 = ct{178};
t1403 = ct{179};
t1406 = ct{180};
t1412 = ct{181};
t1413 = ct{182};
t1415 = ct{183};
t1416 = ct{184};
t1421 = ct{185};
t1426 = ct{186};
t1427 = ct{187};
t1430 = ct{188};
t1431 = ct{189};
t1433 = ct{190};
t1435 = ct{191};
t144 = ct{192};
t1441 = ct{193};
t1443 = ct{194};
t1444 = ct{195};
t1446 = ct{196};
t1453 = ct{197};
t1455 = ct{198};
t1456 = ct{199};
t1457 = ct{200};
t1458 = ct{201};
t1460 = ct{202};
t1463 = ct{203};
t1465 = ct{204};
t1466 = ct{205};
t1467 = ct{206};
t1468 = ct{207};
t1469 = ct{208};
t1470 = ct{209};
t1476 = ct{210};
t1479 = ct{211};
t1480 = ct{212};
t1481 = ct{213};
t1486 = ct{214};
t1487 = ct{215};
t1495 = ct{216};
t15 = ct{217};
t1505 = ct{218};
t1506 = ct{219};
t1508 = ct{220};
t1510 = ct{221};
t1512 = ct{222};
t1513 = ct{223};
t1516 = ct{224};
t1518 = ct{225};
t1521 = ct{226};
t1525 = ct{227};
t1526 = ct{228};
t1528 = ct{229};
t1529 = ct{230};
t1531 = ct{231};
t1535 = ct{232};
t1540 = ct{233};
t1543 = ct{234};
t1544 = ct{235};
t1546 = ct{236};
t1549 = ct{237};
t1551 = ct{238};
t1552 = ct{239};
t1558 = ct{240};
t1562 = ct{241};
t1563 = ct{242};
t1568 = ct{243};
t1575 = ct{244};
t1578 = ct{245};
t1581 = ct{246};
t1585 = ct{247};
t1586 = ct{248};
t1587 = ct{249};
t1590 = ct{250};
t1593 = ct{251};
t1595 = ct{252};
t1596 = ct{253};
t1597 = ct{254};
t1598 = ct{255};
t1599 = ct{256};
t1605 = ct{257};
t1609 = ct{258};
t161 = ct{259};
t1612 = ct{260};
t1618 = ct{261};
t1619 = ct{262};
t162 = ct{263};
t1620 = ct{264};
t1621 = ct{265};
t1624 = ct{266};
t1627 = ct{267};
t1628 = ct{268};
t1630 = ct{269};
t1633 = ct{270};
t1634 = ct{271};
t1635 = ct{272};
t1636 = ct{273};
t1637 = ct{274};
t1639 = ct{275};
t1640 = ct{276};
t1643 = ct{277};
t1645 = ct{278};
t1646 = ct{279};
t1650 = ct{280};
t1651 = ct{281};
t1652 = ct{282};
t1654 = ct{283};
t1655 = ct{284};
t1656 = ct{285};
t1657 = ct{286};
t1659 = ct{287};
t1660 = ct{288};
t1661 = ct{289};
t1663 = ct{290};
t1664 = ct{291};
t1665 = ct{292};
t1667 = ct{293};
t1669 = ct{294};
t1672 = ct{295};
t1674 = ct{296};
t1675 = ct{297};
t1676 = ct{298};
t1678 = ct{299};
t1679 = ct{300};
t1680 = ct{301};
t1681 = ct{302};
t1682 = ct{303};
t1683 = ct{304};
t1685 = ct{305};
t1691 = ct{306};
t1692 = ct{307};
t1693 = ct{308};
t1694 = ct{309};
t1695 = ct{310};
t1696 = ct{311};
t1698 = ct{312};
t1699 = ct{313};
t1700 = ct{314};
t1701 = ct{315};
t1702 = ct{316};
t1703 = ct{317};
t1705 = ct{318};
t1706 = ct{319};
t1716 = ct{320};
t1718 = ct{321};
t1719 = ct{322};
t1720 = ct{323};
t1721 = ct{324};
t1722 = ct{325};
t1723 = ct{326};
t1725 = ct{327};
t1727 = ct{328};
t1730 = ct{329};
t1734 = ct{330};
t1735 = ct{331};
t1736 = ct{332};
t1737 = ct{333};
t1739 = ct{334};
t1740 = ct{335};
t1741 = ct{336};
t1742 = ct{337};
t1744 = ct{338};
t1746 = ct{339};
t1747 = ct{340};
t1748 = ct{341};
t1751 = ct{342};
t1752 = ct{343};
t1759 = ct{344};
t1761 = ct{345};
t1763 = ct{346};
t1764 = ct{347};
t1765 = ct{348};
t1771 = ct{349};
t1774 = ct{350};
t1777 = ct{351};
t1778 = ct{352};
t1779 = ct{353};
t1780 = ct{354};
t1781 = ct{355};
t1782 = ct{356};
t1783 = ct{357};
t1784 = ct{358};
t1785 = ct{359};
t1786 = ct{360};
t1787 = ct{361};
t1788 = ct{362};
t1789 = ct{363};
t1790 = ct{364};
t1792 = ct{365};
t1798 = ct{366};
t1799 = ct{367};
t1800 = ct{368};
t1801 = ct{369};
t1802 = ct{370};
t1806 = ct{371};
t1809 = ct{372};
t1810 = ct{373};
t1813 = ct{374};
t1820 = ct{375};
t1821 = ct{376};
t1832 = ct{377};
t1836 = ct{378};
t1840 = ct{379};
t1841 = ct{380};
t1843 = ct{381};
t1846 = ct{382};
t1851 = ct{383};
t1853 = ct{384};
t1855 = ct{385};
t1857 = ct{386};
t1858 = ct{387};
t1859 = ct{388};
t1860 = ct{389};
t1865 = ct{390};
t1866 = ct{391};
t1867 = ct{392};
t1874 = ct{393};
t1875 = ct{394};
t1882 = ct{395};
t1883 = ct{396};
t1888 = ct{397};
t1890 = ct{398};
t1895 = ct{399};
t1896 = ct{400};
t1898 = ct{401};
t1899 = ct{402};
t1900 = ct{403};
t1904 = ct{404};
t1905 = ct{405};
t1907 = ct{406};
t1908 = ct{407};
t1909 = ct{408};
t1910 = ct{409};
t1912 = ct{410};
t1915 = ct{411};
t1916 = ct{412};
t1917 = ct{413};
t1918 = ct{414};
t1928 = ct{415};
t1929 = ct{416};
t1930 = ct{417};
t1931 = ct{418};
t1932 = ct{419};
t1938 = ct{420};
t1939 = ct{421};
t1941 = ct{422};
t1942 = ct{423};
t1943 = ct{424};
t1945 = ct{425};
t1947 = ct{426};
t1948 = ct{427};
t195 = ct{428};
t1950 = ct{429};
t1951 = ct{430};
t1952 = ct{431};
t1956 = ct{432};
t1957 = ct{433};
t1959 = ct{434};
t1961 = ct{435};
t1962 = ct{436};
t1963 = ct{437};
t1964 = ct{438};
t1965 = ct{439};
t1966 = ct{440};
t1969 = ct{441};
t197 = ct{442};
t1970 = ct{443};
t1971 = ct{444};
t1973 = ct{445};
t1974 = ct{446};
t1976 = ct{447};
t1977 = ct{448};
t1979 = ct{449};
t1981 = ct{450};
t1982 = ct{451};
t1983 = ct{452};
t1993 = ct{453};
t1997 = ct{454};
t1998 = ct{455};
t1999 = ct{456};
t2 = ct{457};
t2000 = ct{458};
t2002 = ct{459};
t2004 = ct{460};
t2007 = ct{461};
t2008 = ct{462};
t2009 = ct{463};
t2011 = ct{464};
t2012 = ct{465};
t2013 = ct{466};
t2015 = ct{467};
t2016 = ct{468};
t2017 = ct{469};
t2018 = ct{470};
t2020 = ct{471};
t2023 = ct{472};
t2024 = ct{473};
t2025 = ct{474};
t2032 = ct{475};
t2033 = ct{476};
t2037 = ct{477};
t2038 = ct{478};
t2042 = ct{479};
t2045 = ct{480};
t2046 = ct{481};
t2047 = ct{482};
t2049 = ct{483};
t2050 = ct{484};
t2057 = ct{485};
t2058 = ct{486};
t2059 = ct{487};
t2061 = ct{488};
t2062 = ct{489};
t2064 = ct{490};
t2065 = ct{491};
t2066 = ct{492};
t2067 = ct{493};
t2068 = ct{494};
t2069 = ct{495};
t2072 = ct{496};
t2075 = ct{497};
t2076 = ct{498};
t2081 = ct{499};
t2082 = ct{500};
t2083 = ct{501};
t2086 = ct{502};
t2087 = ct{503};
t2088 = ct{504};
t2089 = ct{505};
t2090 = ct{506};
t2091 = ct{507};
t2094 = ct{508};
t2096 = ct{509};
t2102 = ct{510};
t2104 = ct{511};
t2106 = ct{512};
t2107 = ct{513};
t2108 = ct{514};
t2109 = ct{515};
t2110 = ct{516};
t2111 = ct{517};
t2113 = ct{518};
t2117 = ct{519};
t2118 = ct{520};
t2119 = ct{521};
t2123 = ct{522};
t2130 = ct{523};
t2131 = ct{524};
t2134 = ct{525};
t2135 = ct{526};
t2137 = ct{527};
t2139 = ct{528};
t214 = ct{529};
t2141 = ct{530};
t2143 = ct{531};
t2144 = ct{532};
t2147 = ct{533};
t2148 = ct{534};
t2150 = ct{535};
t2151 = ct{536};
t2152 = ct{537};
t2153 = ct{538};
t2154 = ct{539};
t2155 = ct{540};
t2156 = ct{541};
t2157 = ct{542};
t2158 = ct{543};
t2161 = ct{544};
t2165 = ct{545};
t2171 = ct{546};
t2172 = ct{547};
t2174 = ct{548};
t2175 = ct{549};
t2178 = ct{550};
t2179 = ct{551};
t2181 = ct{552};
t2182 = ct{553};
t2183 = ct{554};
t2186 = ct{555};
t2188 = ct{556};
t2189 = ct{557};
t2190 = ct{558};
t2191 = ct{559};
t2192 = ct{560};
t2196 = ct{561};
t2197 = ct{562};
t2202 = ct{563};
t2203 = ct{564};
t2206 = ct{565};
t2208 = ct{566};
t2210 = ct{567};
t2211 = ct{568};
t2212 = ct{569};
t2215 = ct{570};
t2216 = ct{571};
t2217 = ct{572};
t2218 = ct{573};
t2220 = ct{574};
t2221 = ct{575};
t2222 = ct{576};
t2223 = ct{577};
t2225 = ct{578};
t2227 = ct{579};
t2229 = ct{580};
t2230 = ct{581};
t2237 = ct{582};
t2240 = ct{583};
t2241 = ct{584};
t2242 = ct{585};
t2243 = ct{586};
t2245 = ct{587};
t2247 = ct{588};
t2248 = ct{589};
t2249 = ct{590};
t2251 = ct{591};
t2252 = ct{592};
t2253 = ct{593};
t2254 = ct{594};
t2255 = ct{595};
t2257 = ct{596};
t2259 = ct{597};
t2260 = ct{598};
t2262 = ct{599};
t2263 = ct{600};
t2268 = ct{601};
t2269 = ct{602};
t2271 = ct{603};
t2274 = ct{604};
t2276 = ct{605};
t2281 = ct{606};
t2282 = ct{607};
t2285 = ct{608};
t2286 = ct{609};
t2287 = ct{610};
t2288 = ct{611};
t2289 = ct{612};
t2290 = ct{613};
t2293 = ct{614};
t2305 = ct{615};
t2307 = ct{616};
t2308 = ct{617};
t2312 = ct{618};
t2316 = ct{619};
t2317 = ct{620};
t2318 = ct{621};
t2319 = ct{622};
t2320 = ct{623};
t2321 = ct{624};
t2322 = ct{625};
t2324 = ct{626};
t2325 = ct{627};
t2329 = ct{628};
t2334 = ct{629};
t2336 = ct{630};
t2338 = ct{631};
t2339 = ct{632};
t2340 = ct{633};
t2341 = ct{634};
t2342 = ct{635};
t2343 = ct{636};
t2345 = ct{637};
t2346 = ct{638};
t2347 = ct{639};
t2348 = ct{640};
t2349 = ct{641};
t2350 = ct{642};
t2352 = ct{643};
t2354 = ct{644};
t2356 = ct{645};
t2358 = ct{646};
t2360 = ct{647};
t2361 = ct{648};
t2362 = ct{649};
t2363 = ct{650};
t2364 = ct{651};
t2368 = ct{652};
t2376 = ct{653};
t2382 = ct{654};
t2385 = ct{655};
t2386 = ct{656};
t2387 = ct{657};
t2388 = ct{658};
t2389 = ct{659};
t2390 = ct{660};
t2391 = ct{661};
t2392 = ct{662};
t2397 = ct{663};
t2399 = ct{664};
t24 = ct{665};
t2400 = ct{666};
t2401 = ct{667};
t2404 = ct{668};
t2406 = ct{669};
t2407 = ct{670};
t2408 = ct{671};
t2409 = ct{672};
t2410 = ct{673};
t2411 = ct{674};
t2412 = ct{675};
t2413 = ct{676};
t2419 = ct{677};
t2420 = ct{678};
t2422 = ct{679};
t2426 = ct{680};
t2427 = ct{681};
t2428 = ct{682};
t2429 = ct{683};
t2430 = ct{684};
t2431 = ct{685};
t2433 = ct{686};
t2434 = ct{687};
t2435 = ct{688};
t2436 = ct{689};
t2437 = ct{690};
t2438 = ct{691};
t2447 = ct{692};
t2449 = ct{693};
t2458 = ct{694};
t2461 = ct{695};
t2462 = ct{696};
t2463 = ct{697};
t2465 = ct{698};
t2468 = ct{699};
t2470 = ct{700};
t2471 = ct{701};
t2472 = ct{702};
t2474 = ct{703};
t2476 = ct{704};
t2479 = ct{705};
t2480 = ct{706};
t2483 = ct{707};
t2485 = ct{708};
t2486 = ct{709};
t2487 = ct{710};
t2488 = ct{711};
t2489 = ct{712};
t2492 = ct{713};
t2495 = ct{714};
t2496 = ct{715};
t25 = ct{716};
t2501 = ct{717};
t2503 = ct{718};
t2504 = ct{719};
t2512 = ct{720};
t2513 = ct{721};
t2514 = ct{722};
t2515 = ct{723};
t2516 = ct{724};
t2518 = ct{725};
t2522 = ct{726};
t2523 = ct{727};
t2524 = ct{728};
t2525 = ct{729};
t2526 = ct{730};
t2527 = ct{731};
t2528 = ct{732};
t2530 = ct{733};
t2531 = ct{734};
t2533 = ct{735};
t2534 = ct{736};
t2535 = ct{737};
t2536 = ct{738};
t2543 = ct{739};
t2545 = ct{740};
t2546 = ct{741};
t2547 = ct{742};
t2550 = ct{743};
t2551 = ct{744};
t2552 = ct{745};
t2555 = ct{746};
t2557 = ct{747};
t2559 = ct{748};
t2560 = ct{749};
t2562 = ct{750};
t2563 = ct{751};
t2564 = ct{752};
t2567 = ct{753};
t2568 = ct{754};
t2569 = ct{755};
t2570 = ct{756};
t2571 = ct{757};
t2573 = ct{758};
t2574 = ct{759};
t2576 = ct{760};
t2577 = ct{761};
t2578 = ct{762};
t2579 = ct{763};
t2581 = ct{764};
t2582 = ct{765};
t2584 = ct{766};
t2585 = ct{767};
t2587 = ct{768};
t2589 = ct{769};
t259 = ct{770};
t2590 = ct{771};
t2591 = ct{772};
t2597 = ct{773};
t2598 = ct{774};
t2599 = ct{775};
t26 = ct{776};
t260 = ct{777};
t2600 = ct{778};
t2605 = ct{779};
t2607 = ct{780};
t2613 = ct{781};
t2616 = ct{782};
t2617 = ct{783};
t2619 = ct{784};
t2621 = ct{785};
t2623 = ct{786};
t2624 = ct{787};
t2627 = ct{788};
t2629 = ct{789};
t2630 = ct{790};
t2632 = ct{791};
t2636 = ct{792};
t2637 = ct{793};
t2638 = ct{794};
t2646 = ct{795};
t2648 = ct{796};
t2650 = ct{797};
t2652 = ct{798};
t2655 = ct{799};
t2657 = ct{800};
t2659 = ct{801};
t2660 = ct{802};
t2661 = ct{803};
t2662 = ct{804};
t2663 = ct{805};
t2665 = ct{806};
t2666 = ct{807};
t2667 = ct{808};
t2668 = ct{809};
t2669 = ct{810};
t2671 = ct{811};
t2673 = ct{812};
t2677 = ct{813};
t2678 = ct{814};
t2679 = ct{815};
t2682 = ct{816};
t2684 = ct{817};
t2688 = ct{818};
t2689 = ct{819};
t2692 = ct{820};
t2696 = ct{821};
t2698 = ct{822};
t2699 = ct{823};
t27 = ct{824};
t2700 = ct{825};
t2705 = ct{826};
t2706 = ct{827};
t2707 = ct{828};
t2708 = ct{829};
t2710 = ct{830};
t2712 = ct{831};
t2715 = ct{832};
t2717 = ct{833};
t2718 = ct{834};
t2722 = ct{835};
t2723 = ct{836};
t2725 = ct{837};
t2726 = ct{838};
t2727 = ct{839};
t2728 = ct{840};
t2730 = ct{841};
t2733 = ct{842};
t2734 = ct{843};
t2735 = ct{844};
t2736 = ct{845};
t2737 = ct{846};
t2738 = ct{847};
t2740 = ct{848};
t2742 = ct{849};
t2743 = ct{850};
t2744 = ct{851};
t2746 = ct{852};
t2749 = ct{853};
t2750 = ct{854};
t2751 = ct{855};
t2752 = ct{856};
t2754 = ct{857};
t2756 = ct{858};
t2758 = ct{859};
t2759 = ct{860};
t276 = ct{861};
t2760 = ct{862};
t2761 = ct{863};
t2763 = ct{864};
t2764 = ct{865};
t2765 = ct{866};
t2766 = ct{867};
t2768 = ct{868};
t277 = ct{869};
t2772 = ct{870};
t2774 = ct{871};
t2776 = ct{872};
t2778 = ct{873};
t2779 = ct{874};
t2781 = ct{875};
t2783 = ct{876};
t2785 = ct{877};
t2786 = ct{878};
t2787 = ct{879};
t2788 = ct{880};
t2790 = ct{881};
t2791 = ct{882};
t2792 = ct{883};
t2794 = ct{884};
t2796 = ct{885};
t2797 = ct{886};
t2798 = ct{887};
t2799 = ct{888};
t2800 = ct{889};
t2802 = ct{890};
t2803 = ct{891};
t2804 = ct{892};
t2805 = ct{893};
t2806 = ct{894};
t2808 = ct{895};
t2811 = ct{896};
t2813 = ct{897};
t2814 = ct{898};
t2816 = ct{899};
t2817 = ct{900};
t2818 = ct{901};
t2819 = ct{902};
t2821 = ct{903};
t2823 = ct{904};
t2824 = ct{905};
t2825 = ct{906};
t2829 = ct{907};
t283 = ct{908};
t2831 = ct{909};
t2832 = ct{910};
t2833 = ct{911};
t2834 = ct{912};
t2836 = ct{913};
t2837 = ct{914};
t2838 = ct{915};
t2839 = ct{916};
t284 = ct{917};
t2841 = ct{918};
t2842 = ct{919};
t2843 = ct{920};
t2844 = ct{921};
t2845 = ct{922};
t2846 = ct{923};
t2847 = ct{924};
t2849 = ct{925};
t285 = ct{926};
t2853 = ct{927};
t2857 = ct{928};
t2858 = ct{929};
t2859 = ct{930};
t286 = ct{931};
t2860 = ct{932};
t2861 = ct{933};
t2864 = ct{934};
t2865 = ct{935};
t2868 = ct{936};
t287 = ct{937};
t2870 = ct{938};
t2871 = ct{939};
t2872 = ct{940};
t2874 = ct{941};
t2875 = ct{942};
t2876 = ct{943};
t2877 = ct{944};
t2878 = ct{945};
t2879 = ct{946};
t288 = ct{947};
t2882 = ct{948};
t2883 = ct{949};
t2884 = ct{950};
t2886 = ct{951};
t2887 = ct{952};
t2889 = ct{953};
t289 = ct{954};
t2890 = ct{955};
t2893 = ct{956};
t2896 = ct{957};
t2897 = ct{958};
t2898 = ct{959};
t2899 = ct{960};
t290 = ct{961};
t2903 = ct{962};
t2909 = ct{963};
t291 = ct{964};
t2912 = ct{965};
t2913 = ct{966};
t2914 = ct{967};
t2915 = ct{968};
t2916 = ct{969};
t2917 = ct{970};
t2918 = ct{971};
t2919 = ct{972};
t292 = ct{973};
t2920 = ct{974};
t2921 = ct{975};
t2926 = ct{976};
t2927 = ct{977};
t2928 = ct{978};
t293 = ct{979};
t2930 = ct{980};
t2932 = ct{981};
t2936 = ct{982};
t2937 = ct{983};
t2938 = ct{984};
t294 = ct{985};
t2941 = ct{986};
t2942 = ct{987};
t2943 = ct{988};
t2944 = ct{989};
t2945 = ct{990};
t2946 = ct{991};
t2949 = ct{992};
t2950 = ct{993};
t2952 = ct{994};
t2954 = ct{995};
t2956 = ct{996};
t2959 = ct{997};
t2960 = ct{998};
t2962 = ct{999};
t2963 = ct{1000};
t2964 = ct{1001};
t2965 = ct{1002};
t2966 = ct{1003};
t2970 = ct{1004};
t2972 = ct{1005};
t2973 = ct{1006};
t2976 = ct{1007};
t2977 = ct{1008};
t2978 = ct{1009};
t2979 = ct{1010};
t2981 = ct{1011};
t2982 = ct{1012};
t2985 = ct{1013};
t2988 = ct{1014};
t2989 = ct{1015};
t2992 = ct{1016};
t2994 = ct{1017};
t2995 = ct{1018};
t2996 = ct{1019};
t2997 = ct{1020};
t2998 = ct{1021};
t3 = ct{1022};
t3004 = ct{1023};
t3006 = ct{1024};
t3007 = ct{1025};
t3008 = ct{1026};
t3009 = ct{1027};
t3011 = ct{1028};
t3012 = ct{1029};
t3016 = ct{1030};
t3017 = ct{1031};
t3019 = ct{1032};
t3022 = ct{1033};
t3027 = ct{1034};
t3030 = ct{1035};
t3031 = ct{1036};
t3032 = ct{1037};
t3033 = ct{1038};
t3034 = ct{1039};
t3035 = ct{1040};
t3037 = ct{1041};
t3038 = ct{1042};
t304 = ct{1043};
t3040 = ct{1044};
t3041 = ct{1045};
t3042 = ct{1046};
t3043 = ct{1047};
t3047 = ct{1048};
t3049 = ct{1049};
t3050 = ct{1050};
t3051 = ct{1051};
t3054 = ct{1052};
t3059 = ct{1053};
t3060 = ct{1054};
t3061 = ct{1055};
t3062 = ct{1056};
t3063 = ct{1057};
t3064 = ct{1058};
t3070 = ct{1059};
t3075 = ct{1060};
t3076 = ct{1061};
t3078 = ct{1062};
t3080 = ct{1063};
t3082 = ct{1064};
t3083 = ct{1065};
t3084 = ct{1066};
t3085 = ct{1067};
t3086 = ct{1068};
t3087 = ct{1069};
t3089 = ct{1070};
t3090 = ct{1071};
t3091 = ct{1072};
t3092 = ct{1073};
t3093 = ct{1074};
t3094 = ct{1075};
t3096 = ct{1076};
t3097 = ct{1077};
t3098 = ct{1078};
t3100 = ct{1079};
t3103 = ct{1080};
t3105 = ct{1081};
t3106 = ct{1082};
t3107 = ct{1083};
t3108 = ct{1084};
t3109 = ct{1085};
t3110 = ct{1086};
t3112 = ct{1087};
t3113 = ct{1088};
t3117 = ct{1089};
t3121 = ct{1090};
t3122 = ct{1091};
t3127 = ct{1092};
t3128 = ct{1093};
t3131 = ct{1094};
t3132 = ct{1095};
t3134 = ct{1096};
t3135 = ct{1097};
t3138 = ct{1098};
t3139 = ct{1099};
t3145 = ct{1100};
t3146 = ct{1101};
t3147 = ct{1102};
t3149 = ct{1103};
t3151 = ct{1104};
t3153 = ct{1105};
t3155 = ct{1106};
t3156 = ct{1107};
t3158 = ct{1108};
t3160 = ct{1109};
t3161 = ct{1110};
t3162 = ct{1111};
t3163 = ct{1112};
t3166 = ct{1113};
t3167 = ct{1114};
t3169 = ct{1115};
t3170 = ct{1116};
t3171 = ct{1117};
t3173 = ct{1118};
t3174 = ct{1119};
t3176 = ct{1120};
t3177 = ct{1121};
t3178 = ct{1122};
t3179 = ct{1123};
t3180 = ct{1124};
t3183 = ct{1125};
t3184 = ct{1126};
t3185 = ct{1127};
t3186 = ct{1128};
t3187 = ct{1129};
t3190 = ct{1130};
t3192 = ct{1131};
t3193 = ct{1132};
t3196 = ct{1133};
t3199 = ct{1134};
t3203 = ct{1135};
t3204 = ct{1136};
t3206 = ct{1137};
t3207 = ct{1138};
t3210 = ct{1139};
t3212 = ct{1140};
t3213 = ct{1141};
t3214 = ct{1142};
t3215 = ct{1143};
t3216 = ct{1144};
t3217 = ct{1145};
t3218 = ct{1146};
t3221 = ct{1147};
t3222 = ct{1148};
t3223 = ct{1149};
t3226 = ct{1150};
t3230 = ct{1151};
t3231 = ct{1152};
t3232 = ct{1153};
t3233 = ct{1154};
t3235 = ct{1155};
t3236 = ct{1156};
t3239 = ct{1157};
t3241 = ct{1158};
t3243 = ct{1159};
t3244 = ct{1160};
t3245 = ct{1161};
t3247 = ct{1162};
t3248 = ct{1163};
t3250 = ct{1164};
t3251 = ct{1165};
t3252 = ct{1166};
t3254 = ct{1167};
t3256 = ct{1168};
t3257 = ct{1169};
t3258 = ct{1170};
t3260 = ct{1171};
t3261 = ct{1172};
t3262 = ct{1173};
t3263 = ct{1174};
t3265 = ct{1175};
t3266 = ct{1176};
t3267 = ct{1177};
t3270 = ct{1178};
t3271 = ct{1179};
t3272 = ct{1180};
t3273 = ct{1181};
t3276 = ct{1182};
t3277 = ct{1183};
t3278 = ct{1184};
t3279 = ct{1185};
t3280 = ct{1186};
t3284 = ct{1187};
t3285 = ct{1188};
t3286 = ct{1189};
t3287 = ct{1190};
t3289 = ct{1191};
t3290 = ct{1192};
t3296 = ct{1193};
t3299 = ct{1194};
t3300 = ct{1195};
t3301 = ct{1196};
t3302 = ct{1197};
t3303 = ct{1198};
t3304 = ct{1199};
t3305 = ct{1200};
t3306 = ct{1201};
t3307 = ct{1202};
t3308 = ct{1203};
t3311 = ct{1204};
t3312 = ct{1205};
t3313 = ct{1206};
t3314 = ct{1207};
t3315 = ct{1208};
t3317 = ct{1209};
t3319 = ct{1210};
t3320 = ct{1211};
t3321 = ct{1212};
t3322 = ct{1213};
t3325 = ct{1214};
t3326 = ct{1215};
t3327 = ct{1216};
t3328 = ct{1217};
t3329 = ct{1218};
t3330 = ct{1219};
t3331 = ct{1220};
t3332 = ct{1221};
t3333 = ct{1222};
t3334 = ct{1223};
t3335 = ct{1224};
t3336 = ct{1225};
t3337 = ct{1226};
t3338 = ct{1227};
t3339 = ct{1228};
t3340 = ct{1229};
t3341 = ct{1230};
t3342 = ct{1231};
t3343 = ct{1232};
t3344 = ct{1233};
t3347 = ct{1234};
t3349 = ct{1235};
t3351 = ct{1236};
t3354 = ct{1237};
t3357 = ct{1238};
t3359 = ct{1239};
t3360 = ct{1240};
t3367 = ct{1241};
t3368 = ct{1242};
t3372 = ct{1243};
t3375 = ct{1244};
t3376 = ct{1245};
t3377 = ct{1246};
t3378 = ct{1247};
t3379 = ct{1248};
t3380 = ct{1249};
t3381 = ct{1250};
t3384 = ct{1251};
t3385 = ct{1252};
t3386 = ct{1253};
t3387 = ct{1254};
t3388 = ct{1255};
t3390 = ct{1256};
t3391 = ct{1257};
t3392 = ct{1258};
t3397 = ct{1259};
t3399 = ct{1260};
t3402 = ct{1261};
t3403 = ct{1262};
t3404 = ct{1263};
t3405 = ct{1264};
t3406 = ct{1265};
t3407 = ct{1266};
t3409 = ct{1267};
t3411 = ct{1268};
t3412 = ct{1269};
t3413 = ct{1270};
t3414 = ct{1271};
t3415 = ct{1272};
t3416 = ct{1273};
t3419 = ct{1274};
t3423 = ct{1275};
t3424 = ct{1276};
t3427 = ct{1277};
t3429 = ct{1278};
t3431 = ct{1279};
t3432 = ct{1280};
t3433 = ct{1281};
t3437 = ct{1282};
t3438 = ct{1283};
t3439 = ct{1284};
t3440 = ct{1285};
t3441 = ct{1286};
t3442 = ct{1287};
t3443 = ct{1288};
t3444 = ct{1289};
t3445 = ct{1290};
t3446 = ct{1291};
t3447 = ct{1292};
t3448 = ct{1293};
t3449 = ct{1294};
t3454 = ct{1295};
t3457 = ct{1296};
t3458 = ct{1297};
t3459 = ct{1298};
t3460 = ct{1299};
t3463 = ct{1300};
t3465 = ct{1301};
t3466 = ct{1302};
t3467 = ct{1303};
t3469 = ct{1304};
t3471 = ct{1305};
t3473 = ct{1306};
t3474 = ct{1307};
t3475 = ct{1308};
t3476 = ct{1309};
t3478 = ct{1310};
t3480 = ct{1311};
t3481 = ct{1312};
t3482 = ct{1313};
t3483 = ct{1314};
t3484 = ct{1315};
t3485 = ct{1316};
t3486 = ct{1317};
t3487 = ct{1318};
t3488 = ct{1319};
t3489 = ct{1320};
t3490 = ct{1321};
t3491 = ct{1322};
t3492 = ct{1323};
t3494 = ct{1324};
t3497 = ct{1325};
t3499 = ct{1326};
t3500 = ct{1327};
t3501 = ct{1328};
t3504 = ct{1329};
t3506 = ct{1330};
t3508 = ct{1331};
t3510 = ct{1332};
t3512 = ct{1333};
t3513 = ct{1334};
t3515 = ct{1335};
t3516 = ct{1336};
t3517 = ct{1337};
t3521 = ct{1338};
t3522 = ct{1339};
t3523 = ct{1340};
t3524 = ct{1341};
t3526 = ct{1342};
t3528 = ct{1343};
t3529 = ct{1344};
t3530 = ct{1345};
t3531 = ct{1346};
t3534 = ct{1347};
t3535 = ct{1348};
t3536 = ct{1349};
t3538 = ct{1350};
t3539 = ct{1351};
t3540 = ct{1352};
t3541 = ct{1353};
t3542 = ct{1354};
t3543 = ct{1355};
t3544 = ct{1356};
t3545 = ct{1357};
t3547 = ct{1358};
t3548 = ct{1359};
t3550 = ct{1360};
t3552 = ct{1361};
t3553 = ct{1362};
t3554 = ct{1363};
t3555 = ct{1364};
t3556 = ct{1365};
t3557 = ct{1366};
t3558 = ct{1367};
t3559 = ct{1368};
t3563 = ct{1369};
t3565 = ct{1370};
t3570 = ct{1371};
t3571 = ct{1372};
t3575 = ct{1373};
t3576 = ct{1374};
t3578 = ct{1375};
t3579 = ct{1376};
t3581 = ct{1377};
t3582 = ct{1378};
t3583 = ct{1379};
t3584 = ct{1380};
t3587 = ct{1381};
t3588 = ct{1382};
t3591 = ct{1383};
t3594 = ct{1384};
t3595 = ct{1385};
t3596 = ct{1386};
t3597 = ct{1387};
t3598 = ct{1388};
t3600 = ct{1389};
t3602 = ct{1390};
t3603 = ct{1391};
t3605 = ct{1392};
t3609 = ct{1393};
t3610 = ct{1394};
t3611 = ct{1395};
t3613 = ct{1396};
t3614 = ct{1397};
t3615 = ct{1398};
t3616 = ct{1399};
t3617 = ct{1400};
t3618 = ct{1401};
t3619 = ct{1402};
t3620 = ct{1403};
t3621 = ct{1404};
t3622 = ct{1405};
t3623 = ct{1406};
t3624 = ct{1407};
t3627 = ct{1408};
t3629 = ct{1409};
t3630 = ct{1410};
t3632 = ct{1411};
t3634 = ct{1412};
t3637 = ct{1413};
t3638 = ct{1414};
t3639 = ct{1415};
t3643 = ct{1416};
t3644 = ct{1417};
t3646 = ct{1418};
t3647 = ct{1419};
t3648 = ct{1420};
t3649 = ct{1421};
t3651 = ct{1422};
t3652 = ct{1423};
t3653 = ct{1424};
t3654 = ct{1425};
t3655 = ct{1426};
t3657 = ct{1427};
t3659 = ct{1428};
t3661 = ct{1429};
t3666 = ct{1430};
t3667 = ct{1431};
t3668 = ct{1432};
t3670 = ct{1433};
t3671 = ct{1434};
t3672 = ct{1435};
t3673 = ct{1436};
t3674 = ct{1437};
t3677 = ct{1438};
t3678 = ct{1439};
t3679 = ct{1440};
t3680 = ct{1441};
t3681 = ct{1442};
t3682 = ct{1443};
t3683 = ct{1444};
t3684 = ct{1445};
t3685 = ct{1446};
t3686 = ct{1447};
t3687 = ct{1448};
t3689 = ct{1449};
t3690 = ct{1450};
t3693 = ct{1451};
t3697 = ct{1452};
t3698 = ct{1453};
t3699 = ct{1454};
t3700 = ct{1455};
t3701 = ct{1456};
t3702 = ct{1457};
t3704 = ct{1458};
t3708 = ct{1459};
t3709 = ct{1460};
t3710 = ct{1461};
t3711 = ct{1462};
t3716 = ct{1463};
t3719 = ct{1464};
t3720 = ct{1465};
t3721 = ct{1466};
t3722 = ct{1467};
t3723 = ct{1468};
t3724 = ct{1469};
t3730 = ct{1470};
t3735 = ct{1471};
t3736 = ct{1472};
t3738 = ct{1473};
t3739 = ct{1474};
t3741 = ct{1475};
t3742 = ct{1476};
t3744 = ct{1477};
t3745 = ct{1478};
t3746 = ct{1479};
t3747 = ct{1480};
t3748 = ct{1481};
t3749 = ct{1482};
t3750 = ct{1483};
t3755 = ct{1484};
t3756 = ct{1485};
t3757 = ct{1486};
t3758 = ct{1487};
t3759 = ct{1488};
t376 = ct{1489};
t3760 = ct{1490};
t3761 = ct{1491};
t3762 = ct{1492};
t3764 = ct{1493};
t3765 = ct{1494};
t3766 = ct{1495};
t3767 = ct{1496};
t3769 = ct{1497};
t377 = ct{1498};
t3770 = ct{1499};
t3771 = ct{1500};
t3772 = ct{1501};
t3773 = ct{1502};
t3774 = ct{1503};
t3775 = ct{1504};
t3777 = ct{1505};
t3779 = ct{1506};
t3780 = ct{1507};
t3784 = ct{1508};
t3785 = ct{1509};
t3787 = ct{1510};
t3789 = ct{1511};
t3791 = ct{1512};
t3792 = ct{1513};
t3793 = ct{1514};
t3794 = ct{1515};
t3795 = ct{1516};
t3797 = ct{1517};
t3798 = ct{1518};
t3799 = ct{1519};
t3800 = ct{1520};
t3802 = ct{1521};
t3804 = ct{1522};
t3805 = ct{1523};
t3806 = ct{1524};
t3807 = ct{1525};
t3808 = ct{1526};
t3809 = ct{1527};
t381 = ct{1528};
t3811 = ct{1529};
t3812 = ct{1530};
t3814 = ct{1531};
t3815 = ct{1532};
t3817 = ct{1533};
t3818 = ct{1534};
t3819 = ct{1535};
t382 = ct{1536};
t3820 = ct{1537};
t3823 = ct{1538};
t3824 = ct{1539};
t3825 = ct{1540};
t3826 = ct{1541};
t3828 = ct{1542};
t3829 = ct{1543};
t383 = ct{1544};
t3831 = ct{1545};
t3832 = ct{1546};
t3833 = ct{1547};
t3834 = ct{1548};
t3836 = ct{1549};
t3837 = ct{1550};
t3838 = ct{1551};
t3840 = ct{1552};
t3841 = ct{1553};
t3842 = ct{1554};
t3845 = ct{1555};
t3846 = ct{1556};
t3847 = ct{1557};
t3848 = ct{1558};
t3849 = ct{1559};
t3850 = ct{1560};
t3851 = ct{1561};
t3854 = ct{1562};
t3855 = ct{1563};
t3856 = ct{1564};
t3858 = ct{1565};
t3859 = ct{1566};
t3860 = ct{1567};
t3861 = ct{1568};
t3862 = ct{1569};
t3867 = ct{1570};
t3868 = ct{1571};
t3870 = ct{1572};
t3871 = ct{1573};
t3872 = ct{1574};
t3873 = ct{1575};
t3876 = ct{1576};
t3879 = ct{1577};
t3880 = ct{1578};
t3882 = ct{1579};
t3883 = ct{1580};
t3885 = ct{1581};
t3886 = ct{1582};
t3887 = ct{1583};
t3888 = ct{1584};
t3889 = ct{1585};
t3890 = ct{1586};
t3891 = ct{1587};
t3892 = ct{1588};
t3893 = ct{1589};
t3894 = ct{1590};
t3896 = ct{1591};
t3898 = ct{1592};
t390 = ct{1593};
t3900 = ct{1594};
t3902 = ct{1595};
t3903 = ct{1596};
t3906 = ct{1597};
t3907 = ct{1598};
t3908 = ct{1599};
t3909 = ct{1600};
t3911 = ct{1601};
t3913 = ct{1602};
t3914 = ct{1603};
t3915 = ct{1604};
t3916 = ct{1605};
t3918 = ct{1606};
t3919 = ct{1607};
t3921 = ct{1608};
t3923 = ct{1609};
t3925 = ct{1610};
t3926 = ct{1611};
t3928 = ct{1612};
t3929 = ct{1613};
t3930 = ct{1614};
t3931 = ct{1615};
t3932 = ct{1616};
t3933 = ct{1617};
t3934 = ct{1618};
t3936 = ct{1619};
t3937 = ct{1620};
t3938 = ct{1621};
t3939 = ct{1622};
t394 = ct{1623};
t3940 = ct{1624};
t3943 = ct{1625};
t3944 = ct{1626};
t3945 = ct{1627};
t3947 = ct{1628};
t3948 = ct{1629};
t3949 = ct{1630};
t3950 = ct{1631};
t3951 = ct{1632};
t3952 = ct{1633};
t3953 = ct{1634};
t3954 = ct{1635};
t3955 = ct{1636};
t3956 = ct{1637};
t3957 = ct{1638};
t3958 = ct{1639};
t3959 = ct{1640};
t3960 = ct{1641};
t3961 = ct{1642};
t3962 = ct{1643};
t3964 = ct{1644};
t3965 = ct{1645};
t3966 = ct{1646};
t3967 = ct{1647};
t3969 = ct{1648};
t3971 = ct{1649};
t3974 = ct{1650};
t3975 = ct{1651};
t3976 = ct{1652};
t3977 = ct{1653};
t3979 = ct{1654};
t3980 = ct{1655};
t3981 = ct{1656};
t3982 = ct{1657};
t3983 = ct{1658};
t3984 = ct{1659};
t3985 = ct{1660};
t3986 = ct{1661};
t3988 = ct{1662};
t3989 = ct{1663};
t3991 = ct{1664};
t3992 = ct{1665};
t3993 = ct{1666};
t3995 = ct{1667};
t3996 = ct{1668};
t3998 = ct{1669};
t4 = ct{1670};
t4000 = ct{1671};
t4001 = ct{1672};
t4003 = ct{1673};
t4005 = ct{1674};
t4006 = ct{1675};
t4007 = ct{1676};
t4008 = ct{1677};
t4009 = ct{1678};
t4010 = ct{1679};
t4012 = ct{1680};
t4014 = ct{1681};
t4016 = ct{1682};
t4017 = ct{1683};
t4019 = ct{1684};
t4020 = ct{1685};
t4021 = ct{1686};
t4022 = ct{1687};
t4023 = ct{1688};
t4024 = ct{1689};
t4025 = ct{1690};
t4026 = ct{1691};
t4027 = ct{1692};
t4028 = ct{1693};
t4029 = ct{1694};
t4033 = ct{1695};
t4034 = ct{1696};
t4035 = ct{1697};
t4036 = ct{1698};
t4037 = ct{1699};
t4038 = ct{1700};
t4040 = ct{1701};
t4041 = ct{1702};
t4042 = ct{1703};
t4044 = ct{1704};
t4046 = ct{1705};
t4047 = ct{1706};
t4048 = ct{1707};
t4050 = ct{1708};
t4051 = ct{1709};
t4052 = ct{1710};
t4053 = ct{1711};
t4054 = ct{1712};
t4056 = ct{1713};
t4058 = ct{1714};
t4059 = ct{1715};
t4061 = ct{1716};
t4062 = ct{1717};
t4064 = ct{1718};
t4065 = ct{1719};
t4066 = ct{1720};
t4068 = ct{1721};
t4070 = ct{1722};
t4071 = ct{1723};
t4072 = ct{1724};
t4073 = ct{1725};
t4074 = ct{1726};
t4077 = ct{1727};
t4078 = ct{1728};
t4081 = ct{1729};
t4083 = ct{1730};
t4084 = ct{1731};
t4085 = ct{1732};
t4086 = ct{1733};
t4087 = ct{1734};
t4089 = ct{1735};
t4090 = ct{1736};
t4091 = ct{1737};
t4092 = ct{1738};
t4093 = ct{1739};
t4094 = ct{1740};
t4095 = ct{1741};
t4096 = ct{1742};
t4097 = ct{1743};
t4098 = ct{1744};
t4099 = ct{1745};
t410 = ct{1746};
t4100 = ct{1747};
t4104 = ct{1748};
t4105 = ct{1749};
t4107 = ct{1750};
t4108 = ct{1751};
t4109 = ct{1752};
t411 = ct{1753};
t4111 = ct{1754};
t4112 = ct{1755};
t4115 = ct{1756};
t4116 = ct{1757};
t4117 = ct{1758};
t4119 = ct{1759};
t412 = ct{1760};
t4120 = ct{1761};
t4121 = ct{1762};
t4122 = ct{1763};
t4126 = ct{1764};
t4129 = ct{1765};
t413 = ct{1766};
t4130 = ct{1767};
t4132 = ct{1768};
t4133 = ct{1769};
t4135 = ct{1770};
t4137 = ct{1771};
t4138 = ct{1772};
t4139 = ct{1773};
t414 = ct{1774};
t4140 = ct{1775};
t4141 = ct{1776};
t4143 = ct{1777};
t4144 = ct{1778};
t4145 = ct{1779};
t4147 = ct{1780};
t4148 = ct{1781};
t415 = ct{1782};
t4151 = ct{1783};
t4152 = ct{1784};
t4153 = ct{1785};
t4154 = ct{1786};
t4155 = ct{1787};
t4156 = ct{1788};
t4157 = ct{1789};
t4160 = ct{1790};
t4162 = ct{1791};
t4164 = ct{1792};
t4165 = ct{1793};
t4169 = ct{1794};
t4170 = ct{1795};
t4171 = ct{1796};
t4173 = ct{1797};
t4174 = ct{1798};
t4177 = ct{1799};
t4178 = ct{1800};
t4179 = ct{1801};
t4182 = ct{1802};
t4184 = ct{1803};
t4186 = ct{1804};
t4187 = ct{1805};
t4188 = ct{1806};
t4189 = ct{1807};
t4190 = ct{1808};
t4191 = ct{1809};
t4192 = ct{1810};
t4193 = ct{1811};
t4194 = ct{1812};
t4195 = ct{1813};
t4196 = ct{1814};
t4197 = ct{1815};
t420 = ct{1816};
t4200 = ct{1817};
t4201 = ct{1818};
t4202 = ct{1819};
t4203 = ct{1820};
t4204 = ct{1821};
t4205 = ct{1822};
t4206 = ct{1823};
t4208 = ct{1824};
t4209 = ct{1825};
t421 = ct{1826};
t4210 = ct{1827};
t4211 = ct{1828};
t4212 = ct{1829};
t4213 = ct{1830};
t4214 = ct{1831};
t4215 = ct{1832};
t4216 = ct{1833};
t4217 = ct{1834};
t4218 = ct{1835};
t4220 = ct{1836};
t4221 = ct{1837};
t4222 = ct{1838};
t4223 = ct{1839};
t4224 = ct{1840};
t4225 = ct{1841};
t4226 = ct{1842};
t4227 = ct{1843};
t4228 = ct{1844};
t4229 = ct{1845};
t4230 = ct{1846};
t4231 = ct{1847};
t4232 = ct{1848};
t4233 = ct{1849};
t4234 = ct{1850};
t4236 = ct{1851};
t4237 = ct{1852};
t4238 = ct{1853};
t4239 = ct{1854};
t4240 = ct{1855};
t4241 = ct{1856};
t4243 = ct{1857};
t4244 = ct{1858};
t4245 = ct{1859};
t4246 = ct{1860};
t4247 = ct{1861};
t4248 = ct{1862};
t4249 = ct{1863};
t425 = ct{1864};
t4250 = ct{1865};
t4252 = ct{1866};
t4253 = ct{1867};
t4255 = ct{1868};
t4256 = ct{1869};
t4258 = ct{1870};
t4259 = ct{1871};
t4260 = ct{1872};
t4261 = ct{1873};
t4262 = ct{1874};
t4263 = ct{1875};
t4265 = ct{1876};
t4266 = ct{1877};
t4268 = ct{1878};
t4269 = ct{1879};
t4271 = ct{1880};
t4272 = ct{1881};
t4273 = ct{1882};
t4274 = ct{1883};
t4276 = ct{1884};
t4277 = ct{1885};
t4278 = ct{1886};
t4280 = ct{1887};
t4281 = ct{1888};
t4282 = ct{1889};
t4285 = ct{1890};
t4286 = ct{1891};
t4290 = ct{1892};
t4295 = ct{1893};
t4296 = ct{1894};
t4298 = ct{1895};
t430 = ct{1896};
t4300 = ct{1897};
t4301 = ct{1898};
t4302 = ct{1899};
t4303 = ct{1900};
t4304 = ct{1901};
t4305 = ct{1902};
t4306 = ct{1903};
t4307 = ct{1904};
t4308 = ct{1905};
t4309 = ct{1906};
t431 = ct{1907};
t4310 = ct{1908};
t4311 = ct{1909};
t4312 = ct{1910};
t4313 = ct{1911};
t4315 = ct{1912};
t4316 = ct{1913};
t4317 = ct{1914};
t4318 = ct{1915};
t4319 = ct{1916};
t4320 = ct{1917};
t4321 = ct{1918};
t4322 = ct{1919};
t4323 = ct{1920};
t4324 = ct{1921};
t4326 = ct{1922};
t4327 = ct{1923};
t4329 = ct{1924};
t433 = ct{1925};
t4330 = ct{1926};
t4332 = ct{1927};
t4333 = ct{1928};
t4334 = ct{1929};
t4337 = ct{1930};
t4339 = ct{1931};
t4340 = ct{1932};
t4341 = ct{1933};
t4342 = ct{1934};
t4343 = ct{1935};
t4344 = ct{1936};
t4345 = ct{1937};
t4346 = ct{1938};
t4347 = ct{1939};
t4348 = ct{1940};
t4349 = ct{1941};
t4350 = ct{1942};
t4351 = ct{1943};
t4352 = ct{1944};
t4354 = ct{1945};
t4355 = ct{1946};
t4356 = ct{1947};
t4357 = ct{1948};
t4358 = ct{1949};
t4359 = ct{1950};
t436 = ct{1951};
t4360 = ct{1952};
t4361 = ct{1953};
t4362 = ct{1954};
t4364 = ct{1955};
t4365 = ct{1956};
t4367 = ct{1957};
t4368 = ct{1958};
t4370 = ct{1959};
t4371 = ct{1960};
t4372 = ct{1961};
t4373 = ct{1962};
t4374 = ct{1963};
t4375 = ct{1964};
t4376 = ct{1965};
t4377 = ct{1966};
t4378 = ct{1967};
t4379 = ct{1968};
t4380 = ct{1969};
t4382 = ct{1970};
t4383 = ct{1971};
t4384 = ct{1972};
t4385 = ct{1973};
t4386 = ct{1974};
t4387 = ct{1975};
t4388 = ct{1976};
t4389 = ct{1977};
t4392 = ct{1978};
t4393 = ct{1979};
t4394 = ct{1980};
t4395 = ct{1981};
t4399 = ct{1982};
t44 = ct{1983};
t4400 = ct{1984};
t4401 = ct{1985};
t4402 = ct{1986};
t4403 = ct{1987};
t4404 = ct{1988};
t4405 = ct{1989};
t4406 = ct{1990};
t4407 = ct{1991};
t4408 = ct{1992};
t4409 = ct{1993};
t4411 = ct{1994};
t4412 = ct{1995};
t4413 = ct{1996};
t4414 = ct{1997};
t4415 = ct{1998};
t4416 = ct{1999};
t4418 = ct{2000};
t4419 = ct{2001};
t4420 = ct{2002};
t4421 = ct{2003};
t4422 = ct{2004};
t4424 = ct{2005};
t4425 = ct{2006};
t4427 = ct{2007};
t4428 = ct{2008};
t4429 = ct{2009};
t4431 = ct{2010};
t4432 = ct{2011};
t4433 = ct{2012};
t4434 = ct{2013};
t4435 = ct{2014};
t4437 = ct{2015};
t4438 = ct{2016};
t4439 = ct{2017};
t4440 = ct{2018};
t4442 = ct{2019};
t4444 = ct{2020};
t4447 = ct{2021};
t4449 = ct{2022};
t445 = ct{2023};
t4450 = ct{2024};
t4451 = ct{2025};
t4452 = ct{2026};
t4453 = ct{2027};
t4454 = ct{2028};
t4455 = ct{2029};
t4457 = ct{2030};
t4458 = ct{2031};
t4459 = ct{2032};
t4460 = ct{2033};
t4461 = ct{2034};
t4462 = ct{2035};
t4465 = ct{2036};
t4467 = ct{2037};
t4469 = ct{2038};
t4470 = ct{2039};
t4471 = ct{2040};
t4472 = ct{2041};
t4473 = ct{2042};
t4475 = ct{2043};
t4476 = ct{2044};
t4477 = ct{2045};
t4478 = ct{2046};
t4479 = ct{2047};
t4480 = ct{2048};
t4481 = ct{2049};
t4482 = ct{2050};
t4483 = ct{2051};
t4484 = ct{2052};
t4485 = ct{2053};
t4486 = ct{2054};
t4487 = ct{2055};
t4488 = ct{2056};
t4489 = ct{2057};
t4490 = ct{2058};
t4492 = ct{2059};
t4493 = ct{2060};
t4495 = ct{2061};
t4496 = ct{2062};
t4497 = ct{2063};
t4498 = ct{2064};
t4499 = ct{2065};
t4500 = ct{2066};
t4501 = ct{2067};
t4502 = ct{2068};
t4503 = ct{2069};
t4504 = ct{2070};
t4505 = ct{2071};
t4506 = ct{2072};
t4507 = ct{2073};
t451 = ct{2074};
t4511 = ct{2075};
t4512 = ct{2076};
t4514 = ct{2077};
t4515 = ct{2078};
t4517 = ct{2079};
t4518 = ct{2080};
t4519 = ct{2081};
t4520 = ct{2082};
t4521 = ct{2083};
t4522 = ct{2084};
t4523 = ct{2085};
t4524 = ct{2086};
t4525 = ct{2087};
t4526 = ct{2088};
t4528 = ct{2089};
t4529 = ct{2090};
t4530 = ct{2091};
t4531 = ct{2092};
t4532 = ct{2093};
t4533 = ct{2094};
t4534 = ct{2095};
t4536 = ct{2096};
t4537 = ct{2097};
t4538 = ct{2098};
t4541 = ct{2099};
t4542 = ct{2100};
t4545 = ct{2101};
t4546 = ct{2102};
t4547 = ct{2103};
t4548 = ct{2104};
t4549 = ct{2105};
t4550 = ct{2106};
t4551 = ct{2107};
t4552 = ct{2108};
t4553 = ct{2109};
t4555 = ct{2110};
t4556 = ct{2111};
t4557 = ct{2112};
t4558 = ct{2113};
t4559 = ct{2114};
t4560 = ct{2115};
t4561 = ct{2116};
t4562 = ct{2117};
t4563 = ct{2118};
t4566 = ct{2119};
t4567 = ct{2120};
t4570 = ct{2121};
t4571 = ct{2122};
t4572 = ct{2123};
t4573 = ct{2124};
t4574 = ct{2125};
t4575 = ct{2126};
t4576 = ct{2127};
t4577 = ct{2128};
t4578 = ct{2129};
t4580 = ct{2130};
t4581 = ct{2131};
t4583 = ct{2132};
t4584 = ct{2133};
t4585 = ct{2134};
t4587 = ct{2135};
t4588 = ct{2136};
t4589 = ct{2137};
t459 = ct{2138};
t4591 = ct{2139};
t4592 = ct{2140};
t4597 = ct{2141};
t4598 = ct{2142};
t4600 = ct{2143};
t4601 = ct{2144};
t4602 = ct{2145};
t4603 = ct{2146};
t4604 = ct{2147};
t4605 = ct{2148};
t4606 = ct{2149};
t4608 = ct{2150};
t4610 = ct{2151};
t4613 = ct{2152};
t4614 = ct{2153};
t4615 = ct{2154};
t4616 = ct{2155};
t4617 = ct{2156};
t4618 = ct{2157};
t4619 = ct{2158};
t4620 = ct{2159};
t4621 = ct{2160};
t4622 = ct{2161};
t4623 = ct{2162};
t4624 = ct{2163};
t4625 = ct{2164};
t4626 = ct{2165};
t4629 = ct{2166};
t4630 = ct{2167};
t4634 = ct{2168};
t4636 = ct{2169};
t4637 = ct{2170};
t4638 = ct{2171};
t4639 = ct{2172};
t4641 = ct{2173};
t4645 = ct{2174};
t4646 = ct{2175};
t4647 = ct{2176};
t4649 = ct{2177};
t465 = ct{2178};
t4651 = ct{2179};
t4652 = ct{2180};
t4653 = ct{2181};
t4655 = ct{2182};
t4657 = ct{2183};
t4659 = ct{2184};
t4660 = ct{2185};
t4661 = ct{2186};
t4662 = ct{2187};
t4663 = ct{2188};
t4664 = ct{2189};
t4665 = ct{2190};
t4666 = ct{2191};
t4667 = ct{2192};
t4668 = ct{2193};
t4669 = ct{2194};
t4672 = ct{2195};
t4673 = ct{2196};
t4674 = ct{2197};
t4675 = ct{2198};
t4678 = ct{2199};
t4681 = ct{2200};
t4682 = ct{2201};
t4683 = ct{2202};
t4684 = ct{2203};
t4685 = ct{2204};
t4686 = ct{2205};
t4687 = ct{2206};
t4695 = ct{2207};
t4697 = ct{2208};
t4698 = ct{2209};
t4700 = ct{2210};
t4701 = ct{2211};
t4702 = ct{2212};
t4704 = ct{2213};
t4705 = ct{2214};
t4706 = ct{2215};
t4707 = ct{2216};
t4708 = ct{2217};
t4709 = ct{2218};
t4710 = ct{2219};
t4711 = ct{2220};
t4712 = ct{2221};
t4713 = ct{2222};
t4720 = ct{2223};
t4722 = ct{2224};
t4723 = ct{2225};
t4724 = ct{2226};
t4729 = ct{2227};
t4732 = ct{2228};
t4733 = ct{2229};
t4735 = ct{2230};
t4736 = ct{2231};
t4737 = ct{2232};
t4738 = ct{2233};
t4742 = ct{2234};
t4746 = ct{2235};
t4747 = ct{2236};
t4749 = ct{2237};
t4750 = ct{2238};
t4751 = ct{2239};
t4752 = ct{2240};
t4753 = ct{2241};
t4754 = ct{2242};
t4755 = ct{2243};
t4756 = ct{2244};
t4758 = ct{2245};
t4759 = ct{2246};
t4761 = ct{2247};
t4764 = ct{2248};
t4766 = ct{2249};
t4769 = ct{2250};
t4770 = ct{2251};
t4771 = ct{2252};
t4772 = ct{2253};
t4773 = ct{2254};
t4775 = ct{2255};
t4776 = ct{2256};
t4780 = ct{2257};
t4781 = ct{2258};
t4783 = ct{2259};
t4784 = ct{2260};
t4785 = ct{2261};
t4786 = ct{2262};
t4787 = ct{2263};
t4788 = ct{2264};
t4789 = ct{2265};
t4790 = ct{2266};
t4796 = ct{2267};
t4799 = ct{2268};
t48 = ct{2269};
t4800 = ct{2270};
t4801 = ct{2271};
t4802 = ct{2272};
t4803 = ct{2273};
t4805 = ct{2274};
t4806 = ct{2275};
t4807 = ct{2276};
t4809 = ct{2277};
t4810 = ct{2278};
t4811 = ct{2279};
t4815 = ct{2280};
t4816 = ct{2281};
t4820 = ct{2282};
t4821 = ct{2283};
t4823 = ct{2284};
t4826 = ct{2285};
t4830 = ct{2286};
t4831 = ct{2287};
t4832 = ct{2288};
t4834 = ct{2289};
t4836 = ct{2290};
t4838 = ct{2291};
t4841 = ct{2292};
t4843 = ct{2293};
t4844 = ct{2294};
t4845 = ct{2295};
t4846 = ct{2296};
t4847 = ct{2297};
t4848 = ct{2298};
t4849 = ct{2299};
t485 = ct{2300};
t4850 = ct{2301};
t4851 = ct{2302};
t4852 = ct{2303};
t4853 = ct{2304};
t4858 = ct{2305};
t4862 = ct{2306};
t4864 = ct{2307};
t4865 = ct{2308};
t4867 = ct{2309};
t4870 = ct{2310};
t4871 = ct{2311};
t4873 = ct{2312};
t4874 = ct{2313};
t4877 = ct{2314};
t4878 = ct{2315};
t4879 = ct{2316};
t488 = ct{2317};
t4880 = ct{2318};
t4881 = ct{2319};
t4882 = ct{2320};
t4883 = ct{2321};
t4884 = ct{2322};
t4888 = ct{2323};
t4889 = ct{2324};
t4890 = ct{2325};
t4892 = ct{2326};
t4895 = ct{2327};
t4897 = ct{2328};
t49 = ct{2329};
t4900 = ct{2330};
t4901 = ct{2331};
t4903 = ct{2332};
t4904 = ct{2333};
t4906 = ct{2334};
t4908 = ct{2335};
t4909 = ct{2336};
t4911 = ct{2337};
t4912 = ct{2338};
t4913 = ct{2339};
t4914 = ct{2340};
t4915 = ct{2341};
t4922 = ct{2342};
t4923 = ct{2343};
t4924 = ct{2344};
t4925 = ct{2345};
t4926 = ct{2346};
t4927 = ct{2347};
t4928 = ct{2348};
t4929 = ct{2349};
t4931 = ct{2350};
t4932 = ct{2351};
t4933 = ct{2352};
t4934 = ct{2353};
t4936 = ct{2354};
t4937 = ct{2355};
t4938 = ct{2356};
t4939 = ct{2357};
t4940 = ct{2358};
t4941 = ct{2359};
t4942 = ct{2360};
t4943 = ct{2361};
t4944 = ct{2362};
t4945 = ct{2363};
t4946 = ct{2364};
t4947 = ct{2365};
t4948 = ct{2366};
t4949 = ct{2367};
t4950 = ct{2368};
t4953 = ct{2369};
t4954 = ct{2370};
t496 = ct{2371};
t4960 = ct{2372};
t4961 = ct{2373};
t4963 = ct{2374};
t4964 = ct{2375};
t4966 = ct{2376};
t4967 = ct{2377};
t4968 = ct{2378};
t4969 = ct{2379};
t4972 = ct{2380};
t4973 = ct{2381};
t4974 = ct{2382};
t4975 = ct{2383};
t4976 = ct{2384};
t4977 = ct{2385};
t4978 = ct{2386};
t4979 = ct{2387};
t4980 = ct{2388};
t4982 = ct{2389};
t4983 = ct{2390};
t4986 = ct{2391};
t4987 = ct{2392};
t4988 = ct{2393};
t4989 = ct{2394};
t4990 = ct{2395};
t4991 = ct{2396};
t4993 = ct{2397};
t4995 = ct{2398};
t4996 = ct{2399};
t4997 = ct{2400};
t4998 = ct{2401};
t4999 = ct{2402};
t5 = ct{2403};
t50 = ct{2404};
t5000 = ct{2405};
t5002 = ct{2406};
t5004 = ct{2407};
t5005 = ct{2408};
t5006 = ct{2409};
t5007 = ct{2410};
t5008 = ct{2411};
t5009 = ct{2412};
t501 = ct{2413};
t5010 = ct{2414};
t5012 = ct{2415};
t5014 = ct{2416};
t5016 = ct{2417};
t5017 = ct{2418};
t5018 = ct{2419};
t5019 = ct{2420};
t502 = ct{2421};
t5021 = ct{2422};
t5022 = ct{2423};
t5023 = ct{2424};
t5024 = ct{2425};
t5026 = ct{2426};
t5027 = ct{2427};
t5030 = ct{2428};
t5031 = ct{2429};
t5032 = ct{2430};
t5033 = ct{2431};
t5036 = ct{2432};
t5038 = ct{2433};
t5039 = ct{2434};
t504 = ct{2435};
t5040 = ct{2436};
t5041 = ct{2437};
t5042 = ct{2438};
t5046 = ct{2439};
t5047 = ct{2440};
t5048 = ct{2441};
t5050 = ct{2442};
t5051 = ct{2443};
t5052 = ct{2444};
t5053 = ct{2445};
t5054 = ct{2446};
t5055 = ct{2447};
t5057 = ct{2448};
t5058 = ct{2449};
t5059 = ct{2450};
t5060 = ct{2451};
t5061 = ct{2452};
t5062 = ct{2453};
t5063 = ct{2454};
t5064 = ct{2455};
t5066 = ct{2456};
t5067 = ct{2457};
t5072 = ct{2458};
t5074 = ct{2459};
t5076 = ct{2460};
t5077 = ct{2461};
t5078 = ct{2462};
t5080 = ct{2463};
t5082 = ct{2464};
t5083 = ct{2465};
t5084 = ct{2466};
t5085 = ct{2467};
t5088 = ct{2468};
t5090 = ct{2469};
t5092 = ct{2470};
t5093 = ct{2471};
t5095 = ct{2472};
t5098 = ct{2473};
t5099 = ct{2474};
t51 = ct{2475};
t5101 = ct{2476};
t5102 = ct{2477};
t5103 = ct{2478};
t5104 = ct{2479};
t5109 = ct{2480};
t5111 = ct{2481};
t5112 = ct{2482};
t5114 = ct{2483};
t5120 = ct{2484};
t5121 = ct{2485};
t5123 = ct{2486};
t5126 = ct{2487};
t5128 = ct{2488};
t5131 = ct{2489};
t5135 = ct{2490};
t5136 = ct{2491};
t5137 = ct{2492};
t5139 = ct{2493};
t5143 = ct{2494};
t5144 = ct{2495};
t5146 = ct{2496};
t5149 = ct{2497};
t5150 = ct{2498};
t5152 = ct{2499};
t5153 = ct{2500};
t5154 = ct{2501};
t5155 = ct{2502};
t5156 = ct{2503};
t5158 = ct{2504};
t5161 = ct{2505};
t5163 = ct{2506};
t5165 = ct{2507};
t5166 = ct{2508};
t5167 = ct{2509};
t5171 = ct{2510};
t5172 = ct{2511};
t5173 = ct{2512};
t5174 = ct{2513};
t5176 = ct{2514};
t5177 = ct{2515};
t5178 = ct{2516};
t5179 = ct{2517};
t5182 = ct{2518};
t5184 = ct{2519};
t5185 = ct{2520};
t519 = ct{2521};
t5190 = ct{2522};
t5191 = ct{2523};
t5193 = ct{2524};
t5194 = ct{2525};
t5197 = ct{2526};
t5198 = ct{2527};
t5199 = ct{2528};
t5202 = ct{2529};
t5203 = ct{2530};
t5204 = ct{2531};
t5205 = ct{2532};
t5206 = ct{2533};
t5207 = ct{2534};
t5208 = ct{2535};
t5214 = ct{2536};
t5215 = ct{2537};
t5217 = ct{2538};
t5218 = ct{2539};
t5220 = ct{2540};
t5223 = ct{2541};
t5224 = ct{2542};
t5225 = ct{2543};
t5227 = ct{2544};
t5229 = ct{2545};
t523 = ct{2546};
t5232 = ct{2547};
t5237 = ct{2548};
t5238 = ct{2549};
t5239 = ct{2550};
t524 = ct{2551};
t5240 = ct{2552};
t5241 = ct{2553};
t5244 = ct{2554};
t5246 = ct{2555};
t5250 = ct{2556};
t5251 = ct{2557};
t5256 = ct{2558};
t5263 = ct{2559};
t5265 = ct{2560};
t5266 = ct{2561};
t5268 = ct{2562};
t527 = ct{2563};
t5271 = ct{2564};
t5272 = ct{2565};
t5274 = ct{2566};
t5275 = ct{2567};
t5280 = ct{2568};
t5285 = ct{2569};
t5286 = ct{2570};
t5287 = ct{2571};
t5288 = ct{2572};
t5289 = ct{2573};
t5290 = ct{2574};
t5291 = ct{2575};
t5293 = ct{2576};
t5294 = ct{2577};
t5299 = ct{2578};
t530 = ct{2579};
t5300 = ct{2580};
t5301 = ct{2581};
t5302 = ct{2582};
t5304 = ct{2583};
t5306 = ct{2584};
t5308 = ct{2585};
t5309 = ct{2586};
t5310 = ct{2587};
t5311 = ct{2588};
t5312 = ct{2589};
t5313 = ct{2590};
t5316 = ct{2591};
t5317 = ct{2592};
t5318 = ct{2593};
t5319 = ct{2594};
t5321 = ct{2595};
t5324 = ct{2596};
t5325 = ct{2597};
t5326 = ct{2598};
t5327 = ct{2599};
t5328 = ct{2600};
t5329 = ct{2601};
t5334 = ct{2602};
t5335 = ct{2603};
t5336 = ct{2604};
t5338 = ct{2605};
t534 = ct{2606};
t5340 = ct{2607};
t5344 = ct{2608};
t5345 = ct{2609};
t5346 = ct{2610};
t5347 = ct{2611};
t5348 = ct{2612};
t5349 = ct{2613};
t5351 = ct{2614};
t5352 = ct{2615};
t5353 = ct{2616};
t5354 = ct{2617};
t5356 = ct{2618};
t5358 = ct{2619};
t5363 = ct{2620};
t5364 = ct{2621};
t5368 = ct{2622};
t5369 = ct{2623};
t537 = ct{2624};
t5370 = ct{2625};
t5372 = ct{2626};
t5374 = ct{2627};
t5378 = ct{2628};
t5379 = ct{2629};
t5380 = ct{2630};
t5382 = ct{2631};
t5384 = ct{2632};
t5385 = ct{2633};
t5386 = ct{2634};
t539 = ct{2635};
t5391 = ct{2636};
t5392 = ct{2637};
t5393 = ct{2638};
t5396 = ct{2639};
t5398 = ct{2640};
t5399 = ct{2641};
t54 = ct{2642};
t5401 = ct{2643};
t5404 = ct{2644};
t5405 = ct{2645};
t5406 = ct{2646};
t5407 = ct{2647};
t5409 = ct{2648};
t541 = ct{2649};
t5412 = ct{2650};
t5413 = ct{2651};
t5417 = ct{2652};
t5419 = ct{2653};
t542 = ct{2654};
t5420 = ct{2655};
t5421 = ct{2656};
t5422 = ct{2657};
t5423 = ct{2658};
t5424 = ct{2659};
t5425 = ct{2660};
t5427 = ct{2661};
t5428 = ct{2662};
t5429 = ct{2663};
t5430 = ct{2664};
t5431 = ct{2665};
t5435 = ct{2666};
t5437 = ct{2667};
t5438 = ct{2668};
t5439 = ct{2669};
t544 = ct{2670};
t5441 = ct{2671};
t5443 = ct{2672};
t5444 = ct{2673};
t5445 = ct{2674};
t5447 = ct{2675};
t5448 = ct{2676};
t5452 = ct{2677};
t5453 = ct{2678};
t5455 = ct{2679};
t5456 = ct{2680};
t5458 = ct{2681};
t5459 = ct{2682};
t546 = ct{2683};
t5460 = ct{2684};
t5461 = ct{2685};
t5463 = ct{2686};
t5464 = ct{2687};
t5470 = ct{2688};
t5474 = ct{2689};
t5475 = ct{2690};
t5476 = ct{2691};
t5477 = ct{2692};
t5480 = ct{2693};
t5481 = ct{2694};
t5484 = ct{2695};
t5486 = ct{2696};
t5488 = ct{2697};
t5490 = ct{2698};
t5492 = ct{2699};
t5493 = ct{2700};
t5494 = ct{2701};
t5498 = ct{2702};
t55 = ct{2703};
t550 = ct{2704};
t5502 = ct{2705};
t5509 = ct{2706};
t5511 = ct{2707};
t5514 = ct{2708};
t5516 = ct{2709};
t5519 = ct{2710};
t5521 = ct{2711};
t5523 = ct{2712};
t5524 = ct{2713};
t5527 = ct{2714};
t5528 = ct{2715};
t553 = ct{2716};
t5530 = ct{2717};
t5533 = ct{2718};
t5536 = ct{2719};
t5538 = ct{2720};
t5539 = ct{2721};
t5540 = ct{2722};
t5542 = ct{2723};
t5543 = ct{2724};
t5546 = ct{2725};
t5547 = ct{2726};
t5548 = ct{2727};
t5550 = ct{2728};
t5551 = ct{2729};
t5552 = ct{2730};
t5553 = ct{2731};
t5556 = ct{2732};
t5557 = ct{2733};
t5563 = ct{2734};
t5565 = ct{2735};
t5566 = ct{2736};
t5569 = ct{2737};
t557 = ct{2738};
t5571 = ct{2739};
t5573 = ct{2740};
t5575 = ct{2741};
t5576 = ct{2742};
t5578 = ct{2743};
t558 = ct{2744};
t5580 = ct{2745};
t5582 = ct{2746};
t5585 = ct{2747};
t5588 = ct{2748};
t5592 = ct{2749};
t5597 = ct{2750};
t5598 = ct{2751};
t5599 = ct{2752};
t56 = ct{2753};
t5601 = ct{2754};
t5602 = ct{2755};
t5603 = ct{2756};
t5606 = ct{2757};
t5607 = ct{2758};
t5616 = ct{2759};
t5618 = ct{2760};
t5619 = ct{2761};
t5620 = ct{2762};
t5622 = ct{2763};
t5623 = ct{2764};
t5627 = ct{2765};
t5629 = ct{2766};
t5631 = ct{2767};
t5632 = ct{2768};
t5633 = ct{2769};
t5638 = ct{2770};
t5642 = ct{2771};
t5644 = ct{2772};
t5648 = ct{2773};
t5657 = ct{2774};
t5658 = ct{2775};
t5659 = ct{2776};
t5660 = ct{2777};
t5661 = ct{2778};
t5662 = ct{2779};
t5663 = ct{2780};
t5664 = ct{2781};
t5667 = ct{2782};
t5668 = ct{2783};
t5670 = ct{2784};
t5672 = ct{2785};
t5674 = ct{2786};
t5677 = ct{2787};
t5678 = ct{2788};
t5682 = ct{2789};
t5684 = ct{2790};
t5685 = ct{2791};
t5686 = ct{2792};
t5687 = ct{2793};
t5688 = ct{2794};
t5689 = ct{2795};
t5690 = ct{2796};
t5691 = ct{2797};
t5692 = ct{2798};
t5693 = ct{2799};
t5694 = ct{2800};
t5696 = ct{2801};
t5697 = ct{2802};
t5699 = ct{2803};
t5704 = ct{2804};
t5705 = ct{2805};
t5706 = ct{2806};
t5707 = ct{2807};
t5709 = ct{2808};
t5710 = ct{2809};
t5712 = ct{2810};
t5713 = ct{2811};
t5715 = ct{2812};
t5717 = ct{2813};
t5721 = ct{2814};
t5722 = ct{2815};
t5724 = ct{2816};
t5726 = ct{2817};
t573 = ct{2818};
t5730 = ct{2819};
t5731 = ct{2820};
t5733 = ct{2821};
t5734 = ct{2822};
t5738 = ct{2823};
t574 = ct{2824};
t5741 = ct{2825};
t5745 = ct{2826};
t5749 = ct{2827};
t575 = ct{2828};
t5754 = ct{2829};
t5756 = ct{2830};
t5761 = ct{2831};
t5763 = ct{2832};
t5771 = ct{2833};
t5772 = ct{2834};
t5776 = ct{2835};
t5778 = ct{2836};
t5779 = ct{2837};
t5780 = ct{2838};
t5781 = ct{2839};
t5785 = ct{2840};
t5786 = ct{2841};
t5788 = ct{2842};
t5789 = ct{2843};
t5791 = ct{2844};
t5792 = ct{2845};
t5793 = ct{2846};
t5795 = ct{2847};
t5798 = ct{2848};
t5800 = ct{2849};
t5805 = ct{2850};
t5808 = ct{2851};
t5809 = ct{2852};
t5814 = ct{2853};
t5815 = ct{2854};
t5818 = ct{2855};
t5820 = ct{2856};
t5823 = ct{2857};
t5824 = ct{2858};
t5826 = ct{2859};
t5829 = ct{2860};
t5832 = ct{2861};
t5835 = ct{2862};
t5837 = ct{2863};
t5840 = ct{2864};
t5841 = ct{2865};
t5843 = ct{2866};
t5845 = ct{2867};
t5846 = ct{2868};
t5847 = ct{2869};
t5848 = ct{2870};
t5855 = ct{2871};
t5857 = ct{2872};
t5859 = ct{2873};
t5862 = ct{2874};
t5867 = ct{2875};
t5868 = ct{2876};
t5869 = ct{2877};
t587 = ct{2878};
t5870 = ct{2879};
t5874 = ct{2880};
t5880 = ct{2881};
t5881 = ct{2882};
t5887 = ct{2883};
t5889 = ct{2884};
t5891 = ct{2885};
t5894 = ct{2886};
t5895 = ct{2887};
t5897 = ct{2888};
t59 = ct{2889};
t5901 = ct{2890};
t5905 = ct{2891};
t5908 = ct{2892};
t5909 = ct{2893};
t5910 = ct{2894};
t5915 = ct{2895};
t5916 = ct{2896};
t5917 = ct{2897};
t5919 = ct{2898};
t5923 = ct{2899};
t5925 = ct{2900};
t5926 = ct{2901};
t5932 = ct{2902};
t5933 = ct{2903};
t5935 = ct{2904};
t5936 = ct{2905};
t5939 = ct{2906};
t5941 = ct{2907};
t5947 = ct{2908};
t5949 = ct{2909};
t595 = ct{2910};
t5959 = ct{2911};
t5960 = ct{2912};
t5963 = ct{2913};
t5964 = ct{2914};
t5967 = ct{2915};
t5970 = ct{2916};
t5971 = ct{2917};
t5973 = ct{2918};
t5980 = ct{2919};
t5981 = ct{2920};
t5982 = ct{2921};
t5983 = ct{2922};
t5984 = ct{2923};
t5985 = ct{2924};
t5986 = ct{2925};
t5988 = ct{2926};
t5989 = ct{2927};
t5990 = ct{2928};
t5991 = ct{2929};
t5992 = ct{2930};
t5996 = ct{2931};
t5998 = ct{2932};
t6000 = ct{2933};
t6001 = ct{2934};
t6009 = ct{2935};
t6010 = ct{2936};
t6013 = ct{2937};
t6014 = ct{2938};
t6015 = ct{2939};
t6021 = ct{2940};
t6024 = ct{2941};
t603 = ct{2942};
t6049 = ct{2943};
t6051 = ct{2944};
t6052 = ct{2945};
t6066 = ct{2946};
t6067 = ct{2947};
t6074 = ct{2948};
t6083 = ct{2949};
t6099 = ct{2950};
t61 = ct{2951};
t6117 = ct{2952};
t6129 = ct{2953};
t614 = ct{2954};
t628 = ct{2955};
t629 = ct{2956};
t634 = ct{2957};
t641 = ct{2958};
t65 = ct{2959};
t650 = ct{2960};
t651 = ct{2961};
t655 = ct{2962};
t6555 = ct{2963};
t6557 = ct{2964};
t657 = ct{2965};
t6599 = ct{2966};
t6628 = ct{2967};
t6629 = ct{2968};
t664 = ct{2969};
t665 = ct{2970};
t666 = ct{2971};
t667 = ct{2972};
t668 = ct{2973};
t669 = ct{2974};
t675 = ct{2975};
t68 = ct{2976};
t693 = ct{2977};
t7 = ct{2978};
t71 = ct{2979};
t721 = ct{2980};
t724 = ct{2981};
t73 = ct{2982};
t731 = ct{2983};
t732 = ct{2984};
t736 = ct{2985};
t741 = ct{2986};
t753 = ct{2987};
t754 = ct{2988};
t755 = ct{2989};
t756 = ct{2990};
t757 = ct{2991};
t759 = ct{2992};
t760 = ct{2993};
t761 = ct{2994};
t762 = ct{2995};
t765 = ct{2996};
t769 = ct{2997};
t772 = ct{2998};
t774 = ct{2999};
t776 = ct{3000};
t778 = ct{3001};
t795 = ct{3002};
t797 = ct{3003};
t799 = ct{3004};
t8 = ct{3005};
t802 = ct{3006};
t803 = ct{3007};
t806 = ct{3008};
t817 = ct{3009};
t818 = ct{3010};
t820 = ct{3011};
t828 = ct{3012};
t831 = ct{3013};
t838 = ct{3014};
t843 = ct{3015};
t846 = ct{3016};
t847 = ct{3017};
t848 = ct{3018};
t850 = ct{3019};
t851 = ct{3020};
t852 = ct{3021};
t853 = ct{3022};
t855 = ct{3023};
t865 = ct{3024};
t867 = ct{3025};
t868 = ct{3026};
t870 = ct{3027};
t871 = ct{3028};
t872 = ct{3029};
t876 = ct{3030};
t886 = ct{3031};
t888 = ct{3032};
t9 = ct{3033};
t901 = ct{3034};
t902 = ct{3035};
t903 = ct{3036};
t904 = ct{3037};
t906 = ct{3038};
t907 = ct{3039};
t909 = ct{3040};
t914 = ct{3041};
t925 = ct{3042};
t926 = ct{3043};
t947 = ct{3044};
t949 = ct{3045};
t952 = ct{3046};
t955 = ct{3047};
t957 = ct{3048};
t964 = ct{3049};
t972 = ct{3050};
t977 = ct{3051};
t983 = ct{3052};
t991 = ct{3053};
t992 = ct{3054};
t993 = ct{3055};
t994 = ct{3056};
t995 = ct{3057};
t6026 = t4408.*t5566;
t6029 = t4392.*t5607;
t6030 = t4447.*t5556;
t6036 = -t4447.*(t2215-t2237+t3424+t3427-t3439+t8.*t872.*(t534-t546).*9.52624335e-4);
t6038 = -t4392.*(-t2503+t2754+t3433-t3460+t3506+t4.*t871.*(t534-t546).*9.52624335e-4);
t6039 = t4447.*t5607;
t6042 = t4392.*(-t2503+t2754+t3433-t3460+t3506+t4.*t871.*(t534-t546).*9.52624335e-4);
t6045 = t4476.*t5566;
t6056 = t4392.*(t2706-t2712+t3512+t3528+t3534+t3552);
t6057 = t4476.*t5607;
t6058 = t4392.*(t2883+t2956-t3186-t3199+t3602+t3661);
t6069 = -t6067;
t6075 = t4447.*(t2706-t2712+t3512+t3528+t3534+t3552);
t6086 = -t6083;
t6089 = t1663+t2349+t2408+t3007+t3019+t3500+t3558+t3622+t3623;
t6090 = t1563+t2408+t2534+t2865+t2874+t3558+t3579+t3622+t3747;
t6091 = t1563+t2349+t2619+t2865+t2874+t3500+t3623+t3673+t3741;
t6098 = -t3967.*(t2449.*3.372786875e-3+t3544+t3545+t3598-t3934-t3966);
t6101 = t3967.*(t2449.*3.372786875e-3+t3544+t3545+t3598-t3934-t3966);
t6104 = t2321+t2385+t2749+t3011+t3041+t3223+t3251+t3542+t3616;
t6105 = t2252+t2480+t2749+t2870+t2897+t3377+t3384+t3542+t3616;
t6106 = t2252+t2321+t2870+t2886+t2897+t3223+t3251+t3637+t3767;
t6111 = t2211+t2321+t2781+t2995+t3033+t3223+t3251+t3654+t3674;
t6123 = -t4164.*(t2449.*3.372786875e-3+t3544+t3545+t3598-t3934-t3966);
t6125 = t2211+t2321+t2959+t2995+t3033+t3223+t3251+t3799+t3806;
t6128 = t4164.*(t2449.*3.372786875e-3+t3544+t3545+t3598-t3934-t3966);
t6135 = -t4237.*(t2449.*3.372786875e-3+t3544+t3545+t3598-t3934-t3966);
t6138 = t2350+t2462+t2781+t3134+t3158+t3349+t3368+t3654+t3674;
t6140 = t4237.*(t2449.*3.372786875e-3+t3544+t3545+t3598-t3934-t3966);
t6141 = -t4255.*(t2449.*3.36554e-3+t3490+t3648+t3649-t3934-t3966);
t6143 = t4255.*(t2449.*3.36554e-3+t3490+t3648+t3649-t3934-t3966);
t6148 = -t4311.*(t2449.*3.36554e-3+t3490+t3648+t3649-t3934-t3966);
t6150 = t4311.*(t2449.*3.36554e-3+t3490+t3648+t3649-t3934-t3966);
t6158 = (t1260-t2364+t1430.*(t105-t465)).*(t2449.*3.372786875e-3+t3544+t3545+t3598-t3934-t3966);
t6161 = -t4382.*(t2449.*3.36554e-3+t3490+t3648+t3649-t3934-t3966);
t6164 = (t1396-t2573+t1430.*(t197-t537).*2.0).*(t2449.*3.36554e-3+t3490+t3544+t3545-t4001-t4034);
t6165 = -t4454.*(t2449.*3.372786875e-3+t3544+t3545+t3598-t3934-t3966);
t6166 = t4454.*(t2449.*3.372786875e-3+t3544+t3545+t3598-t3934-t3966);
t6171 = -t4471.*(t2449.*3.36554e-3+t3490+t3544+t3545-t4001-t4034);
t6174 = (-t1018+t1426+t1431-t1446+t3.*t496.*(t105-t465)).*(t2449.*3.372786875e-3+t3544+t3545+t3598-t3934-t3966);
t6176 = (t1395-t2868+t1505.*(t534-t546).*2.0).*(t2449.*3.36554e-3+t3490+t3544+t3545-t4001-t4034);
t6182 = -t4581.*(t2449.*3.372786875e-3+t3544+t3545+t3598-t3934-t3966);
t6183 = (t1019-t1651+t1702+t3.*t818.*(t105-t465)+t3.*t872.*(t103-t544)).*(t2449.*3.372786875e-3+t3544+t3545+t3598-t3934-t3966);
t6187 = -t4672.*(t2449.*3.372786875e-3+t3544+t3545+t3598-t3934-t3966);
t6191 = t4672.*(t2449.*3.372786875e-3+t3544+t3545+t3598-t3934-t3966);
t6192 = -t3967.*(t1970-t1971+t2487+t3161-t3236-t3794-t3817+t1240.*(t105-t465).*3.372786875e-3+t903.*(t534-t546).*3.372786875e-3);
t6193 = -t4686.*(t2449.*3.372786875e-3+t3544+t3545+t3598-t3934-t3966);
t6195 = t3967.*(t1970-t1971+t2487+t3161-t3236-t3794-t3817+t1240.*(t105-t465).*3.372786875e-3+t903.*(t534-t546).*3.372786875e-3);
t6196 = t4686.*(t2449.*3.372786875e-3+t3544+t3545+t3598-t3934-t3966);
t6197 = t4162.*t6099;
t6198 = (t995+t1064-t1506+t1598-t1763-t1774).*(t2449.*3.36554e-3+t3490+t3648+t3649-t3934-t3966);
t6199 = t3961.*t6129;
t6200 = -t4695.*(t2449.*3.372786875e-3+t3544+t3545+t3598-t3934-t3966);
t6204 = t4695.*(t2449.*3.372786875e-3+t3544+t3545+t3598-t3934-t3966);
t6205 = (t2449.*3.36554e-3+t3490+t3648+t3649-t3934-t3966).*(t820+t1121-t1435+t1997+t2000+t11.*t420.*(t214-t541));
t6211 = (t2449.*3.372786875e-3+t3544+t3545+t3598-t3934-t3966).*(t1260-t1328-t1427-t1441+t1706+t9.*t870.*(t105-t465));
t6219 = t4277.*t6099;
t6221 = (t753+t991-t1771-t1957+t1181.*(t105-t465)+t11.*t381.*(t534-t546)).*(t2449.*3.372786875e-3+t3544+t3545+t3598-t3934-t3966);
t6222 = (t1064+t1137-t1694+t1698-t1763-t1774).*(t2449.*3.36554e-3+t3490+t3648+t3649-t3934-t3966);
t6225 = -t4173.*(-t1865+t2158+t2487+t3302-t3390-t3794-t3817+t1240.*(t105-t465).*3.36554e-3+t903.*(t534-t546).*3.36554e-3);
t6226 = -t4162.*(t1970-t1971+t2487+t3161-t3236-t3794-t3817+t1240.*(t105-t465).*3.372786875e-3+t903.*(t534-t546).*3.372786875e-3);
t6227 = -t4164.*(t1970-t1971+t2487+t3161-t3236-t3794-t3817+t1240.*(t105-t465).*3.372786875e-3+t903.*(t534-t546).*3.372786875e-3);
t6229 = t4162.*(t1970-t1971+t2487+t3161-t3236-t3794-t3817+t1240.*(t105-t465).*3.372786875e-3+t903.*(t534-t546).*3.372786875e-3);
t6230 = t4164.*(t1970-t1971+t2487+t3161-t3236-t3794-t3817+t1240.*(t105-t465).*3.372786875e-3+t903.*(t534-t546).*3.372786875e-3);
t6231 = (t867+t1059-t1646-t1705+t1938-t2002).*(t2449.*3.36554e-3+t3490+t3648+t3649-t3934-t3966);
t6234 = t4313.*t6099;
t6236 = t4173.*t6129;
t6240 = -t6129.*(-t1262+t1701+t9.*t868.*(t105-t465));
t6241 = -t4738.*(t2449.*3.36554e-3+t3490+t3648+t3649-t3934-t3966);
t6249 = -t6129.*(-t947+t1240.*(t105-t465)+t903.*(t534-t546));
t6253 = -t4770.*(t2449.*3.36554e-3+t3490+t3648+t3649-t3934-t3966);
t6256 = -t4311.*(-t1865+t2158+t2487+t3302-t3390-t3794-t3817+t1240.*(t105-t465).*3.36554e-3+t903.*(t534-t546).*3.36554e-3);
t6258 = -t6099.*(-t1331+t2317+t1510.*(t103-t544));
t6261 = t4311.*(-t1865+t2158+t2487+t3302-t3390-t3794-t3817+t1240.*(t105-t465).*3.36554e-3+t903.*(t534-t546).*3.36554e-3);
t6263 = -(t1079+t1956-t4277-t1178.*(t105-t465)).*(t2449.*3.372786875e-3+t3544+t3545+t3598-t3934-t3966);
t6264 = (t1079+t1956-t4277-t1178.*(t105-t465)).*(t2449.*3.372786875e-3+t3544+t3545+t3598-t3934-t3966);
t6268 = (t2449.*3.36554e-3+t3490+t3648+t3649-t3934-t3966).*(t1060+t1138-t1883+t1932+t2088+t1179.*(t103-t544));
t6273 = (t1185+t1813-t4313+t1047.*(t105-t465)).*(t2449.*3.372786875e-3+t3544+t3545+t3598-t3934-t3966);
t6274 = t4392.*t6117;
t6275 = (t1250-t1261+t1761-t2083-t2111+t1037.*(t103-t544)).*(t2449.*3.36554e-3+t3490+t3648+t3649-t3934-t3966);
t6277 = (t1260-t2364+t1430.*(t105-t465)).*(t1970-t1971+t2487+t3161-t3236-t3794-t3817+t1240.*(t105-t465).*3.372786875e-3+t903.*(t534-t546).*3.372786875e-3);
t6278 = -t4382.*(-t1865+t2158+t2487+t3302-t3390-t3794-t3817+t1240.*(t105-t465).*3.36554e-3+t903.*(t534-t546).*3.36554e-3);
t6281 = -t4821.*(t2449.*3.36554e-3+t3490+t3544+t3545-t4001-t4034);
t6282 = (t1053+t1332+t2368+t817.*(t214-t541)+t977.*(t103-t544)+t1512.*(t105-t465)).*(t2449.*3.36554e-3+t3490+t3648+t3649-t3934-t3966);
t6284 = t4408.*t6117;
t6287 = -t4823.*(t2449.*3.36554e-3+t3490+t3544+t3545-t4001-t4034);
t6290 = t4823.*(t2449.*3.36554e-3+t3490+t3544+t3545-t4001-t4034);
t6292 = (t2449.*3.36554e-3+t3490+t3544+t3545-t4001-t4034).*(-t1129+t1139-t2082+t2110+t2123+t8.*t872.*(t534-t546));
t6295 = -t4834.*(t2449.*3.36554e-3+t3490+t3544+t3545-t4001-t4034);
t6296 = t4447.*t6117;
t6303 = -t4849.*(t2449.*3.36554e-3+t3490+t3544+t3545-t4001-t4034);
t6304 = (t1396-t2573+t1430.*(t197-t537).*2.0).*(-t1865+t1970+t2708+t3161-t3236-t3845-t3870+t1240.*(t105-t465).*3.36554e-3+t903.*(t534-t546).*3.36554e-3);
t6309 = -t4454.*(t1970-t1971+t2487+t3161-t3236-t3794-t3817+t1240.*(t105-t465).*3.372786875e-3+t903.*(t534-t546).*3.372786875e-3);
t6311 = t4476.*t6117;
t6313 = -t4897.*(t2449.*3.36554e-3+t3490+t3544+t3545-t4001-t4034);
t6314 = -t4471.*(-t1865+t1970+t2708+t3161-t3236-t3845-t3870+t1240.*(t105-t465).*3.36554e-3+t903.*(t534-t546).*3.36554e-3);
t6315 = t4897.*(t2449.*3.36554e-3+t3490+t3544+t3545-t4001-t4034);
t6316 = t4471.*(-t1865+t1970+t2708+t3161-t3236-t3845-t3870+t1240.*(t105-t465).*3.36554e-3+t903.*(t534-t546).*3.36554e-3);
t6317 = (-t1018+t1426+t1431-t1446+t3.*t496.*(t105-t465)).*(t1970-t1971+t2487+t3161-t3236-t3794-t3817+t1240.*(t105-t465).*3.372786875e-3+t903.*(t534-t546).*3.372786875e-3);
t6320 = (t1395-t2868+t1505.*(t534-t546).*2.0).*(-t1865+t1970+t2708+t3161-t3236-t3845-t3870+t1240.*(t105-t465).*3.36554e-3+t903.*(t534-t546).*3.36554e-3);
t6329 = -t4922.*(t2449.*3.36554e-3+t3490+t3544+t3545-t4001-t4034);
t6330 = -t4923.*(t2449.*3.36554e-3+t3490+t3544+t3545-t4001-t4034);
t6332 = t4922.*(t2449.*3.36554e-3+t3490+t3544+t3545-t4001-t4034);
t6345 = -t4575.*(t1970-t1971+t2487+t3161-t3236-t3794-t3817+t1240.*(t105-t465).*3.372786875e-3+t903.*(t534-t546).*3.372786875e-3);
t6347 = -t4581.*(t1970-t1971+t2487+t3161-t3236-t3794-t3817+t1240.*(t105-t465).*3.372786875e-3+t903.*(t534-t546).*3.372786875e-3);
t6351 = t4581.*(t1970-t1971+t2487+t3161-t3236-t3794-t3817+t1240.*(t105-t465).*3.372786875e-3+t903.*(t534-t546).*3.372786875e-3);
t6352 = -t4592.*(-t1865+t2158+t2487+t3302-t3390-t3794-t3817+t1240.*(t105-t465).*3.36554e-3+t903.*(t534-t546).*3.36554e-3);
t6354 = (t1019-t1651+t1702+t3.*t818.*(t105-t465)+t3.*t872.*(t103-t544)).*(t1970-t1971+t2487+t3161-t3236-t3794-t3817+t1240.*(t105-t465).*3.372786875e-3+t903.*(t534-t546).*3.372786875e-3);
t6356 = t4592.*(-t1865+t2158+t2487+t3302-t3390-t3794-t3817+t1240.*(t105-t465).*3.36554e-3+t903.*(t534-t546).*3.36554e-3);
t6361 = -t4618.*(-t1865+t2158+t2487+t3302-t3390-t3794-t3817+t1240.*(t105-t465).*3.36554e-3+t903.*(t534-t546).*3.36554e-3);
t6365 = -t4638.*(t1970-t1971+t2487+t3161-t3236-t3794-t3817+t1240.*(t105-t465).*3.372786875e-3+t903.*(t534-t546).*3.372786875e-3);
t6369 = (t2449.*3.36554e-3+t3490+t3544+t3545-t4001-t4034).*(t1176-t1366+t2434+t2435-t2899+t1430.*(t539+t641));
t6370 = -t4645.*(-t1865+t2158+t2487+t3302-t3390-t3794-t3817+t1240.*(t105-t465).*3.36554e-3+t903.*(t534-t546).*3.36554e-3);
t6372 = (t1751+t2308+t964.*(t105-t465)+t1430.*(t103-t544)).*(t1970-t1971+t2487+t3161-t3236-t3794-t3817+t1240.*(t105-t465).*3.372786875e-3+t903.*(t534-t546).*3.372786875e-3);
t6376 = t1667+t2382+t2438+t2447+t3012+t3022+t3458+t3543+t3587+t3594+t3600+t3621;
t6377 = t1568+t2438+t2447+t2528+t2871+t2875+t3543+t3550+t3587+t3594+t3600+t3746;
t6384 = t1568+t2382+t2657+t2663+t2871+t2875+t3458+t3621+t3638+t3697+t3735+t3745;
t6385 = -t4695.*(t1970-t1971+t2487+t3161-t3236-t3794-t3817+t1240.*(t105-t465).*3.372786875e-3+t903.*(t534-t546).*3.372786875e-3);
t6388 = t2324+t2346+t2786+t2838+t3006+t3047+t3185+t3250+t3536+t3591+t3596+t3615;
t6389 = t2172+t2474+t2786+t2838+t2864+t2909+t3334+t3375+t3536+t3591+t3596+t3615;
t6391 = (t1260-t1328-t1427-t1441+t1706+t9.*t870.*(t105-t465)).*(t1970-t1971+t2487+t3161-t3236-t3794-t3817+t1240.*(t105-t465).*3.372786875e-3+t903.*(t534-t546).*3.372786875e-3);
t6393 = (t1365-t1443+t2829-t2831-t2833+t1505.*(t534-t546)).*(t2449.*3.36554e-3+t3490+t3544+t3545-t4001-t4034);
t6399 = t2172+t2346+t2864+t2909+t2916+t2979+t3185+t3250+t3630+t3693+t3700+t3765;
t6400 = (t1064+t1137-t1694+t1698-t1763-t1774).*(-t1865+t2158+t2487+t3302-t3390-t3794-t3817+t1240.*(t105-t465).*3.36554e-3+t903.*(t534-t546).*3.36554e-3);
t6405 = -t4738.*(-t1865+t2158+t2487+t3302-t3390-t3794-t3817+t1240.*(t105-t465).*3.36554e-3+t903.*(t534-t546).*3.36554e-3);
t6406 = t4738.*(-t1865+t2158+t2487+t3302-t3390-t3794-t3817+t1240.*(t105-t465).*3.36554e-3+t903.*(t534-t546).*3.36554e-3);
t6409 = t1966+t2046+t2400+t2545+t3156+t3162+t3277+t3284+t3818+t3831+t3833+t3854;
t6410 = t1909+t2157+t2400+t2545+t3146+t3151+t3300+t3303+t3818+t3831+t3833+t3854;
t6413 = (t2436-t2536+t1510.*(t197-t537)+t1505.*(t214-t541)).*(-t1865+t1970+t2708+t3161-t3236-t3845-t3870+t1240.*(t105-t465).*3.36554e-3+t903.*(t534-t546).*3.36554e-3);
t6419 = -t4770.*(-t1865+t2158+t2487+t3302-t3390-t3794-t3817+t1240.*(t105-t465).*3.36554e-3+t903.*(t534-t546).*3.36554e-3);
t6421 = t4770.*(-t1865+t2158+t2487+t3302-t3390-t3794-t3817+t1240.*(t105-t465).*3.36554e-3+t903.*(t534-t546).*3.36554e-3);
t6422 = t1909+t1966+t2598+t2756+t3146+t3151+t3156+t3162+t3872+t3888+t3890+t3919;
t6430 = -(t1079+t1956-t4277-t1178.*(t105-t465)).*(t1970-t1971+t2487+t3161-t3236-t3794-t3817+t1240.*(t105-t465).*3.372786875e-3+t903.*(t534-t546).*3.372786875e-3);
t6433 = (t1060+t1138-t1883+t1932+t2088+t1179.*(t103-t544)).*(-t1865+t2158+t2487+t3302-t3390-t3794-t3817+t1240.*(t105-t465).*3.36554e-3+t903.*(t534-t546).*3.36554e-3);
t6434 = (t1185+t1813-t4313+t1047.*(t105-t465)).*(t1970-t1971+t2487+t3161-t3236-t3794-t3817+t1240.*(t105-t465).*3.372786875e-3+t903.*(t534-t546).*3.372786875e-3);
t6439 = (t1250-t1261+t1761-t2083-t2111+t1037.*(t103-t544)).*(-t1865+t2158+t2487+t3302-t3390-t3794-t3817+t1240.*(t105-t465).*3.36554e-3+t903.*(t534-t546).*3.36554e-3);
t6443 = (t1053+t1332+t2368+t817.*(t214-t541)+t977.*(t103-t544)+t1512.*(t105-t465)).*(-t1865+t2158+t2487+t3302-t3390-t3794-t3817+t1240.*(t105-t465).*3.36554e-3+t903.*(t534-t546).*3.36554e-3);
t6446 = -t4823.*(-t1865+t1970+t2708+t3161-t3236-t3845-t3870+t1240.*(t105-t465).*3.36554e-3+t903.*(t534-t546).*3.36554e-3);
t6447 = -t4830.*(-t1865+t1970+t2708+t3161-t3236-t3845-t3870+t1240.*(t105-t465).*3.36554e-3+t903.*(t534-t546).*3.36554e-3);
t6448 = (-t1129+t1139-t2082+t2110+t2123+t8.*t872.*(t534-t546)).*(-t1865+t1970+t2708+t3161-t3236-t3845-t3870+t1240.*(t105-t465).*3.36554e-3+t903.*(t534-t546).*3.36554e-3);
t6449 = -t4834.*(-t1865+t1970+t2708+t3161-t3236-t3845-t3870+t1240.*(t105-t465).*3.36554e-3+t903.*(t534-t546).*3.36554e-3);
t6450 = -t4849.*(-t1865+t1970+t2708+t3161-t3236-t3845-t3870+t1240.*(t105-t465).*3.36554e-3+t903.*(t534-t546).*3.36554e-3);
t6455 = -t4897.*(-t1865+t1970+t2708+t3161-t3236-t3845-t3870+t1240.*(t105-t465).*3.36554e-3+t903.*(t534-t546).*3.36554e-3);
t6459 = -t4923.*(-t1865+t1970+t2708+t3161-t3236-t3845-t3870+t1240.*(t105-t465).*3.36554e-3+t903.*(t534-t546).*3.36554e-3);
t6460 = t4923.*(-t1865+t1970+t2708+t3161-t3236-t3845-t3870+t1240.*(t105-t465).*3.36554e-3+t903.*(t534-t546).*3.36554e-3);
t6466 = t2919+t2964+t3083+t3108+t3508+t3539+t3578+t3613+t3652+t3653+t3655+t3708;
t6467 = t2926+t2966+t3061+t3100+t3494+t3595+t3613+t3624+t3652+t3653+t3655+t3666;
t6468 = t2919+t2926+t2964+t2966+t3494+t3508+t3539+t3595+t3762+t3784+t3785+t3789;
t6471 = t3938.*(t1568-t2347+t2657+t2663+t2871+t2875+t3458+t3621+t3638+t3697+t3735+t3745);
t6482 = t4162.*(t1568-t2404-t2412+t2528+t2871+t2875+t3543+t3550+t3587+t3594+t3600+t3746);
t6483 = t4173.*(t1667-t2347+t2438+t2447+t3012+t3022+t3458+t3543+t3587+t3594+t3600+t3621);
t6484 = -(-t1262+t1701+t9.*t868.*(t105-t465)).*(t1667-t2347+t2438+t2447+t3012+t3022+t3458+t3543+t3587+t3594+t3600+t3621);
t6485 = t3097+t3218+t3254+t3258+t3296+t3306+t3332+t3386+t3795+t3829+t3840+t3842;
t6486 = t3145+t3166+t3184+t3231+t3239+t3360+t3405+t3409+t3795+t3829+t3840+t3842;
t6487 = t3097+t3145+t3166+t3184+t3218+t3231+t3254+t3258+t3846+t3886+t3911+t3913;
t6492 = t761+t1403+t1480+t1590+t2570+t3399+t3404+t4177+t4178+t5424;
t6493 = -(-t947+t1240.*(t105-t465)+t903.*(t534-t546)).*(t1667-t2347+t2438+t2447+t3012+t3022+t3458+t3543+t3587+t3594+t3600+t3621);
t6495 = (-t947+t1240.*(t105-t465)+t903.*(t534-t546)).*(t1667-t2347+t2438+t2447+t3012+t3022+t3458+t3543+t3587+t3594+t3600+t3621);
t6497 = t4277.*(t1568-t2404-t2412+t2528+t2871+t2875+t3543+t3550+t3587+t3594+t3600+t3746);
t6501 = t4313.*(t1568-t2404-t2412+t2528+t2871+t2875+t3543+t3550+t3587+t3594+t3600+t3746);
t6506 = -(t1332+t2368+t1512.*(t105-t465)).*(t1667-t2347+t2438+t2447+t3012+t3022+t3458+t3543+t3587+t3594+t3600+t3621);
t6510 = t4392.*(t1568-t2347+t2657+t2663+t2871+t2875+t3458+t3621+t3638+t3697+t3735+t3745);
t6526 = t4447.*(t1568-t2347+t2657+t2663+t2871+t2875+t3458+t3621+t3638+t3697+t3735+t3745);
t6531 = t4476.*(t1568-t2347+t2657+t2663+t2871+t2875+t3458+t3621+t3638+t3697+t3735+t3745);
t6538 = t756+t759+t1187+t1192+t1463+t1546+t1585+t1595+t2216+t2230+t2764+t2774+t3469+t3488+t3491+t3581+t4191+t4192;
t6539 = t760+t762+t1188+t1191+t1469+t1551+t1587+t1599+t2217+t2229+t2766+t2776+t3484+t3492+t3497+t3565+t4193+t4194;
et1 = t2920+t2927+t3489-t3494+t3722-t3784+t964.*(t105-t465).*3.36554e-3+t977.*(t105-t465).*3.36554e-3+t1430.*(t103-t544).*3.36554e-3+t1512.*(t103-t544).*3.36554e-3;
et2 = t1510.*(t197-t537).*3.372816795e-3+t1505.*(t214-t541).*3.372816795e-3;
t6549 = -t3938.*(et1+et2);
et3 = t2927+t3062-t3494+t3584+t3597-t3652+t964.*(t105-t465).*3.372786875e-3+t977.*(t105-t465).*3.36554e-3+t1430.*(t103-t544).*3.372786875e-3+t1512.*(t103-t544).*3.36554e-3;
et4 = t1510.*(t197-t537).*3.36554e-3+t1505.*(t214-t541).*3.36554e-3;
t6550 = -t3961.*(et3+et4);
et5 = t2927+t3062-t3494+t3584+t3597-t3652+t964.*(t105-t465).*3.372786875e-3+t977.*(t105-t465).*3.36554e-3+t1430.*(t103-t544).*3.372786875e-3+t1512.*(t103-t544).*3.36554e-3;
et6 = t1510.*(t197-t537).*3.36554e-3+t1505.*(t214-t541).*3.36554e-3;
t6552 = t3961.*(et5+et6);
et7 = t2927+t3062-t3494+t3584+t3597-t3652+t964.*(t105-t465).*3.372786875e-3+t977.*(t105-t465).*3.36554e-3+t1430.*(t103-t544).*3.372786875e-3+t1512.*(t103-t544).*3.36554e-3;
et8 = t1510.*(t197-t537).*3.36554e-3+t1505.*(t214-t541).*3.36554e-3;
t6562 = (et7+et8).*(-t1262+t1701+t9.*t868.*(t105-t465));
et9 = t2927+t3062-t3494+t3584+t3597-t3652+t964.*(t105-t465).*3.372786875e-3+t977.*(t105-t465).*3.36554e-3+t1430.*(t103-t544).*3.372786875e-3+t1512.*(t103-t544).*3.36554e-3;
et10 = t1510.*(t197-t537).*3.36554e-3+t1505.*(t214-t541).*3.36554e-3;
t6565 = (et9+et10).*(-t947+t1240.*(t105-t465)+t903.*(t534-t546));
et11 = t2920+t3084+t3489-t3578+t3584-t3652+t964.*(t105-t465).*3.36554e-3+t977.*(t105-t465).*3.367829185e-3+t1430.*(t103-t544).*3.36554e-3+t1512.*(t103-t544).*3.367829185e-3;
et12 = t1510.*(t197-t537).*3.36554e-3+t1505.*(t214-t541).*3.36554e-3;
t6566 = -t4277.*(et11+et12);
et13 = t2920+t3084+t3489-t3578+t3584-t3652+t964.*(t105-t465).*3.36554e-3+t977.*(t105-t465).*3.367829185e-3+t1430.*(t103-t544).*3.36554e-3+t1512.*(t103-t544).*3.367829185e-3;
et14 = t1510.*(t197-t537).*3.36554e-3+t1505.*(t214-t541).*3.36554e-3;
t6567 = t4277.*(et13+et14);
et15 = t2920+t3084+t3489-t3578+t3584-t3652+t964.*(t105-t465).*3.36554e-3+t977.*(t105-t465).*3.367829185e-3+t1430.*(t103-t544).*3.36554e-3+t1512.*(t103-t544).*3.367829185e-3;
et16 = t1510.*(t197-t537).*3.36554e-3+t1505.*(t214-t541).*3.36554e-3;
t6571 = -t4313.*(et15+et16);
et17 = t2927+t3062-t3494+t3584+t3597-t3652+t964.*(t105-t465).*3.372786875e-3+t977.*(t105-t465).*3.36554e-3+t1430.*(t103-t544).*3.372786875e-3+t1512.*(t103-t544).*3.36554e-3;
et18 = t1510.*(t197-t537).*3.36554e-3+t1505.*(t214-t541).*3.36554e-3;
t6580 = (et17+et18).*(t1332+t2368+t1512.*(t105-t465));
et19 = t2920+t3084+t3489-t3578+t3584-t3652+t964.*(t105-t465).*3.36554e-3+t977.*(t105-t465).*3.367829185e-3+t1430.*(t103-t544).*3.36554e-3+t1512.*(t103-t544).*3.367829185e-3;
et20 = t1510.*(t197-t537).*3.36554e-3+t1505.*(t214-t541).*3.36554e-3;
t6581 = (et19+et20).*(-t1331+t2317+t1510.*(t103-t544));
et21 = t2920+t2927+t3489-t3494+t3722-t3784+t964.*(t105-t465).*3.36554e-3+t977.*(t105-t465).*3.36554e-3+t1430.*(t103-t544).*3.36554e-3+t1512.*(t103-t544).*3.36554e-3;
et22 = t1510.*(t197-t537).*3.372816795e-3+t1505.*(t214-t541).*3.372816795e-3;
t6584 = -t4408.*(et21+et22);
et23 = t2920+t2927+t3489-t3494+t3722-t3784+t964.*(t105-t465).*3.36554e-3+t977.*(t105-t465).*3.36554e-3+t1430.*(t103-t544).*3.36554e-3+t1512.*(t103-t544).*3.36554e-3;
et24 = t1510.*(t197-t537).*3.372816795e-3+t1505.*(t214-t541).*3.372816795e-3;
t6588 = -t4447.*(et23+et24);
et25 = t2920+t2927+t3489-t3494+t3722-t3784+t964.*(t105-t465).*3.36554e-3+t977.*(t105-t465).*3.36554e-3+t1430.*(t103-t544).*3.36554e-3+t1512.*(t103-t544).*3.36554e-3;
et26 = t1510.*(t197-t537).*3.372816795e-3+t1505.*(t214-t541).*3.372816795e-3;
t6602 = -t4476.*(et25+et26);
t6611 = t1765+t1798+t1965+t2037+t2045+t2154+t2486+t2584+t2650+t2751+t3155+t3215+t3221+t3261+t3301+t3305+t3327+t3474;
t6612 = t1675+t1874+t1908+t2037+t2154+t2156+t2437+t2546+t2666+t2765+t3183+t3215+t3221+t3299+t3301+t3305+t3319+t3413;
t6613 = t1675+t1765+t1908+t1965+t2220+t2307+t2437+t2486+t2546+t2584+t3155+t3183+t3261+t3319+t3367+t3372+t3454+t3457;
t6614 = t1963+t2066+t2094+t2288+t2550+t2896+t2946+t2949+t2985+t2992+t3037+t3042+t3078+t3515+t3538+t3559+t3588;
t6615 = t2007+t2042+t2118+t2144+t2362+t2547+t2607+t2677+t2740+t2758+t2846+t2893+t2930+t2942+t3271+t3317+t3340+t3388;
t6616 = t1905+t1969+t2190+t2262+t2362+t2407+t2470+t2530+t2547+t2552+t3016+t3049+t3086+t3087+t3271+t3317+t3340+t3388;
t6617 = t1905+t1969+t2007+t2118+t2407+t2470+t2530+t2552+t2560+t2759+t2846+t2893+t2930+t2942+t3440+t3465+t3478+t3513;
t6618 = t1912+t2066+t2151+t2431+t2550+t2804+t2806+t2898+t2938+t2985+t2992+t3051+t3174+t3515+t3588+t3646+t3677;
t6619 = t1912+t1963+t2245+t2288+t2760+t2804+t2806+t2896+t2898+t2938+t3037+t3128+t3135+t3538+t3559+t3603+t3736;
t6620 = t1941+t1973+t2007+t2090+t2489+t2547+t2576+t2743+t2768+t2802+t2930+t2942+t3060+t3103+t3391+t3412+t3414+t3445;
t6621 = t1867+t1930+t2102+t2190+t2489+t2547+t2568+t2632+t2787+t2845+t2918+t2965+t3086+t3087+t3391+t3412+t3414+t3445;
t6622 = t1867+t1930+t1941+t2007+t2568+t2576+t2632+t2715+t2743+t2759+t2918+t2930+t2942+t2965+t3516+t3529+t3541+t3553;
t6623 = t1962+t2171+t2251+t2363+t2463+t2551+t2577+t2630+t2679+t2742+t2976+t2988+t3032+t3075+t3252+t3279+t3313+t3342;
t6624 = t2025+t2150+t2322+t2363+t2392+t2472+t2531+t2551+t2788+t2814+t2832+t2932+t2988+t3032+t3252+t3342+t3443+t3446;
t6625 = t1962+t2025+t2251+t2322+t2472+t2531+t2562+t2577+t2630+t2761+t2832+t2932+t3132+t3163+t3279+t3313+t3357+t3466;
t6630 = t760+t1003+t1416+t1469+t1551+t1587+t1605+t2221+t2766+t3092+t3245+t3492+t3497+t3699+t4093+t4130+t4193+t4194;
t6634 = -t3938.*(t1645+t1965+t2072+t2220-t2242-t2409-t2483-t2504-t3093+t3155+t3261+t3432+t3437-t3442+t1179.*(t103-t544).*3.36554e-3+t3.*t575.*(t105-t465).*3.36554e-3+t8.*t872.*(t534-t546).*3.372816795e-3);
t6635 = t2288+t2290+t2422+t2461+t2671+t2682+t2689+t2705+t2752+t2813+t3017+t3043+t3098+t3112+t3280+t3314+t3517+t3535;
t6636 = t2318+t2320+t2431+t2433+t2476+t2488+t2752+t2813+t2837+t2841+t2872+t2903+t3098+t3112+t3444+t3447+t3517+t3535;
t6637 = t2288+t2290+t2318+t2320+t2476+t2488+t2671+t2682+t2872+t2890+t2903+t2960+t3226+t3241+t3280+t3314+t3605+t3629;
t6638 = -t4173.*(t1799+t1965+t2037-t2064+t2072-t2613-t2696-t2723-t3093+t3155+t3261+t3270-t3276+t3312+t1179.*(t103-t544).*3.36554e-3+t3.*t575.*(t105-t465).*3.372786875e-3+t8.*t872.*(t534-t546).*3.36554e-3);
t6640 = (-t1262+t1701+t9.*t868.*(t105-t465)).*(t1799+t1965+t2037-t2064+t2072-t2613-t2696-t2723-t3093+t3155+t3261+t3270-t3276+t3312+t1179.*(t103-t544).*3.36554e-3+t3.*t575.*(t105-t465).*3.372786875e-3+t8.*t872.*(t534-t546).*3.36554e-3);
t6641 = -t4162.*(t1645+t2037-t2064+t2156+t2227-t2409-t2483-t2504-t3244+t3270-t3276+t3299+t3312+t3413+t1179.*(t103-t544).*3.367829185e-3+t3.*t575.*(t105-t465).*3.36554e-3+t8.*t872.*(t534-t546).*3.36554e-3);
t6642 = t1723+t1820+t1931+t1998+t2340+t2600+t2797+t2859+t2860+t2936+t3147+t3153+t3196+t3232+t3760+t3761+t3873+t3903;
t6643 = t1820+t1841+t1998+t2091+t2181+t2401+t2797+t2860+t3004+t3076+t3196+t3232+t3278+t3285+t3610+t3611+t3819+t3837;
t6644 = t1723+t1916+t1931+t2181+t2182+t2401+t2859+t2936+t2962+t3031+t3147+t3153+t3338+t3387+t3610+t3611+t3819+t3837;
t6645 = (-t947+t1240.*(t105-t465)+t903.*(t534-t546)).*(t1799+t1965+t2037-t2064+t2072-t2613-t2696-t2723-t3093+t3155+t3261+t3270-t3276+t3312+t1179.*(t103-t544).*3.36554e-3+t3.*t575.*(t105-t465).*3.372786875e-3+t8.*t872.*(t534-t546).*3.36554e-3);
t6646 = -t4277.*(t1645+t2037-t2064+t2156+t2227-t2409-t2483-t2504-t3244+t3270-t3276+t3299+t3312+t3413+t1179.*(t103-t544).*3.367829185e-3+t3.*t575.*(t105-t465).*3.36554e-3+t8.*t872.*(t534-t546).*3.36554e-3);
t6647 = t4277.*(t1645+t2037-t2064+t2156+t2227-t2409-t2483-t2504-t3244+t3270-t3276+t3299+t3312+t3413+t1179.*(t103-t544).*3.367829185e-3+t3.*t575.*(t105-t465).*3.36554e-3+t8.*t872.*(t534-t546).*3.36554e-3);
t6653 = -t4313.*(t1645+t2037-t2064+t2156+t2227-t2409-t2483-t2504-t3244+t3270-t3276+t3299+t3312+t3413+t1179.*(t103-t544).*3.367829185e-3+t3.*t575.*(t105-t465).*3.36554e-3+t8.*t872.*(t534-t546).*3.36554e-3);
t6656 = t848+t906+t1630+t1636+t1669+t1679+t1740+t1802+t2665+t2725+t3618+t3620+t3682+t3684+t4229+t4230+t4245+t4247;
t6669 = (t1332+t2368+t1512.*(t105-t465)).*(t1799+t1965+t2037-t2064+t2072-t2613-t2696-t2723-t3093+t3155+t3261+t3270-t3276+t3312+t1179.*(t103-t544).*3.36554e-3+t3.*t575.*(t105-t465).*3.372786875e-3+t8.*t872.*(t534-t546).*3.36554e-3);
t6672 = -t4392.*(t1645+t1965+t2072+t2220-t2242-t2409-t2483-t2504-t3093+t3155+t3261+t3432+t3437-t3442+t1179.*(t103-t544).*3.36554e-3+t3.*t575.*(t105-t465).*3.36554e-3+t8.*t872.*(t534-t546).*3.372816795e-3);
t6673 = t4392.*(t1645+t1965+t2072+t2220-t2242-t2409-t2483-t2504-t3093+t3155+t3261+t3432+t3437-t3442+t1179.*(t103-t544).*3.36554e-3+t3.*t575.*(t105-t465).*3.36554e-3+t8.*t872.*(t534-t546).*3.372816795e-3);
t6677 = -t4447.*(t1645+t1965+t2072+t2220-t2242-t2409-t2483-t2504-t3093+t3155+t3261+t3432+t3437-t3442+t1179.*(t103-t544).*3.36554e-3+t3.*t575.*(t105-t465).*3.36554e-3+t8.*t872.*(t534-t546).*3.372816795e-3);
t6681 = t3938.*(t1867-t1907-t1915+t2007+t2568+t2576+t2632+t2715+t2743+t2759+t2918+t2930+t2942+t2965+t3516+t3529+t3541+t3553);
t6699 = -t4476.*(t1645+t1965+t2072+t2220-t2242-t2409-t2483-t2504-t3093+t3155+t3261+t3432+t3437-t3442+t1179.*(t103-t544).*3.36554e-3+t3.*t575.*(t105-t465).*3.36554e-3+t8.*t872.*(t534-t546).*3.372816795e-3);
t6709 = t4162.*(t1867-t1907-t2067+t2190+t2489+t2547+t2568+t2632+t2787+t2845+t2918+t2965+t3086+t3087+t3391+t3412+t3414+t3445);
t6729 = t4313.*(t1867-t1907-t2067+t2190+t2489+t2547+t2568+t2632+t2787+t2845+t2918+t2965+t3086+t3087+t3391+t3412+t3414+t3445);
t6739 = t4392.*(t1867-t1907-t1915+t2007+t2568+t2576+t2632+t2715+t2743+t2759+t2918+t2930+t2942+t2965+t3516+t3529+t3541+t3553);
t6743 = -(-t1331+t2317+t1510.*(t103-t544)).*(t1867-t1907-t2067+t2190+t2489+t2547+t2568+t2632+t2787+t2845+t2918+t2965+t3086+t3087+t3391+t3412+t3414+t3445);
t6745 = t4408.*(t1867-t1907-t1915+t2007+t2568+t2576+t2632+t2715+t2743+t2759+t2918+t2930+t2942+t2965+t3516+t3529+t3541+t3553);
t6754 = -t3938.*(t1692+t1786+t1910+t1964+t2305-t2600-t2797-t2860-t2936-t3147+t3167-t3232+t3720+t3721-t3903+t1430.*(t539+t641).*3.372816795e-3+t1181.*(t105-t465).*3.36554e-3+t11.*t381.*(t534-t546).*3.36554e-3);
t6755 = t4447.*(t1867-t1907-t1915+t2007+t2568+t2576+t2632+t2715+t2743+t2759+t2918+t2930+t2942+t2965+t3516+t3529+t3541+t3553);
t6756 = -t3961.*(t1786+t1810+t1964+t2047+t2152-t2401-t2797-t2860-t3076+t3167-t3232-t3278+t3582+t3583-t3837+t1430.*(t539+t641).*3.36554e-3+t1181.*(t105-t465).*3.372786875e-3+t11.*t381.*(t534-t546).*3.372786875e-3);
